simulink model "RB_KAIROS_ArmOnly"  (R2020b)
(part 5 of 17)

t11502 = (t10964.*(t263-t283-t310+t1265))./4.0;
t11506 = (t11023.*(t943-t1091))./4.0;
t11513 = (t3424.*t11023)./4.0;
t11514 = (t6158.*t10141)./4.0;
t11524 = (t6763.*t9828)./4.0;
t11527 = t14.*t6430.*t9828.*8.9697375e-1;
t11530 = -t11523;
t11536 = (t7797.*t9233)./4.0;
t11540 = t14.*t9828.*(t4540+t5.*(t2425-t2468)).*(-8.9697375e-1);
t11562 = t10141.*(-t2149+t2205+t693.*(t48-t349)+t784.*(t48-t349)).*(-1.0./2.0);
t11579 = ((t1492+t2158+t2696-t4727).*(-t3045-t3218+t3458+t3539+t3878+t8.*(t260+t468+t570+t2298).*1.666555))./2.0;
t11624 = t5235.*(t16.*(t30.*(t2425-t2468)+t68.*(t2425-t2468)).*1.666555+t8.*(t7.*(t4650+t34.*(t2425-t2468))+t47.*(t2425-t2468)).*1.666555).*(-1.0./4.0);
t11629 = (t5235.*(t16.*(t30.*(t2425-t2468)+t68.*(t2425-t2468)).*1.666555+t8.*(t7.*(t4650+t34.*(t2425-t2468))+t47.*(t2425-t2468)).*1.666555))./4.0;
t11645 = t10141.*(t624+t2511-t3502-t9.*t439.*4.252e-3).*(-1.0./2.0);
t11655 = (t4252.*t10964)./4.0;
t11657 = (t4251.*t10966)./4.0;
t11658 = t8.*t11633;
t11659 = t9.*t11633;
t11660 = t16.*t11633;
t11661 = t17.*t11633;
t11701 = t15.*t9236.*(t4542-t6448).*(-1.0./4.0);
t11713 = -t11709;
t11714 = (t15.*t9236.*(t6460-t35.*(t2425-t2468)))./4.0;
t11715 = t9263.*(t4542-t6448).*(-1.0./4.0);
t11738 = (t8213.*t9236)./4.0;
t11746 = t15.*t9278.*(t4542-t6448).*(-1.0./4.0);
t11747 = t8166.*(t1786+t2973-t7703-t5.*t12.*3.746479959e-1).*(-1.0./4.0);
t11753 = (t4569.*t10964)./4.0;
t11755 = (t15.*t9278.*(t4542-t6448))./4.0;
t11763 = (t4604.*t10966)./4.0;
t11764 = (t7247.*t9828)./4.0;
t11774 = (t7259.*t9830)./4.0;
t11776 = -t11767;
t11778 = ((t4542-t6448).*(t5457-t7520))./4.0;
t11780 = ((t4542-t6448).*(t5454-t7513))./4.0;
t11784 = t9236.*(t4654+t15.*(t4650+t34.*(t2425-t2468))).*(-1.0./4.0);
t11786 = t9269.*(-t1476-t1540+t2091+t2165+t2579+t8.*(t260+t468+t570+t2298)).*(-1.0./2.0);
t11787 = (t9236.*(t4654+t15.*(t4650+t34.*(t2425-t2468))))./4.0;
t11792 = t7434.*(-t3045-t3218+t3458+t3539+t3878+t8.*(t260+t468+t570+t2298).*1.666555).*(-1.0./2.0);
t11796 = t9828.*(t30.*(t2425-t2468).*3.587895+t68.*(t2425-t2468).*3.587895).*(-1.0./4.0);
t11797 = (t8191.*t9310)./2.0;
t11805 = (t8166.*t9325)./4.0;
t11808 = (t9828.*(t30.*(t2425-t2468).*3.587895+t68.*(t2425-t2468).*3.587895))./4.0;
t11818 = -t11809;
t11824 = t4884.*(t8963+t7.*(t5026+t5.*(t2959-t2967))).*(-1.0./4.0);
t11826 = (t6196.*t10441)./4.0;
t11829 = (t4884.*(t8963+t7.*(t5026+t5.*(t2959-t2967))))./4.0;
t11868 = (t6092.*t10501)./4.0;
t11871 = t8.*t11855;
t11905 = (t5713.*t10769)./4.0;
t11934 = (t7130.*t10141)./2.0;
t11937 = t7728+t9891;
t11947 = t10501.*(t985+t3399-t13.*t42.*1.01140545e-1-t7.*t223.*5.034347249e-2).*(-1.0./4.0);
t12016 = t5443.*(t8963+t7.*(t5026+t5.*(t2959-t2967))).*(-1.0./4.0);
t12021 = (t5443.*(t8963+t7.*(t5026+t5.*(t2959-t2967))))./4.0;
t12028 = (t8711.*t9285)./4.0;
t12030 = (t6302.*(t8643-t8.*(t30.*(t2425-t2468)+t68.*(t2425-t2468)).*7.35522e-1))./4.0;
t12034 = (t6190.*t10769)./4.0;
t12038 = (t4884.*t11266)./4.0;
t12042 = t2910+t2981+t3181+t3294+t3631+t5828+t7998;
t12050 = t2957+t3123+t3130+t3291+t3628+t5827+t8016;
t12072 = t14.*t6430.*t10501.*3.064865e-1;
t12077 = (t8711.*t9499)./4.0;
t12079 = t14.*t10501.*(t4540+t5.*(t2425-t2468)).*(-3.064865e-1);
t12083 = t6190.*(-t1053-t3327+t5081.*1.225946+t7731+t15.*t223.*1.4653732538e-2).*(-1.0./4.0);
t12084 = t14.*t10501.*(t4540+t5.*(t2425-t2468)).*3.064865e-1;
t12097 = (t6928.*t10501)./4.0;
t12100 = (t6175.*t10850)./4.0;
t12106 = (t6196.*t10858)./4.0;
t12150 = (t8437.*t9884)./4.0;
t12181 = t6196.*(t8963+t7.*(t5026+t5.*(t2959-t2967))).*(-1.0./4.0);
t12188 = (t6196.*(t8963+t7.*(t5026+t5.*(t2959-t2967))))./4.0;
t12191 = t10094.*(t4542-t6448).*(-1.0./4.0);
t12194 = (t10094.*(t4542-t6448))./4.0;
t12196 = (t5443.*t11266)./4.0;
t12197 = (t10094.*(t6460-t35.*(t2425-t2468)))./4.0;
t12211 = (t8166.*(-t1785+t2869+t2960+t5489+t5720+t4.*t13.*3.746479959e-1))./4.0;
t12217 = (t7245.*t10501)./2.0;
t12218 = (t7245.*t10501)./4.0;
t12228 = (t7246.*t10501)./4.0;
t12243 = (t6190.*t11023)./4.0;
t12249 = (t3266.*t11907)./4.0;
t12251 = t10501.*(t30.*(t2425-t2468).*1.225946+t68.*(t2425-t2468).*1.225946).*(-1.0./4.0);
t12260 = (t10501.*(t30.*(t2425-t2468).*1.225946+t68.*(t2425-t2468).*1.225946))./4.0;
t12266 = t2684+t2687+t11633;
t12269 = (t3362.*t11907)./4.0;
t12272 = (t11907.*(t923-t1076))./4.0;
t12297 = (t6.*t6430.*t10964)./4.0;
t12299 = (t6442.*t10966)./4.0;
t12302 = (t14.*t6430.*t10966)./4.0;
t12309 = t6.*t10964.*(t4540+t5.*(t2425-t2468)).*(-1.0./4.0);
t12313 = t14.*t10966.*(t4540+t5.*(t2425-t2468)).*(-1.0./4.0);
t12316 = (t6455.*t10964)./4.0;
t12317 = (t8711.*t9884)./4.0;
t12327 = t10966.*(t30.*(t2425-t2468)+t68.*(t2425-t2468)).*(-1.0./4.0);
t12335 = (t10966.*(t30.*(t2425-t2468)+t68.*(t2425-t2468)))./4.0;
t12343 = t10964.*(t4650+t34.*(t2425-t2468)).*(-1.0./4.0);
t12348 = (t10964.*(t4650+t34.*(t2425-t2468)))./4.0;
t12362 = t7.*t12049.*1.059103943995e-1;
t12366 = t15.*t12053.*1.059103943995e-1;
t12374 = (t8433.*t10141)./4.0;
t12377 = (t4884.*t11720)./4.0;
t12378 = t7.*t12163.*8.639075e-2;
t12380 = (t4265.*t11907)./4.0;
t12387 = t7677+t10566;
t12406 = (t8054.*t10441)./4.0;
t12418 = (t8628.*t10141)./4.0;
t12419 = (t8191.*t10398)./4.0;
t12454 = (t4774.*t11907)./4.0;
t12464 = t1313+t3488+t3541+t3612+t3867+t3922+t5822+t8013;
t12483 = (t5443.*t11720)./4.0;
t12486 = t12407.*(-7.35522e-1);
t12489 = t12407.*7.35522e-1;
t12528 = (t8438.*t10501)./4.0;
t12531 = (t9263.*t9828)./2.0;
t12535 = (t5277.*t11907)./4.0;
t12544 = ((t16.*(t30.*(t2425-t2468)+t68.*(t2425-t2468)).*1.666555+t8.*(t7.*(t4650+t34.*(t2425-t2468))+t47.*(t2425-t2468)).*1.666555).*(-t1476-t1540+t2091+t2165+t2579+t8.*(t260+t468+t570+t2298)))./4.0;
t12547 = t10759.*(t4542-t6448).*(-1.0./4.0);
t12548 = (t9325.*t9830)./2.0;
t12549 = (t10759.*(t4542-t6448))./4.0;
t12550 = t9828.*(t5454-t7513).*(-1.0./2.0);
t12552 = t10769.*(t4542-t6448).*(-1.0./4.0);
t12554 = (t9828.*(t5454-t7513))./2.0;
t12555 = (t10769.*(t4542-t6448))./4.0;
t12557 = (t8166.*t10754)./4.0;
t12558 = -t12553;
t12559 = (t10769.*(t6460-t35.*(t2425-t2468)))./4.0;
t12565 = (t8609.*t10501)./4.0;
t12568 = t12407.*(-3.867742437e-3);
t12573 = t15.*t12385.*1.059103943995e-1;
t12579 = t12407.*3.867742437e-3;
t12588 = t3188+t3333+t3627+t7833+t9323;
t12589 = t3125+t3336+t3630+t7835+t9331;
t12590 = t7.*t12396.*1.059103943995e-1;
t12593 = ((t4542-t6448).*(-t1053-t3327+t5081.*1.225946+t7731+t15.*t223.*1.4653732538e-2))./4.0;
t12601 = (t8689.*t10501)./4.0;
t12603 = (t5583.*t11907)./2.0;
t12604 = (t5583.*t11907)./4.0;
t12627 = (t5716.*t11907)./4.0;
t12654 = t8054.*(t8963+t7.*(t5026+t5.*(t2959-t2967))).*(-1.0./4.0);
t12664 = (t8054.*(t8963+t7.*(t5026+t5.*(t2959-t2967))))./4.0;
t12667 = t1267+t1955+t2202+t2562+t7690+t9892;
t12687 = (t5884.*t11907)./4.0;
t12711 = t10964.*(t4542-t6448).*(-1.0./4.0);
t12712 = t10966.*(t4542-t6448).*(-1.0./4.0);
t12715 = (t10966.*(t4542-t6448))./4.0;
t12718 = (t10964.*(t6460-t35.*(t2425-t2468)))./4.0;
t12719 = (t10966.*(t6460-t35.*(t2425-t2468)))./4.0;
t12725 = (t8166.*t10964)./4.0;
t12727 = (t8166.*t10966)./4.0;
t12730 = t8256.*(t8963+t7.*(t5026+t5.*(t2959-t2967))).*(-1.0./4.0);
t12734 = t11023.*(t4542-t6448).*(-1.0./4.0);
t12735 = (t8256.*(t8963+t7.*(t5026+t5.*(t2959-t2967))))./4.0;
t12737 = (t11023.*(t4542-t6448))./4.0;
t12740 = (t11023.*(t6460-t35.*(t2425-t2468)))./4.0;
t12749 = (t6114.*t11907)./4.0;
t12751 = t10964.*(t263+t1265-t7252-t5.*t12.*1.0442e-1).*(-1.0./2.0);
t12752 = (t8272.*t10966)./2.0;
t12756 = (t10964.*(t263+t1265-t7252-t5.*t12.*1.0442e-1))./2.0;
t12796 = t3182+t3565+t3934+t11848;
t12832 = (t14.*t6430.*t11907)./4.0;
t12836 = (t6442.*t11907)./4.0;
t12842 = t14.*t11907.*(t4540+t5.*(t2425-t2468)).*(-1.0./4.0);
t12844 = (t9236.*t10441)./4.0;
t12845 = (t14.*t11907.*(t4540+t5.*(t2425-t2468)))./4.0;
t12859 = t11907.*(t30.*(t2425-t2468)+t68.*(t2425-t2468)).*(-1.0./4.0);
t12865 = (t11907.*(t30.*(t2425-t2468)+t68.*(t2425-t2468)))./4.0;
t12866 = t206+t446+t2571+t2622+t2736+t2770+t11671;
t12887 = (t5634.*t12163)./4.0;
t12890 = (t6175.*t12049)./4.0;
t12898 = t1315+t3619+t3932+t3973+t7832+t9327;
t12900 = (t6196.*t12053)./4.0;
t12914 = -t12911;
t12916 = (t10964.*(-t262+t1056+t1250+t5078+t5282+t4.*t13.*1.0442e-1))./2.0;
t12917 = (t9828.*t10094)./2.0;
t12919 = -t12915;
t12924 = (t8697.*t10966)./2.0;
t12926 = (t8256.*t11266)./4.0;
t12939 = (t5216.*t12385)./4.0;
t12948 = t10501.*(t5457-t7520).*(-1.0./2.0);
t12955 = (t5218.*t12396)./4.0;
t12996 = ((t16.*(t30.*(t2425-t2468)+t68.*(t2425-t2468))+t8.*(t7.*(t4650+t34.*(t2425-t2468))+t47.*(t2425-t2468))).*(-t3045-t3218+t3458+t3539+t3878+t8.*(t260+t468+t570+t2298).*1.666555))./4.0;
t13011 = (t8931.*t10964)./2.0;
t13018 = t10966.*(t5027-t7134).*(-1.0./2.0);
t13023 = (t10966.*(t5027-t7134))./2.0;
t13060 = (t5635.*t12385)./4.0;
t13083 = (t5646.*t12396)./4.0;
t13137 = (t9236.*t10858)./4.0;
t13150 = t232+t429+t2506+t2524+t3657+t3669+t7690+t9892;
t13163 = (t6046.*t12392)./4.0;
t13169 = (t4024.*t12792)./4.0;
t13183 = t9278.*(t8963+t7.*(t5026+t5.*(t2959-t2967))).*(-1.0./4.0);
t13187 = (t9278.*(t8963+t7.*(t5026+t5.*(t2959-t2967))))./4.0;
t13191 = -t13190;
t13199 = (t12163.*(t921+t1317-t5853))./4.0;
t13215 = (t7039.*t12185)./4.0;
t13219 = t16.*t13019.*4.38178973375e-3;
t13236 = t7.*t13140.*8.639075e-2;
t13248 = (t9828.*t10759)./2.0;
t13262 = (t6552.*t12385)./4.0;
t13264 = t11907.*(t4542-t6448).*(-1.0./4.0);
t13268 = (t11907.*(t4542-t6448))./4.0;
t13271 = (t11907.*(t6460-t35.*(t2425-t2468)))./4.0;
t13275 = (t6546.*t12396)./4.0;
t13281 = (t8166.*t11907)./4.0;
t13311 = (t9236.*t11247)./4.0;
t13340 = (t5235.*t12792)./4.0;
t13341 = (t9685.*t10964)./2.0;
t13351 = (t2980.*t13140)./4.0;
t13353 = (t9686.*t10966)./2.0;
t13358 = (t8050.*t12049)./4.0;
t13365 = (t8054.*t12053)./4.0;
t13396 = (t7113.*t12385)./4.0;
t13406 = (t7124.*t12396)./4.0;
t13446 = (t4064.*t13140)./4.0;
t13545 = t11907.*(t5027-t7134).*(-1.0./2.0);
t13578 = t1604+t2211+t3880+t3884+t3988+t4006+t11862;
t13588 = (t4837.*t13140)./4.0;
t13592 = t7797.*(t8329+t17.*(t16.*(t30.*(t2425-t2468)+t68.*(t2425-t2468))+t8.*(t7.*(t4650+t34.*(t2425-t2468))+t47.*(t2425-t2468)))).*(-1.0./4.0);
t13595 = (t7797.*(t8329+t17.*(t16.*(t30.*(t2425-t2468)+t68.*(t2425-t2468))+t8.*(t7.*(t4650+t34.*(t2425-t2468))+t47.*(t2425-t2468)))))./4.0;
t13604 = (t9278.*t11720)./4.0;
t13605 = (t921+t1317-t5853).*(t3129+t3384+t3574+t7846+t9332).*(-1.0./4.0);
t13606 = t12385.*(t2437+t2648+t3129+t3384+t3574).*(-1.0./4.0);
t13617 = (t10501.*t10769)./2.0;
t13629 = t3098+t3211+t3241+t3678+t8102+t10798;
t13630 = (t5095.*t13140)./4.0;
t13631 = (t8047.*t12385)./4.0;
t13633 = (t8044.*t12385)./4.0;
t13636 = (t8053.*t12396)./4.0;
t13637 = (t8065.*t12396)./4.0;
t13650 = t10501.*(-t1053-t3327+t5081.*1.225946+t7731+t15.*t223.*1.4653732538e-2).*(-1.0./2.0);
t13651 = (t10501.*(-t1053-t3327+t5081.*1.225946+t7731+t15.*t223.*1.4653732538e-2))./2.0;
t13664 = (t8285.*t12385)./4.0;
t13689 = (t8310.*t12396)./4.0;
t13706 = (t9285.*t11907)./2.0;
t13732 = (t6069.*t13019)./4.0;
t13738 = t16.*(t3098+t3211-t3221+t3678+t8102+t10798).*2.62925e-3;
t13739 = t7.*t12385.*(t4542-t6448).*(-3.064865e-1);
t13745 = t7.*t12385.*(t4542-t6448).*3.064865e-1;
t13748 = t7.*t12385.*(t6460-t35.*(t2425-t2468)).*3.064865e-1;
t13749 = (t5648.*t13140)./4.0;
t13755 = t15.*t12396.*(t4542-t6448).*(-3.064865e-1);
t13758 = t15.*t12396.*(t6460-t35.*(t2425-t2468)).*3.064865e-1;
t13774 = (t9499.*t11907)./2.0;
t13775 = (t10501.*t11023)./2.0;
t13828 = (t13313.*(t2904-t2927))./4.0;
t13833 = (t9236.*t12053)./4.0;
t13834 = (t5853.*t13140)./4.0;
t13837 = (t5860.*t13140)./4.0;
t13848 = (t5999.*t13140)./4.0;
t13875 = t12396.*(t5150-t6911).*(-1.0./4.0);
t13882 = t12385.*(t7.*(t4650+t34.*(t2425-t2468)).*1.225946+t47.*(t2425-t2468).*1.225946).*(-1.0./4.0);
t13884 = (t12385.*(t7.*(t4650+t34.*(t2425-t2468)).*1.225946+t47.*(t2425-t2468).*1.225946))./4.0;
t13887 = (t8922.*t12396)./4.0;
t13891 = (t5365.*t13313)./4.0;
t13941 = (t9884.*t11907)./2.0;
t13964 = (t4021.*(t3098+t3211-t3221+t3678+t8102+t10798))./4.0;
t14015 = (t9209.*t12385)./4.0;
t14018 = (t6988.*t13140)./4.0;
t14023 = t12792.*(-t1476-t1540+t2091+t2165+t2579+t8.*(t260+t468+t570+t2298)).*(-1.0./4.0);
t14035 = t1566+t1867+t3700+t3703+t4023+t4038+t8101+t10794;
t14107 = t12392.*(-t3045-t3218+t3458+t3539+t3878+t8.*(t260+t468+t570+t2298).*1.666555).*(-1.0./4.0);
t14155 = t15.*t13140.*(t4542-t6448).*(-1.0./4.0);
t14162 = (t15.*t13140.*(t6460-t35.*(t2425-t2468)))./4.0;
t14164 = (t8213.*t13140)./4.0;
t14180 = t13140.*(t4654+t15.*(t4650+t34.*(t2425-t2468))).*(-1.0./4.0);
t14182 = (t13140.*(t4654+t15.*(t4650+t34.*(t2425-t2468))))./4.0;
t14304 = (t8477.*t13313)./4.0;
t14670 = (t10441.*t13140)./2.0;
t14710 = (t10141.*t13313)./4.0;
t14801 = (t10858.*t13140)./2.0;
t14821 = t1763+t1824+t2316+t2415+t2791+t10569+t12397;
t14823 = t1791+t1818+t2335+t2387+t2789+t10567+t12407;
t14845 = t13140.*(t8963+t7.*(t5026+t5.*(t2959-t2967))).*(-1.0./2.0);
t14858 = (t12163.*t12385)./2.0;
t14865 = (t12185.*t12396)./2.0;
t14914 = (t11247.*t13140)./2.0;
t15037 = t12385.*(t3129+t3384+t3574+t7846+t9332).*(-1.0./2.0);
t15040 = (t12385.*(t3129+t3384+t3574+t7846+t9332))./2.0;
t15142 = (t12053.*t13140)./2.0;
t1967 = -t1918;
t2474 = t9.*t2405;
t2480 = t17.*t2405;
t3308 = t543+t1912;
t3392 = t1918.*(-1.2516e-2);
t3448 = t1912.*6.1597e-2;
t3452 = t1918.*6.1597e-2;
t3569 = t1918.*(-4.28e-4);
t3572 = t1918.*(-1.0517e-2);
t3652 = t1918.*(-7.41e-4);
t3845 = t2549.*(-7.35522e-1);
t3893 = t2549.*7.35522e-1;
t4321 = t1912.*4.5305948634e-2;
t4324 = t1918.*4.5305948634e-2;
t4346 = t1912.*3.127439544e-3;
t4349 = t1918.*3.127439544e-3;
t4350 = t1912.*7.735484874e-3;
t4355 = t1918.*7.735484874e-3;
t4666 = t2549.*(-3.127439544e-3);
t4713 = -t4682;
t4769 = -t4744;
t4814 = -t4771;
t4826 = -t4808;
t4956 = -t4947;
t4980 = t1918.*1.672482661783778e-3;
t4981 = t1912.*5.48359106408232e-4;
t5111 = t4528.*7.35522e-1;
t5113 = t4529.*7.35522e-1;
t5127 = -t5106;
t5147 = -t5128;
t5166 = -t5140;
t5184 = -t5160;
t5199 = t4697.*7.35522e-1;
t5220 = t4693.*7.35522e-1;
t5226 = -t5205;
t5236 = t3239.*(t1918+t9.*(t71-t391)).*(-1.0./4.0);
t5238 = t3324.*(t689-t740).*(-1.0./4.0);
t5242 = (t3239.*(t1918+t9.*(t71-t391)))./4.0;
t5243 = t4771.*7.35522e-1;
t5245 = (t3324.*(t689-t740))./4.0;
t5250 = t3280.*(t1918+t9.*(t71-t391)).*(-1.0./4.0);
t5255 = t4767.*7.35522e-1;
t5260 = (t3280.*(t1918+t9.*(t71-t391)))./4.0;
t5296 = t3447.*(t1918+t9.*(t71-t391)).*(-1.0./4.0);
t5305 = (t3447.*(t1918+t9.*(t71-t391)))./4.0;
t5325 = -t5315;
t5343 = -t5332;
t5348 = -t5338;
t5353 = -t5342;
t5359 = t9.*t5337;
t5360 = t17.*t5337;
t5384 = t9.*t5357;
t5386 = t17.*t5357;
t5395 = -t9.*(t1474+t4743);
t5396 = -t17.*(t1474+t4743);
t5415 = t17.*(t1474+t4743);
t5417 = -t5409;
t5558 = t4529.*3.867742437e-3;
t5567 = -t5549;
t5570 = t4528.*1.563719772e-3;
t5607 = -t5584;
t5608 = -t5585;
t5633 = -t5618;
t5643 = t4693.*3.867742437e-3;
t5658 = t4697.*1.563719772e-3;
t5664 = -t5651;
t5676 = -t5662;
t5684 = -t5673;
t5685 = -t5675;
t5687 = t4771.*3.867742437e-3;
t5698 = t4767.*1.563719772e-3;
t5700 = -t5686;
t5727 = -t5717;
t5752 = -t5738;
t5766 = t4410.*(t1918+t9.*(t71-t391)).*(-1.0./4.0);
t5770 = -t5754;
t5773 = (t4410.*(t1918+t9.*(t71-t391)))./4.0;
t5775 = -t5768;
t5789 = (t3324.*t4515)./4.0;
t5801 = t4499.*(t1918+t9.*(t71-t391)).*(-1.0./4.0);
t5805 = -t5792;
t5814 = (t4499.*(t1918+t9.*(t71-t391)))./4.0;
t5820 = t9.*(t1474+t4743).*(-7.35522e-1);
t5882 = -t5871;
t5893 = t4701.*(t1918+t9.*(t71-t391)).*(-1.0./4.0);
t5908 = (t4701.*(t1918+t9.*(t71-t391)))./4.0;
t6011 = -t5994;
t6204 = t8.*t5234.*4.38178973375e-3;
t6218 = -t6206;
t6251 = t2041+t2102+t2636+t2643;
t6341 = (t8.*t6250)./4.0;
t6378 = (t15.*t16.*t6250)./4.0;
t6380 = (t16.*t6271)./4.0;
t6384 = t9.*(t1474+t4743).*(-1.563719772e-3);
t6389 = -t6370;
t6394 = -t6375;
t6402 = t9.*(t1474+t4743).*1.563719772e-3;
t6405 = (t8.*t15.*t6271)./4.0;
t6465 = -t6457;
t6480 = (t227.*t6271)./4.0;
t6482 = (t323.*t6250)./4.0;
t6486 = t5291.*(t1918+t9.*(t71-t391)).*(-1.0./4.0);
t6488 = t8.*t5915.*2.62925e-3;
t6493 = (t5291.*(t1918+t9.*(t71-t391)))./4.0;
t6496 = -t6489;
t6541 = -t6528;
t6568 = -t6559;
t6572 = (t439.*t6250)./4.0;
t6603 = -t6595;
t6608 = t6271.*(t48-t349).*(-1.0./4.0);
t6618 = (t6271.*(t48-t349))./4.0;
t6623 = t17.*t5719.*1.13264871585e-2;
t6640 = -t6630;
t6664 = -t6652;
t6668 = -t6660;
t6688 = -t6680;
t6696 = t5553.*(t1918+t9.*(t71-t391)).*(-1.0./4.0);
t6707 = -t6691;
t6712 = -t6692;
t6717 = (t5553.*(t1918+t9.*(t71-t391)))./4.0;
t6719 = (t15.*t16.*t6634)./4.0;
t6721 = -t6701;
t6725 = -t6708;
t6731 = -t6714;
t6740 = t5609.*(t1918+t9.*(t71-t391)).*(-1.0./4.0);
t6744 = t1999+t2168+t2188+t4511;
t6751 = -t6738;
t6769 = -t6757;
t6775 = -t6768;
t6782 = -t6771;
t6787 = t6.*t6757;
t6792 = -t6779;
t6811 = t1067+t1659+t5719;
t6812 = -t6786;
t6867 = -t6829;
t6875 = (t1840.*t6271)./2.0;
t6878 = t6250.*(t348-t525).*(-1.0./2.0);
t6884 = t2943+t5915;
t6887 = -t6853;
t6891 = -t6865;
t6899 = -t6874;
t6901 = (t6250.*(t348-t525))./2.0;
t6903 = -t6880;
t6904 = -t6882;
t6914 = -t6888;
t6925 = -t6896;
t6933 = -t6905;
t6938 = t2017+t2639+t5337;
t6940 = (t323.*t6634)./4.0;
t6947 = -t6922;
t6954 = -t6929;
t6963 = -t6943;
t6964 = t5763.*(t1918+t9.*(t71-t391)).*(-1.0./4.0);
t6968 = -t6953;
t6980 = (t5763.*(t1918+t9.*(t71-t391)))./4.0;
t6990 = (t17.*t6844)./2.0;
t6996 = (t8.*t6893)./4.0;
t7006 = (t3324.*t5837)./4.0;
t7011 = (t9.*t16.*t6844)./4.0;
t7017 = -t7000;
t7021 = -t7005;
t7027 = (t15.*t16.*t6893)./4.0;
t7032 = -t7012;
t7035 = -t7014;
t7046 = t5834.*(t1918+t9.*(t71-t391)).*(-1.0./4.0);
t7058 = (t5834.*(t1918+t9.*(t71-t391)))./4.0;
t7067 = (t439.*t6634)./2.0;
t7078 = (t9.*t7003)./2.0;
t7101 = -t7091;
t7103 = (t16.*t17.*t7003)./4.0;
t7125 = t17.*(t1912.*(-4.28e-4)+t3337+t587.*(t71-t391)+t689.*(t71-t391)).*(-1.0./4.0);
t7128 = t2676+t2706+t3473+t3497;
t7135 = (t17.*(t1912.*(-4.28e-4)+t3337+t587.*(t71-t391)+t689.*(t71-t391)))./4.0;
t7139 = t9.*t16.*(t1912.*(-4.28e-4)+t3337+t587.*(t71-t391)+t689.*(t71-t391)).*(-1.0./4.0);
t7140 = (t325.*t6844)./4.0;
t7141 = t2693+t2704+t3499+t3587;
t7148 = (t9.*t16.*(t1912.*(-4.28e-4)+t3337+t587.*(t71-t391)+t689.*(t71-t391)))./4.0;
t7158 = t5990.*(t1918+t9.*(t71-t391)).*(-1.0./4.0);
t7160 = (t323.*t6893)./4.0;
t7163 = -t7147;
t7169 = (t5990.*(t1918+t9.*(t71-t391)))./4.0;
t7183 = t6041.*(t1918+t9.*(t71-t391)).*(-1.0./4.0);
t7185 = t9.*(t1912.*(-1.0027e-2)+t2709+t3492+t751.*(t71-t391)).*(-1.0./4.0);
t7189 = (t229.*t7003)./4.0;
t7190 = (t9.*(t1912.*(-1.0027e-2)+t2709+t3492+t751.*(t71-t391)))./4.0;
t7199 = t16.*t17.*(t1912.*(-1.0027e-2)+t2709+t3492+t751.*(t71-t391)).*(-1.0./4.0);
t7207 = (t16.*t17.*(t1912.*(-1.0027e-2)+t2709+t3492+t751.*(t71-t391)))./4.0;
t7232 = (t440.*t6844)./4.0;
t7243 = (t439.*t6893)./4.0;
t7257 = t325.*(t1912.*(-4.28e-4)+t3337+t587.*(t71-t391)+t689.*(t71-t391)).*(-1.0./4.0);
t7269 = (t325.*(t1912.*(-4.28e-4)+t3337+t587.*(t71-t391)+t689.*(t71-t391)))./4.0;
t7285 = (t5069.*t5234)./4.0;
t7299 = -t7286;
t7308 = t229.*(t1912.*(-1.0027e-2)+t2709+t3492+t751.*(t71-t391)).*(-1.0./4.0);
t7322 = -t7300;
t7327 = (t229.*(t1912.*(-1.0027e-2)+t2709+t3492+t751.*(t71-t391)))./4.0;
t7333 = (t4024.*t5915)./4.0;
t7347 = -t7324;
t7353 = t6634.*(t348-t525).*(-1.0./4.0);
t7354 = -t7331;
t7356 = -t7334;
t7370 = t7003.*(t79-t358).*(-1.0./4.0);
t7375 = (t6634.*(t348-t525))./4.0;
t7382 = (t7003.*(t79-t358))./4.0;
t7384 = t6276.*(t1918+t9.*(t71-t391)).*(-1.0./4.0);
t7391 = t845+t1667+t1988+t2498+t4630;
t7397 = t440.*(t1912.*(-4.28e-4)+t3337+t587.*(t71-t391)+t689.*(t71-t391)).*(-1.0./4.0);
t7409 = t16.*t6872.*2.62925e-3;
t7411 = (t440.*(t1912.*(-4.28e-4)+t3337+t587.*(t71-t391)+t689.*(t71-t391)))./4.0;
t7430 = -t7419;
t7438 = t2510+t2628+t2665+t2695+t2735;
t7440 = t1236+t2028+t2063+t2135+t2656+t2666;
t7455 = (t17.*t7396)./4.0;
t7465 = -t7456;
t7467 = ((t79-t358).*(t1912.*(-1.0027e-2)+t2709+t3492+t751.*(t71-t391)))./4.0;
t7471 = (t9.*t16.*t7396)./4.0;
t7480 = -t7473;
t7486 = t1362+t1985+t2170+t2302+t2611+t2692;
t7490 = t2597+t2634+t2703+t2718+t2732;
t7497 = t1813+t1968+t2178+t2279+t2592+t2689;
t7510 = (t15.*t7458)./4.0;
t7525 = -t7514;
t7534 = (t7.*t14.*t7458)./4.0;
t7537 = (t9.*t7469)./4.0;
t7541 = t6893.*(t348-t525).*(-1.0./2.0);
t7549 = t6844.*(t395+t9.*(t48-t349)).*(-1.0./4.0);
t7550 = t6.*t15.*t7458.*(-1.0./4.0);
t7552 = (t8.*t7485)./2.0;
t7556 = (t6893.*(t348-t525))./2.0;
t7565 = (t6844.*(t395+t9.*(t48-t349)))./4.0;
t7566 = (t14.*t43.*t7458)./4.0;
t7570 = (t16.*t17.*t7469)./4.0;
t7575 = -t7557;
t7582 = (t15.*t16.*t7485)./4.0;
t7586 = t8.*t7557;
t7601 = -t7587;
t7611 = (t325.*t7396)./4.0;
t7617 = -t7598;
t7636 = -t7618;
t7640 = (t1907.*t7003)./4.0;
t7654 = t3625+t3660+t5337;
t7689 = (t5234.*t5430)./4.0;
t7691 = (t225.*t7458)./4.0;
t7692 = (t226.*t7458)./4.0;
t7721 = -t7701;
t7722 = -t7702;
t7725 = (t15.*t223.*t7458)./2.0;
t7730 = (t229.*t7469)./4.0;
t7738 = t9.*t6761.*1.13264871585e-2;
t7744 = ((t395+t9.*(t48-t349)).*(t1912.*(-4.28e-4)+t3337+t587.*(t71-t391)+t689.*(t71-t391)))./4.0;
t7757 = -t7747;
t7767 = (t323.*t7485)./4.0;
t7770 = (t2520.*t6872)./4.0;
t7772 = -t7758;
t7773 = -t7759;
t7776 = (t403.*t7458)./2.0;
t7782 = t323.*t7557;
t7785 = t1907.*(t1912.*(-1.0027e-2)+t2709+t3492+t751.*(t71-t391)).*(-1.0./4.0);
t7795 = t6615.*(t1918+t9.*(t71-t391)).*(-1.0./4.0);
t7806 = -t7791;
t7813 = -t7794;
t7814 = (t6615.*(t1918+t9.*(t71-t391)))./4.0;
t7817 = t12.*t7791;
t7818 = -t7803;
t7822 = t266+t464+t555+t1952+t2001+t2288+t2619+t2624;
t7829 = t6629.*(t1918+t9.*(t71-t391)).*(-1.0./4.0);
t7843 = (t6629.*(t1918+t9.*(t71-t391)))./4.0;
t7849 = (t454.*t7458)./2.0;
t7856 = t2490+t2746+t2962+t3127+t3346;
t7870 = t8.*t6957.*4.38178973375e-3;
t7872 = (t470.*t7458)./2.0;
t7878 = (t3324.*t6687)./4.0;
t7890 = (t439.*t7485)./4.0;
t7897 = -t7877;
t7912 = -t7900;
t7913 = t2462+t2899+t2971+t3056+t3506;
t7916 = -t7905;
t7933 = -t7920;
t7934 = -t7922;
t7948 = -t7936;
t7961 = -t7947;
t7969 = t6758.*(t1918+t9.*(t71-t391)).*(-1.0./4.0);
t7981 = (t6758.*(t1918+t9.*(t71-t391)))./4.0;
t7993 = t8.*t7079.*4.38178973375e-3;
t7994 = -t7984;
t8010 = t8.*t7105.*4.38178973375e-3;
t8028 = t16.*t7116.*4.38178973375e-3;
t8063 = t141+t234+t602+t1995+t2020+t2573+t2659+t3348;
t8071 = (t4884.*t6193)./4.0;
t8076 = -t8059;
t8099 = -t8080;
t8122 = t6983.*(t1918+t9.*(t71-t391)).*(-1.0./4.0);
t8123 = t7396.*(t395+t9.*(t48-t349)).*(-1.0./2.0);
t8128 = t7.*t8077;
t8129 = t8.*t8077;
t8131 = t15.*t8077;
t8132 = t16.*t8077;
t8133 = -t8115;
t8135 = t7003.*(t1918+t9.*(t71-t391)).*(-1.0./2.0);
t8138 = -t8121;
t8139 = (t6983.*(t1918+t9.*(t71-t391)))./4.0;
t8151 = -t8136;
t8168 = (t5234.*t5919)./2.0;
t8179 = (t5234.*t5914)./2.0;
t8182 = (t5235.*t5915)./2.0;
t8185 = t7.*t8158;
t8186 = t7.*t8160;
t8190 = -t8170;
t8198 = (t3780.*t6872)./4.0;
t8199 = -t8180;
t8200 = -t8181;
t8202 = -t8183;
t8215 = (t1907.*t7469)./2.0;
t8227 = t1439+t2078+t6957;
t8234 = t7485.*(t348-t525).*(-1.0./2.0);
t8239 = (t5433.*t5719)./4.0;
t8246 = (t7485.*(t348-t525))./2.0;
t8253 = t1463+t1474+t2000+t2268+t2570+t4743;
t8254 = -t8219;
t8269 = -t8238;
t8277 = -t8263;
t8284 = t7557.*(t348-t525);
t8286 = ((t1918+t9.*(t71-t391)).*(t1912.*(-1.0027e-2)+t2709+t3492+t751.*(t71-t391)))./2.0;
t8288 = -t8275;
t8292 = -t8266;
t8300 = -t8290;
t8308 = (t5434.*t5782)./4.0;
t8325 = -t8319;
t8334 = t9.*t7828.*1.539925e-2;
t8361 = (t4300.*t6761)./4.0;
t8385 = -t8376;
t8403 = -t8390;
t8409 = -t8396;
t8446 = t15.*t7937.*8.639075e-2;
t8474 = -t8463;
t8489 = -t8476;
t8498 = -t8483;
t8521 = (t4509.*t6872)./2.0;
t8530 = t2010+t2531+t2638+t2709+t3334+t3492;
t8531 = (t4514.*t6872)./2.0;
t8540 = ((t1918+t9.*(t71-t391)).*(t1528+t1966+t2026-t2172+t587.*(t48-t349)+t689.*(t48-t349)))./4.0;
t8553 = t8220.*(-7.35522e-1);
t8554 = t8222.*(-7.35522e-1);
t8558 = t7.*t8538;
t8561 = t8220.*(-1.666555);
t8562 = t3237+t3363+t3872+t5215;
t8563 = t3218+t3412+t3913+t5211;
t8568 = t8220.*7.35522e-1;
t8569 = t8222.*7.35522e-1;
t8571 = t8220.*1.666555;
t8572 = -t8567;
t8574 = t8229.*1.225946;
t8576 = t8238.*7.35522e-1;
t8578 = t8237.*1.666555;
t8579 = (t17.*t8506)./4.0;
t8580 = (t5443.*t6193)./4.0;
t8582 = t8219.*7.35522e-1;
t8584 = t8238.*1.666555;
t8586 = t8226.*7.35522e-1;
t8587 = t8218.*1.666555;
t8589 = t8219.*1.666555;
t8590 = (t3324.*t7475)./2.0;
t8591 = t8225.*1.666555;
t8592 = t8226.*1.666555;
t8594 = t8229.*1.666555;
t8595 = t8230.*1.666555;
t8597 = t8225.*1.225946;
t8600 = t3116+t3486+t3963+t5232;
t8604 = -t8583;
t8607 = t7469.*(t1918+t9.*(t71-t391)).*(-1.0./4.0);
t8610 = t8266.*7.35522e-1;
t8611 = (t9.*t16.*t8506)./4.0;
t8612 = t8270.*7.35522e-1;
t8613 = t3157+t3590+t3937+t5230;
t8621 = ((t1918+t9.*(t71-t391)).*(t578.*4.28e-4+t2566-t2597+t905.*(t71-t391)+t1021.*(t71-t391)))./2.0;
t8622 = t2237+t2657+t2670+t2700+t3483+t3520;
t8625 = (t8.*t8552)./4.0;
t8639 = (t15.*t16.*t8552)./4.0;
t8641 = t16.*(t1912.*(-1.196e-3)-t1942+t2518+t3589+t696.*(t71-t391)+t891.*(t71-t391)).*(-1.0./4.0);
t8642 = t9.*t7799.*1.13264871585e-2;
t8644 = -t8636;
t8648 = (t16.*(t1912.*(-1.196e-3)-t1942+t2518+t3589+t696.*(t71-t391)+t891.*(t71-t391)))./4.0;
t8656 = t8.*t15.*(t1912.*(-1.196e-3)-t1942+t2518+t3589+t696.*(t71-t391)+t891.*(t71-t391)).*(-1.0./4.0);
t8659 = -t8652;
t8663 = (t8.*t15.*(t1912.*(-1.196e-3)-t1942+t2518+t3589+t696.*(t71-t391)+t891.*(t71-t391)))./4.0;
t8668 = t15.*t44.*(t1912.*(-1.196e-3)-t1942+t2518+t3589+t696.*(t71-t391)+t891.*(t71-t391)).*(-1.0./4.0);
t8669 = -t8664;
t8673 = (t15.*t44.*(t1912.*(-1.196e-3)-t1942+t2518+t3589+t696.*(t71-t391)+t891.*(t71-t391)))./4.0;
t8684 = (t325.*t8506)./4.0;
t8695 = (t323.*t8552)./4.0;
t8698 = t227.*(t1912.*(-1.196e-3)-t1942+t2518+t3589+t696.*(t71-t391)+t891.*(t71-t391)).*(-1.0./4.0);
t8699 = t228.*(t1912.*(-1.196e-3)-t1942+t2518+t3589+t696.*(t71-t391)+t891.*(t71-t391)).*(-1.0./4.0);
t8704 = -t8696;
t8705 = (t228.*(t1912.*(-1.196e-3)-t1942+t2518+t3589+t696.*(t71-t391)+t891.*(t71-t391)))./4.0;
t8708 = -t8702;
t8713 = t2588+t3414+t3525+t3532+t4479;
t8715 = (t3249.*t7815)./4.0;
t8717 = t17.*t7982.*1.13264871585e-2;
t8718 = -t8712;
t8719 = t9.*t7987.*1.13264871585e-2;
t8727 = (t440.*t8506)./4.0;
t8731 = t404.*(t1912.*(-1.196e-3)-t1942+t2518+t3589+t696.*(t71-t391)+t891.*(t71-t391)).*(-1.0./4.0);
t8737 = (t404.*(t1912.*(-1.196e-3)-t1942+t2518+t3589+t696.*(t71-t391)+t891.*(t71-t391)))./4.0;
t8740 = (t5234.*t6681)./2.0;
t8741 = t5112+t6805;
t8742 = t5126+t6794;
t8746 = -t8738;
t8747 = (t5050.*t6872)./2.0;
t8750 = t5131+t6808;
t8751 = t5142+t6795;
t8756 = -t8748;
t8759 = (t439.*t8552)./2.0;
t8770 = -t8760;
t8776 = t6.*t8077.*2.46255173325e-2;
t8777 = ((t1918+t9.*(t71-t391)).*(t618.*4.28e-4-t1841-t2389+t2400-t2414+t17.*(t113-t409).*1.0027e-2))./2.0;
t8783 = t9.*t8460.*1.539925e-2;
t8787 = t17.*t8464.*1.539925e-2;
t8788 = -t8773;
t8801 = ((t48-t349).*(t1912.*(-1.196e-3)-t1942+t2518+t3589+t696.*(t71-t391)+t891.*(t71-t391)))./4.0;
t8813 = -t8800;
t8822 = -t8805;
t8832 = ((t60-t394).*(t1912.*(-1.196e-3)-t1942+t2518+t3589+t696.*(t71-t391)+t891.*(t71-t391)))./4.0;
t8835 = -t8816;
t8838 = -t8821;
t8845 = t8222.*(-3.867742437e-3);
t8848 = t8220.*(-5.01208083475e-2);
t8851 = (t4024.*t7646)./4.0;
t8854 = -t8833;
t8863 = t8222.*3.867742437e-3;
t8867 = t8220.*5.01208083475e-2;
t8870 = (t3738.*t7828)./4.0;
t8876 = t8229.*7.326866269e-3;
t8880 = (t3752.*t7815)./4.0;
t8882 = t8238.*5.01208083475e-2;
t8889 = t8225.*2.5171736245e-2;
t8890 = t8219.*5.01208083475e-2;
t8891 = t539.*(t1912.*(-1.196e-3)-t1942+t2518+t3589+t696.*(t71-t391)+t891.*(t71-t391)).*(-1.0./2.0);
t8893 = t8226.*5.01208083475e-2;
t8894 = (t16.*(t71-t391).*(t1912.*(-1.196e-3)-t1942+t2518+t3589+t696.*(t71-t391)+t891.*(t71-t391)))./2.0;
t8897 = t8237.*1.17633784675e-2;
t8900 = t8218.*1.17633784675e-2;
t8901 = t16.*t8178.*4.38178973375e-3;
t8902 = -t8878;
t8910 = -t8886;
t8911 = t8230.*1.17633784675e-2;
t8918 = t8266.*3.867742437e-3;
t8920 = -t8907;
t8923 = t8270.*1.563719772e-3;
t8930 = (t3743.*t7901)./4.0;
t8933 = (t5069.*t7079)./4.0;
t8958 = -t8949;
t8961 = t604.*(t1912.*(-1.196e-3)-t1942+t2518+t3589+t696.*(t71-t391)+t891.*(t71-t391)).*(-1.0./2.0);
t8972 = (t604.*(t1912.*(-1.196e-3)-t1942+t2518+t3589+t696.*(t71-t391)+t891.*(t71-t391)))./2.0;
t8973 = (t5083.*t7116)./4.0;
t8975 = -t8967;
t8990 = t8055.*(t1918+t9.*(t71-t391)).*(-1.0./2.0);
t8993 = -t8989;
t8994 = (t8055.*(t1918+t9.*(t71-t391)))./2.0;
t8997 = -t8991;
t8999 = t1431+t1625+t1974+t2250+t2545+t3509+t4528;
t9001 = t1217+t1680+t1977+t2204+t2596+t3624+t4529;
t9005 = t8506.*(t395+t9.*(t48-t349)).*(-1.0./2.0);
t9008 = (t8506.*(t395+t9.*(t48-t349)))./2.0;
t9009 = t1840.*(t1912.*(-1.196e-3)-t1942+t2518+t3589+t696.*(t71-t391)+t891.*(t71-t391)).*(-1.0./2.0);
t9010 = (t5448.*t6761)./4.0;
t9012 = t8552.*(t348-t525).*(-1.0./2.0);
t9014 = (t8552.*(t348-t525))./2.0;
t9022 = ((t386+t16.*(t69-t347)).*(t1912.*(-1.196e-3)-t1942+t2518+t3589+t696.*(t71-t391)+t891.*(t71-t391)))./2.0;
t9023 = -t9018;
t9029 = -t9024;
t9034 = t16.*t8709.*2.62925e-3;
t9044 = (t4286.*t7937)./4.0;
t9050 = t3002+t3169+t3373+t3797+t5130;
t9058 = t14.*(t5124-t6795).*(-6.8635e-3);
t9063 = t14.*(t5124-t6795).*6.8635e-3;
t9077 = (t5430.*t7079)./4.0;
t9078 = t14.*t8780.*6.8635e-3;
t9084 = t6.*t8794.*6.8635e-3;
t9107 = (t5441.*t7116)./4.0;
t9111 = t7.*t8802.*8.639075e-2;
t9124 = -t9115;
t9129 = -t9117;
t9131 = -t9120;
t9134 = -t9125;
t9136 = -t9128;
t9154 = -t9149;
t9164 = (t3489.*t8497)./4.0;
t9167 = t713+t2602+t2685+t2719+t4703+t4767;
t9173 = (t5365.*t7336)./4.0;
t9185 = t2905+t3165+t7828;
t9188 = -t9183;
t9191 = -t9189;
t9192 = (t4884.*t7875)./4.0;
t9202 = (t1918+t9.*(t71-t391)).*(t1961.*4.28e-4+t1965.*1.0027e-2-t2314+t2528+t2538-t905.*(t69-t347)).*(-1.0./2.0);
t9205 = ((t1918+t9.*(t71-t391)).*(t1961.*4.28e-4+t1965.*1.0027e-2-t2314+t2528+t2538-t905.*(t69-t347)))./2.0;
t9206 = t8640.*(t701-t775).*(-1.0./4.0);
t9207 = (t5433.*t7348)./4.0;
t9214 = (t5923.*t6872)./4.0;
t9224 = (t5952.*t6872)./4.0;
t9226 = t6462+t6499;
t9229 = (t3365.*t8640)./4.0;
t9230 = (t5234.*t7612)./4.0;
t9234 = (t5234.*t7622)./4.0;
t9239 = t2568.*(t5124-t6795).*(-1.0./4.0);
t9240 = (t3455.*t8640)./4.0;
t9241 = (t5235.*t7646)./4.0;
t9244 = t9.*t9212;
t9245 = t9.*t9213;
t9246 = -t9231;
t9247 = t17.*t9212;
t9248 = t17.*t9213;
t9249 = (t2568.*(t5124-t6795))./4.0;
t9250 = (t6014.*t6872)./4.0;
t9253 = t8.*t9225;
t9255 = t16.*t9225;
t9258 = (t2568.*t8780)./4.0;
t9265 = (t2561.*t8794)./4.0;
t9283 = (t6046.*t6957)./4.0;
t9288 = -t9281;
t9295 = (t5914.*t7079)./4.0;
t9299 = (t5919.*t7079)./4.0;
t9304 = (t6069.*t6995)./4.0;
t9305 = -t9294;
t9328 = (t5912.*t7116)./4.0;
t9329 = (t5915.*t7116)./4.0;
t9342 = -t9338;
t9347 = (t8077.*(t2821-t2864))./4.0;
t9349 = -t9341;
t9353 = t3266.*(t5110-t6808).*(-1.0./4.0);
t9356 = t3270.*(t5124-t6795).*(-1.0./4.0);
t9359 = t3275.*(t5124-t6795).*(-1.0./4.0);
t9365 = t4024.*(t3063+t3528+t3966-t5230).*(-1.0./4.0);
t9370 = (t3270.*(t5124-t6795))./4.0;
t9371 = (t3275.*(t5124-t6795))./4.0;
t9372 = t3292.*(t5124-t6795).*(-1.0./4.0);
t9378 = -t9364;
t9383 = -t9368;
t9385 = t8.*t9106.*2.62925e-3;
t9388 = (t3292.*(t5124-t6795))./4.0;
t9396 = (t3266.*t8779)./4.0;
t9398 = (t3270.*t8780)./4.0;
t9399 = (t3275.*t8780)./4.0;
t9400 = (t6046.*t7105)./4.0;
t9403 = (t3254.*t8794)./4.0;
t9407 = t8.*t9110.*2.62925e-3;
t9409 = -t9392;
t9413 = t3362.*(t5110-t6808).*(-1.0./4.0);
t9416 = t16.*t9112.*2.62925e-3;
t9418 = (t3270.*t8794)./4.0;
t9420 = (t3275.*t8794)./4.0;
t9422 = (t3292.*t8780)./4.0;
t9424 = -t9404;
t9427 = (t923-t1076).*(t5110-t6808).*(-1.0./4.0);
t9428 = -t9408;
t9429 = -t9411;
t9430 = (t3362.*(t5110-t6808))./4.0;
t9431 = (t943-t1091).*(t5110-t6808).*(-1.0./4.0);
t9434 = t17.*t8979.*1.13264871585e-2;
t9437 = t3424.*(t5110-t6808).*(-1.0./4.0);
t9443 = t9.*t8981.*1.13264871585e-2;
t9445 = ((t943-t1091).*(t5110-t6808))./4.0;
t9452 = (t3424.*(t5110-t6808))./4.0;
t9461 = (t6408.*t6761)./4.0;
t9462 = (t3362.*t8779)./4.0;
t9467 = -t9453;
t9468 = -t9454;
t9469 = -t9457;
t9470 = -t9458;
t9471 = -t9459;
t9473 = (t8779.*(t923-t1076))./4.0;
t9476 = (t8779.*(t943-t1091))./4.0;
t9480 = (t3424.*t8779)./4.0;
t9482 = t3643.*(t5124-t6795).*(-1.0./4.0);
t9483 = (t5329.*t7828)./4.0;
t9484 = (t8792.*(t943-t1091))./4.0;
t9493 = (t4152.*t8640)./4.0;
t9498 = -t9492;
t9503 = (t3643.*t8780)./4.0;
t9507 = (t5115.*t8077)./4.0;
t9512 = t8794.*(t263-t283-t310+t1265).*(-1.0./4.0);
t9516 = (t5345.*t7901)./4.0;
t9535 = (t5234.*t8070)./4.0;
t9537 = t2349+t3338+t3467+t3618+t4384+t4390;
t9539 = (t3752.*t8791)./4.0;
t9545 = -t9533;
t9551 = -t9541;
t9559 = -t9547;
t9560 = t9.*t9534;
t9561 = t17.*t9534;
t9568 = (t5443.*t7875)./4.0;
t9572 = t15.*t9216.*8.639075e-2;
t9575 = t15.*(t2810+t2988-t7937).*8.639075e-2;
t9589 = -t9582;
t9592 = -t9584;
t9595 = -t9587;
t9596 = -t9588;
t9607 = -t9598;
t9609 = (t5433.*t7982)./4.0;
t9613 = (t5434.*t7987)./4.0;
t9614 = (t2501.*t9110)./4.0;
t9624 = (t2520.*t9112)./4.0;
t9629 = t4251.*(t5124-t6795).*(-1.0./4.0);
t9631 = t4265.*(t5110-t6808).*(-1.0./4.0);
t9633 = -t9625;
t9636 = (t4251.*(t5124-t6795))./4.0;
t9641 = (t4265.*(t5110-t6808))./4.0;
t9645 = -t9640;
t9647 = (t5719.*t7797)./4.0;
t9648 = (t4251.*t8780)./4.0;
t9649 = (t5699.*t7815)./4.0;
t9651 = (t4265.*t8779)./4.0;
t9653 = (t3421.*t9028)./4.0;
t9655 = (t4252.*t8794)./4.0;
t9659 = -t9650;
t9667 = -t9658;
t9670 = (t4255.*t8802)./4.0;
t9672 = (t5628.*t7937)./4.0;
t9673 = t9.*t9361.*1.539925e-2;
t9675 = t17.*t9362.*1.539925e-2;
t9683 = (t5782.*t7796)./4.0;
t9688 = (t6761.*t6781)./4.0;
t9689 = t9.*(t824+t2543+t2699+t2707-t4767+t17.*(t260+t468+t570+t2298)).*(-1.13264871585e-2);
t9694 = t9.*(t824+t2543+t2699+t2707-t4767+t17.*(t260+t468+t570+t2298)).*1.13264871585e-2;
t9696 = t17.*(-t2550+t2696+t2698+t4771+t9.*(t260+t468+t570+t2298)+t147.*(t71-t391)).*(-1.13264871585e-2);
t9698 = -t9692;
t9708 = t4557.*(t5124-t6795).*(-1.0./4.0);
t9714 = t9.*t9187.*1.13264871585e-2;
t9717 = t3097+t3198+t3387+t3462+t3868+t5209;
t9724 = t4604.*(t5124-t6795).*(-1.0./4.0);
t9726 = (t4964.*t8640)./2.0;
t9727 = t6802+t6906;
t9728 = t6846+t6852;
t9730 = t4611.*(t5124-t6795).*(-1.0./4.0);
t9732 = t6807+t6915;
t9733 = t6856+t6859;
t9736 = -t9723;
t9738 = (t4604.*(t5124-t6795))./4.0;
t9739 = -t9725;
t9740 = (t4557.*t8780)./4.0;
t9741 = (t4611.*(t5124-t6795))./4.0;
t9742 = t17.*t9197.*1.13264871585e-2;
t9745 = t3738.*(t3085-t3419-t3773+t5128+t17.*(t208-t427).*7.35522e-1).*(-1.0./4.0);
t9746 = t6810+t6937;
t9749 = t9549.*7.35522e-1;
t9750 = (t4557.*t8794)./4.0;
t9752 = t9547.*1.666555;
t9753 = t9549.*1.666555;
t9754 = (t4298.*t8979)./4.0;
t9756 = (t4569.*t8794)./4.0;
t9757 = (t4604.*t8780)./4.0;
t9758 = (t4300.*t8981)./4.0;
t9760 = (t4611.*t8780)./4.0;
t9769 = (t4611.*t8794)./4.0;
t9775 = t15.*t9212.*1.059103943995e-1;
t9776 = t15.*t9213.*1.059103943995e-1;
t9780 = t4774.*(t5110-t6808).*(-1.0./4.0);
t9781 = (t6681.*t7079)./4.0;
t9790 = t17.*t9538.*1.539925e-2;
t9795 = -t9782;
t9799 = t7.*t9225.*1.059103943995e-1;
t9810 = -t9793;
t9811 = (t6872.*t6957)./4.0;
t9816 = -t9803;
t9821 = (t6677.*t7116)./4.0;
t9822 = (t4774.*t8779)./4.0;
t9824 = t9.*t9252.*1.13264871585e-2;
t9826 = (t5739.*t8077)./4.0;
t9827 = (t5740.*t8077)./4.0;
t9833 = t5234.*(-t3218+t3458+t3878+t8.*(t260+t468+t570+t2298).*1.666555).*(-1.0./4.0);
t9835 = (t3732.*t9110)./4.0;
t9836 = (t5750.*t8077)./4.0;
t9842 = (t5234.*(-t3218+t3458+t3878+t8.*(t260+t468+t570+t2298).*1.666555))./4.0;
t9847 = (t5329.*t8460)./4.0;
t9849 = (t2966.*(t2810+t2988-t7937))./4.0;
t9858 = (t5345.*t8464)./4.0;
t9859 = (t3780.*t9112)./4.0;
t9870 = t6872.*(t1492+t2158+t2696-t4727).*(-1.0./4.0);
t9871 = t5235.*(t3063+t3528+t3966-t5230).*(-1.0./4.0);
t9878 = -t9869;
t9880 = (t6872.*(t1492+t2158+t2696-t4727))./4.0;
t9881 = (t5235.*(t3063+t3528+t3966-t5230))./4.0;
t9887 = t2660+t3075+t3186+t3238+t3556+t3736+t4524;
t9896 = t2683+t3154+t3179+t3210+t3614+t3718+t4522;
t9899 = -t9889;
t9901 = -t9897;
t9903 = -t9900;
t9905 = (t5843.*t8077)./4.0;
t9908 = (t4024.*t9106)./4.0;
t9918 = (t5290.*t8640)./4.0;
t9931 = -t9927;
t9943 = (t5234.*t8709)./4.0;
t9945 = -t9938;
t9952 = -t9946;
t9954 = -t9947;
t9964 = t5915.*(-t1476-t1540+t2091+t2165+t2579+t8.*(t260+t468+t570+t2298)).*(-1.0./4.0);
t9967 = t1521+t2410+t2587+t3381+t3416+t3611+t3870+t3923;
t9973 = -t9970;
t9979 = t9549.*5.01208083475e-2;
t9982 = t9547.*1.17633784675e-2;
t9987 = (t6069.*t8178)./4.0;
t9997 = (t5696.*t8497)./4.0;
t10006 = (t5365.*t8693)./4.0;
t10008 = -t10001;
t10010 = t5277.*(t5110-t6808).*(-1.0./4.0);
t10012 = (t6223.*t8077)./4.0;
t10014 = (t4035.*(t2810+t2988-t7937))./4.0;
t10016 = (t4489.*t9110)./4.0;
t10019 = (t5277.*(t5110-t6808))./4.0;
t10021 = (t4509.*t9112)./4.0;
t10027 = (t4498.*t9110)./4.0;
t10030 = t7.*(t6853-t6864).*(-8.639075e-2);
t10035 = (t4514.*t9112)./4.0;
t10037 = (t5277.*t8779)./4.0;
t10038 = (t5524.*t8640)./4.0;
t10044 = t7.*(t6853-t6864).*8.639075e-2;
t10054 = -t10042;
t10056 = -t10048;
t10058 = (t5552.*t8640)./2.0;
t10059 = -t10053;
t10062 = (t3738.*t9361)./4.0;
t10065 = (t3743.*t9362)./4.0;
t10090 = -t10076;
t10095 = -t10080;
t10101 = -t10086;
t10106 = (t6193.*t8256)./4.0;
t10111 = t968+t1567+t2757+t3370+t3375+t3886+t3908+t4329;
t10112 = (t4286.*t9216)./4.0;
t10113 = (t6761.*t7540)./4.0;
t10115 = (t3489.*t9505)./4.0;
t10120 = (t6589.*t7815)./4.0;
t10132 = -t10126;
t10164 = t6449+t8225;
t10169 = t5583.*(t5110-t6808).*(-1.0./4.0);
t10176 = (t5583.*(t5110-t6808))./4.0;
t10177 = t6478+t8229;
t10178 = -t10171;
t10182 = t6469+t8237;
t10195 = (t5583.*t8779)./4.0;
t10196 = -t10183;
t10197 = -t10184;
t10205 = (t5007.*t9110)./4.0;
t10208 = -t9.*(t6452-t8229);
t10209 = -t17.*(t6452-t8229);
t10218 = t17.*(t6452-t8229);
t10220 = (t5050.*t9112)./4.0;
t10223 = (t5449.*t8979)./4.0;
t10226 = (t7079.*t7622)./2.0;
t10228 = t5713.*(t5110-t6808).*(-1.0./4.0);
t10230 = t5716.*(t5110-t6808).*(-1.0./4.0);
t10231 = (t6761.*t7901)./2.0;
t10232 = t8.*t9.*(t6452-t8229);
t10233 = (t7079.*t7612)./2.0;
t10234 = (t5448.*t8981)./4.0;
t10236 = (t5713.*(t5110-t6808))./4.0;
t10237 = (t5716.*(t5110-t6808))./4.0;
t10240 = t1604+t2211+t3880+t3884+t3988+t4006+t5227;
t10241 = (t4849.*(t2810+t2988-t7937))./4.0;
t10242 = (t5713.*t8779)./4.0;
t10245 = (t5716.*t8779)./4.0;
t10248 = (t5699.*t8791)./4.0;
t10250 = (t7116.*t7613)./2.0;
t10251 = (t5713.*t8792)./4.0;
t10253 = -t10244;
t10255 = (t7116.*t7646)./2.0;
t10264 = (t4884.*t9212)./4.0;
t10265 = (t4884.*t9213)./4.0;
t10268 = -t10257;
t10276 = -t10267;
t10278 = (t6302.*t8497)./2.0;
t10279 = (t6096.*t8640)./2.0;
t10281 = (t9196.*(t2904-t2927))./4.0;
t10293 = -t10287;
t10294 = -t10288;
t10295 = -t10289;
t10299 = t5329.*(t3085-t3419-t3773+t5128+t17.*(t208-t427).*7.35522e-1).*(-1.0./4.0);
t10300 = -t10298;
t10303 = (t6158.*t8640)./2.0;
t10307 = t4896.*(t249-t391.*(1.1e+1./1.25e+2)-t1912.*4.252e-3+t3505+t5357+t693.*(t71-t391)+t784.*(t71-t391)).*(-1.0./4.0);
t10309 = -t10306;
t10310 = (t4896.*(t249-t391.*(1.1e+1./1.25e+2)-t1912.*4.252e-3+t3505+t5357+t693.*(t71-t391)+t784.*(t71-t391)))./4.0;
t10311 = (t6750.*t8077)./4.0;
t10312 = t5884.*(t5110-t6808).*(-1.0./4.0);
t10317 = (t6767.*t8077)./4.0;
t10318 = (t5884.*(t5110-t6808))./4.0;
t10321 = t4938.*(t249-t391.*(1.1e+1./1.25e+2)-t1912.*4.252e-3+t3505+t5357+t693.*(t71-t391)+t784.*(t71-t391)).*(-1.0./4.0);
t10322 = -t10315;
t10323 = (t6762.*t8077)./4.0;
t10329 = (t2889-t2921).*(t249-t391.*(1.1e+1./1.25e+2)-t1912.*4.252e-3+t3505+t5357+t693.*(t71-t391)+t784.*(t71-t391)).*(-1.0./4.0);
t10330 = (t4938.*(t249-t391.*(1.1e+1./1.25e+2)-t1912.*4.252e-3+t3505+t5357+t693.*(t71-t391)+t784.*(t71-t391)))./4.0;
t10333 = (t7039.*t7937)./2.0;
t10336 = (t5884.*t8779)./4.0;
t10338 = ((t2889-t2921).*(t249-t391.*(1.1e+1./1.25e+2)-t1912.*4.252e-3+t3505+t5357+t693.*(t71-t391)+t784.*(t71-t391)))./4.0;
t10347 = (t5064.*(t2810+t2988-t7937))./4.0;
t10352 = t8640.*(-t2149+t2205+t693.*(t48-t349)+t784.*(t48-t349)).*(-1.0./4.0);
t10359 = (t8640.*(-t2149+t2205+t693.*(t48-t349)+t784.*(t48-t349)))./4.0;
t10362 = -t10357;
t10369 = -t10363;
t10375 = -t10366;
t10376 = -t10367;
t10377 = -t10368;
t10394 = -t10380;
t10426 = -t10417;
t10430 = (t5696.*t9028)./4.0;
t10433 = t6114.*(t5110-t6808).*(-1.0./4.0);
t10435 = t9.*(t6452-t8229).*(-7.35522e-1);
t10442 = (t6114.*(t5110-t6808))./4.0;
t10449 = t8640.*(t624+t2511-t3502-t9.*t439.*4.252e-3).*(-1.0./4.0);
t10451 = (t6114.*t8779)./4.0;
t10454 = (t7079.*t8070)./2.0;
t10455 = t6190.*(t5110-t6808).*(-1.0./4.0);
t10458 = (t8640.*(t624+t2511-t3502-t9.*t439.*4.252e-3))./4.0;
t10466 = (t7348.*t7797)./4.0;
t10468 = t3067+t3368+t9362;
t10469 = t3088+t3379+t9361;
t10470 = (t7116.*t8062)./2.0;
t10471 = (t6190.*t8779)./4.0;
t10475 = (t6190.*t8792)./4.0;
t10482 = (t5365.*t9196)./4.0;
t10493 = (t5434.*t9187)./4.0;
t10503 = (t5433.*t9197)./4.0;
t10507 = -t10502;
t10510 = -t10504;
t10513 = -t10505;
t10514 = -t10508;
t10516 = (t3249.*t9992)./4.0;
t10520 = (t6761.*t8464)./2.0;
t10528 = (t5443.*t9212)./4.0;
t10529 = (t5443.*t9213)./4.0;
t10544 = (t5434.*t9252)./4.0;
t10559 = -t10548;
t10563 = -t10553;
t10565 = (t5329.*t9361)./4.0;
t10573 = (t5345.*t9362)./4.0;
t10605 = (t5613.*(t2810+t2988-t7937))./4.0;
t10614 = (t3752.*t9992)./4.0;
t10629 = (t6397.*t8979)./4.0;
t10639 = t9.*(t6452-t8229).*(-3.867742437e-3);
t10642 = t16.*(t6452-t8229).*(-5.01208083475e-2);
t10646 = (t3421.*t10096)./4.0;
t10651 = -t10635;
t10652 = t8.*(t6452-t8229).*(-1.17633784675e-2);
t10653 = (t5929.*t9110)./2.0;
t10654 = (t5923.*t9112)./2.0;
t10657 = t9.*(t6452-t8229).*3.867742437e-3;
t10658 = -t10640;
t10659 = -t10641;
t10663 = t15.*(t6452-t8229).*(-1.059103943995e-1);
t10665 = (t6408.*t8981)./4.0;
t10672 = (t3489.*t10096)./4.0;
t10673 = t8.*(t6452-t8229).*1.17633784675e-2;
t10676 = (t5951.*t9110)./2.0;
t10682 = t15.*(t6452-t8229).*1.059103943995e-1;
t10683 = (t5952.*t9112)./2.0;
t10684 = (t5947.*t9110)./2.0;
t10697 = (t7796.*t7799)./4.0;
t10698 = -t10694;
t10699 = (t6014.*t9112)./2.0;
t10714 = (t6302.*t9028)./4.0;
t10717 = (t6589.*t8791)./4.0;
t10727 = -t10721;
t10732 = t7079.*(-t3218+t3458+t3878+t8.*(t260+t468+t570+t2298).*1.666555).*(-1.0./4.0);
t10737 = (t5345.*t9538)./4.0;
t10738 = (t5806.*(t2810+t2988-t7937))./2.0;
t10739 = (t7079.*(-t3218+t3458+t3878+t8.*(t260+t468+t570+t2298).*1.666555))./4.0;
t10747 = (t2810+t2988-t7937).*(t495+t572+t1838+t2069+t2107).*(-1.0./2.0);
t10753 = t3432+t3474+t3527+t3542+t4169+t4501+t5132;
t10761 = -t10755;
t10763 = t3466+t3470+t3498+t3537+t4168+t4500+t5156;
t10764 = -t10758;
t10765 = t7116.*(t3063+t3528+t3966-t5230).*(-1.0./4.0);
t10770 = -t10767;
t10774 = (t5928.*(t2810+t2988-t7937))./2.0;
t10781 = (t7130.*t8640)./4.0;
t10787 = t3209+t3253+t3650+t3693+t4033+t4643+t5371;
t10792 = (t7336.*t8477)./4.0;
t10801 = t7646.*(-t1476-t1540+t2091+t2165+t2579+t8.*(t260+t468+t570+t2298)).*(-1.0./4.0);
t10810 = -t10804;
t10812 = (t5696.*t9505)./4.0;
t10816 = (t7079.*t8709)./4.0;
t10831 = (t8802.*(t921+t1317-t5853))./4.0;
t10835 = t6104.*(t249-t391.*(1.1e+1./1.25e+2)-t1912.*4.252e-3+t3505+t5357+t693.*(t71-t391)+t784.*(t71-t391)).*(-1.0./4.0);
t10841 = (t6104.*(t249-t391.*(1.1e+1./1.25e+2)-t1912.*4.252e-3+t3505+t5357+t693.*(t71-t391)+t784.*(t71-t391)))./4.0;
t10844 = (t6780.*t8979)./4.0;
t10845 = (t6781.*t8981)./4.0;
t10848 = (t7336.*t8640)./4.0;
t10856 = (t6193.*t9278)./4.0;
t10860 = (t7875.*t8256)./4.0;
t10863 = t1565+t2039+t3227+t3807+t3809+t4392+t4426+t5198;
t10871 = t2065+t2074+t2166+t2245+t9534;
t10872 = -t10867;
t10876 = -t10875;
t10880 = t6304.*(t249-t391.*(1.1e+1./1.25e+2)-t1912.*4.252e-3+t3505+t5357+t693.*(t71-t391)+t784.*(t71-t391)).*(-1.0./4.0);
t10883 = -t10879;
t10896 = t16.*t3489.*(t6452-t8229).*(-1.838805e-1);
t10926 = -t10918;
t10928 = (t6761.*t9049)./2.0;
t10941 = t7149+t8984;
t10947 = t8.*t10931;
t10948 = t16.*t10931;
t10949 = t17.*t10783.*1.539925e-2;
t10974 = t8218+t8230;
t10975 = (t6729.*t9110)./4.0;
t10987 = t5634.*(t6853-t6864).*(-1.0./4.0);
t11015 = -t11009;
t11020 = t16.*t4021.*(t6452-t8229).*(-4.1663875e-1);
t11025 = t8.*t4024.*(t6452-t8229).*(-4.1663875e-1);
t11033 = (t6302.*t9505)./4.0;
t11035 = -t11029;
t11042 = -t11034;
t11049 = t9110.*(-t1540+t2091+t2579+t8.*(t260+t468+t570+t2298)).*(-1.0./4.0);
t11051 = (t9110.*(-t1540+t2091+t2579+t8.*(t260+t468+t570+t2298)))./4.0;
t11053 = t4884.*(t6452-t8229).*(-1.0./4.0);
t11054 = (t6957.*t9112)./4.0;
t11056 = t4900.*(t6452-t8229).*(-1.0./4.0);
t11057 = (t4884.*(t6452-t8229))./4.0;
t11059 = (t4900.*(t6452-t8229))./4.0;
t11060 = (t6995.*t9110)./4.0;
t11061 = (t8077.*t8437)./4.0;
t11069 = t4939.*(t6452-t8229).*(-1.0./4.0);
t11073 = t9112.*(t1492+t2158+t2696-t4727).*(-1.0./4.0);
t11074 = (t4939.*(t6452-t8229))./4.0;
t11086 = (t7079.*t9098)./2.0;
t11087 = (t7066.*t9110)./2.0;
t11091 = -t11088;
t11093 = -t11090;
t11095 = -t11092;
t11099 = (t7116.*t9106)./2.0;
t11100 = (t7105.*t9112)./2.0;
t11117 = -t11110;
t11119 = (t8191.*t8497)./4.0;
t11153 = (t7538.*t8979)./4.0;
t11158 = -t11151;
t11159 = (t7540.*t8981)./4.0;
t11161 = (t6967.*(t2810+t2988-t7937))./2.0;
t11178 = t5218.*(t6452-t8229).*(-1.0./4.0);
t11183 = (t5218.*(t6452-t8229))./4.0;
t11192 = -t11185;
t11193 = (t7039.*t9216)./2.0;
t11197 = t6966.*(t249-t391.*(1.1e+1./1.25e+2)-t1912.*4.252e-3+t3505+t5357+t693.*(t71-t391)+t784.*(t71-t391)).*(-1.0./4.0);
t11202 = (t6761.*t9362)./4.0;
t11203 = (t6966.*(t249-t391.*(1.1e+1./1.25e+2)-t1912.*4.252e-3+t3505+t5357+t693.*(t71-t391)+t784.*(t71-t391)))./4.0;
t11204 = ((t3063+t3528+t3966-t5230).*(-t1476-t1540+t2091+t2165+t2579+t8.*(t260+t468+t570+t2298)))./2.0;
t11214 = -t11207;
t11215 = -t11208;
t11224 = (t5699.*t9992)./4.0;
t11241 = (t8077.*t8711)./4.0;
t11249 = (t7079.*(t3098+t3199+t3211-t3221+t3678+t4612))./4.0;
t11250 = (t7402.*t9110)./4.0;
t11263 = -t11256;
t11264 = (t7828.*t8979)./4.0;
t11265 = -t11257;
t11273 = (t7116.*t9269)./4.0;
t11274 = (t7434.*t9112)./4.0;
t11276 = t16.*t5365.*(t6452-t8229).*(-1.0./4.0);
t11282 = -t11272;
t11296 = -t11287;
t11305 = -t11299;
t11306 = (t3743.*t10783)./4.0;
t11314 = t5442.*(t6452-t8229).*(-1.0./4.0);
t11316 = t5443.*(t6452-t8229).*(-1.0./4.0);
t11317 = -t11309;
t11318 = (t7901.*t8981)./4.0;
t11324 = (t5442.*(t6452-t8229))./4.0;
t11325 = (t5443.*(t6452-t8229))./4.0;
t11326 = (t6761.*t9538)./4.0;
t11344 = t7547+t9127;
t11345 = t7215.*(t249-t391.*(1.1e+1./1.25e+2)-t1912.*4.252e-3+t3505+t5357+t693.*(t71-t391)+t784.*(t71-t391)).*(-1.0./4.0);
t11347 = (t8433.*t8640)./4.0;
t11350 = (t7215.*(t249-t391.*(1.1e+1./1.25e+2)-t1912.*4.252e-3+t3505+t5357+t693.*(t71-t391)+t784.*(t71-t391)))./4.0;
t11365 = t8272.*(t5124-t6795).*(-1.0./4.0);
t11366 = -t11358;
t11383 = t7.*t10931.*1.059103943995e-1;
t11392 = (t8272.*t8780)./4.0;
t11399 = -t11389;
t11402 = t8794.*(t263+t1265-t7252-t5.*t12.*1.0442e-1).*(-1.0./4.0);
t11403 = t5646.*(t6452-t8229).*(-1.0./4.0);
t11404 = t16.*t5234.*(t6452-t8229).*(-4.1663875e-1);
t11405 = t8.*t5235.*(t6452-t8229).*(-4.1663875e-1);
t11409 = -t11397;
t11413 = t16.*t5234.*(t6452-t8229).*4.1663875e-1;
t11414 = t8.*t5235.*(t6452-t8229).*4.1663875e-1;
t11439 = t16.*(t8219-t8226).*(-4.38178973375e-3);
t11445 = t16.*(t8219-t8226).*4.38178973375e-3;
t11450 = (t8477.*t8693)./4.0;
t11465 = -t11462;
t11479 = t7796.*(t824+t2543+t2699+t2707-t4767+t17.*(t260+t468+t570+t2298)).*(-1.0./4.0);
t11482 = t7797.*(-t2550+t2696+t2698+t4771+t9.*(t260+t468+t570+t2298)+t147.*(t71-t391)).*(-1.0./4.0);
t11487 = (t8191.*t9028)./4.0;
t11498 = (t8640.*t8693)./4.0;
t11500 = -t11494;
t11504 = -t11497;
t11510 = -t11506;
t11515 = -t11513;
t11516 = (t6302.*t10096)./4.0;
t11518 = -t11514;
t11529 = t8.*t6046.*(t6452-t8229).*(-1.0./4.0);
t11534 = t6957.*(-t3045-t3218+t3458+t3539+t3878+t8.*(t260+t468+t570+t2298).*1.666555).*(-1.0./2.0);
t11538 = t16.*t6069.*(t6452-t8229).*(-1.0./4.0);
t11547 = (t6853-t6864).*(t921+t1317-t5853).*(-1.0./4.0);
t11556 = (t7796.*t9252)./4.0;
t11558 = (t8460.*t8979)./4.0;
t11564 = (t8464.*t8981)./4.0;
t11575 = t15.*(t9128+t7.*(t5026+t5.*(t2959-t2967)).*1.225946).*(-8.639075e-2);
t11584 = t15.*(t9128+t7.*(t5026+t5.*(t2959-t2967)).*1.225946).*8.639075e-2;
t11586 = t6175.*(t6452-t8229).*(-1.0./4.0);
t11587 = -t11579;
t11593 = t16.*t5696.*(t6452-t8229).*(-1.838805e-1);
t11595 = (t6175.*(t6452-t8229))./4.0;
t11596 = t6196.*(t6452-t8229).*(-1.0./4.0);
t11601 = (t6196.*(t6452-t8229))./4.0;
t11611 = ((t3479-t3544+t2772.*(t48-t349)+t2775.*(t48-t349)).*(t249-t391.*(1.1e+1./1.25e+2)-t1912.*4.252e-3+t3505+t5357+t693.*(t71-t391)+t784.*(t71-t391)))./4.0;
t11616 = t9106.*(-t1476-t1540+t2091+t2165+t2579+t8.*(t260+t468+t570+t2298)).*(-1.0./4.0);
t11618 = (t9106.*(-t1476-t1540+t2091+t2165+t2579+t8.*(t260+t468+t570+t2298)))./4.0;
t11619 = t7105.*(-t3045-t3218+t3458+t3539+t3878+t8.*(t260+t468+t570+t2298).*1.666555).*(-1.0./4.0);
t11621 = (t7105.*(-t3045-t3218+t3458+t3539+t3878+t8.*(t260+t468+t570+t2298).*1.666555))./4.0;
t11623 = t8697.*(t5124-t6795).*(-1.0./4.0);
t11627 = (t5234.*(t8646-t8.*(t30.*(t2425-t2468)+t68.*(t2425-t2468)).*1.666555))./4.0;
t11628 = (t8697.*(t5124-t6795))./4.0;
t11635 = (t8794.*(-t262+t1056+t1250+t5078+t5282+t4.*t13.*1.0442e-1))./4.0;
t11640 = (t8697.*t8780)./4.0;
t11662 = -t11655;
t11663 = (t8054.*t9212)./4.0;
t11664 = (t8054.*t9213)./4.0;
t11665 = t7980.*(t249-t391.*(1.1e+1./1.25e+2)-t1912.*4.252e-3+t3505+t5357+t693.*(t71-t391)+t784.*(t71-t391)).*(-1.0./4.0);
t11669 = (t8050.*t9225)./4.0;
t11675 = (t7980.*(t249-t391.*(1.1e+1./1.25e+2)-t1912.*4.252e-3+t3505+t5357+t693.*(t71-t391)+t784.*(t71-t391)))./4.0;
t11677 = t6385.*(t6452-t8229).*(-1.0./4.0);
t11678 = -t11659;
t11679 = -t11660;
t11681 = (t6385.*(t6452-t8229))./4.0;
t11687 = t7.*(t4542-t6448).*(t2810+t2988-t7937).*(-1.0./4.0);
t11691 = ((t2752+t3814-t4385-t9.*t439.*3.127439544e-3).*(t249-t391.*(1.1e+1./1.25e+2)-t1912.*4.252e-3+t3505+t5357+t693.*(t71-t391)+t784.*(t71-t391)))./4.0;
t11692 = (t7.*(t4542-t6448).*(t2810+t2988-t7937))./4.0;
t11700 = (t7.*(t6460-t35.*(t2425-t2468)).*(t2810+t2988-t7937))./4.0;
t11704 = (t8177.*(t2810+t2988-t7937))./4.0;
t11706 = t8077.*(t1786+t2973-t7703-t5.*t12.*3.746479959e-1).*(-1.0./4.0);
t11745 = (t7.*(t4650+t34.*(t2425-t2468))+t47.*(t2425-t2468)).*(t2810+t2988-t7937).*(-1.0./4.0);
t11750 = (t8077.*t9325)./4.0;
t11762 = -t11753;
t11773 = -t11764;
t11779 = ((t5110-t6808).*(t5027-t7134))./4.0;
t11781 = ((t5124-t6795).*(t5027-t7134))./4.0;
t11785 = t6546.*(t6452-t8229).*(-1.0./4.0);
t11790 = (t6546.*(t6452-t8229))./4.0;
t11794 = (t8794.*t8931)./4.0;
t11798 = (t6175.*t10408)./4.0;
t11802 = t8779.*(t5027-t7134).*(-1.0./4.0);
t11806 = t8780.*(t5027-t7134).*(-1.0./4.0);
t11810 = -t11797;
t11813 = (t8779.*(t5027-t7134))./4.0;
t11814 = -t11805;
t11815 = (t8780.*(t5027-t7134))./4.0;
t11816 = (t5345.*t10783)./4.0;
t11830 = -t11826;
t11834 = t3249.*(t9125+t7.*(t5026+t5.*(t2959-t2967)).*1.666555).*(-1.0./4.0);
t11837 = (t3249.*(t9125+t7.*(t5026+t5.*(t2959-t2967)).*1.666555))./4.0;
t11842 = t16.*t6302.*(t6452-t8229).*(-1.838805e-1);
t11845 = t16.*t6302.*(t6452-t8229).*1.838805e-1;
t11849 = (t8477.*t9196)./4.0;
t11856 = t11658.*1.666555;
t11857 = t11660.*1.666555;
t11860 = t11658.*7.35522e-1;
t11861 = t11659.*7.35522e-1;
t11863 = t11660.*7.35522e-1;
t11865 = t11661.*7.35522e-1;
t11877 = (t2904-t2927).*(t8219-t8226).*(-1.0./4.0);
t11880 = ((t2904-t2927).*(t8219-t8226))./4.0;
t11881 = (t8191.*t9505)./2.0;
t11895 = t3752.*(t9125+t7.*(t5026+t5.*(t2959-t2967)).*1.666555).*(-1.0./4.0);
t11897 = t8497.*(t249-t391.*(1.1e+1./1.25e+2)-t1912.*4.252e-3+t3505+t5357+t693.*(t71-t391)+t784.*(t71-t391)).*(-1.0./4.0);
t11898 = (t3752.*(t9125+t7.*(t5026+t5.*(t2959-t2967)).*1.666555))./4.0;
t11899 = (t8497.*(t249-t391.*(1.1e+1./1.25e+2)-t1912.*4.252e-3+t3505+t5357+t693.*(t71-t391)+t784.*(t71-t391)))./4.0;
t11912 = (t8640.*t9196)./4.0;
t11914 = t8.*t6872.*(t6452-t8229).*(-1.0./4.0);
t11915 = t8547.*(t249-t391.*(1.1e+1./1.25e+2)-t1912.*4.252e-3+t3505+t5357+t693.*(t71-t391)+t784.*(t71-t391)).*(-1.0./4.0);
t11923 = (t8.*t6872.*(t6452-t8229))./4.0;
t11924 = (t8547.*(t249-t391.*(1.1e+1./1.25e+2)-t1912.*4.252e-3+t3505+t5357+t693.*(t71-t391)+t784.*(t71-t391)))./4.0;
t11925 = t6969.*(t6452-t8229).*(-1.0./4.0);
t11938 = -t11934;
t11943 = t6872.*(t16.*(t30.*(t2425-t2468)+t68.*(t2425-t2468))+t8.*(t7.*(t4650+t34.*(t2425-t2468))+t47.*(t2425-t2468))).*(-1.0./4.0);
t11948 = (t6872.*(t16.*(t30.*(t2425-t2468)+t68.*(t2425-t2468))+t8.*(t7.*(t4650+t34.*(t2425-t2468))+t47.*(t2425-t2468))))./4.0;
t11950 = -t9.*(t7693+t9904);
t11951 = -t17.*(t7693+t9904);
t11952 = (t8979.*t9048)./4.0;
t11953 = (t4255.*t11336)./4.0;
t11959 = t8979.*(t3085-t3419-t3773+t5128+t17.*(t208-t427).*7.35522e-1).*(-1.0./2.0);
t11964 = (t8981.*t9049)./4.0;
t11969 = t3476+t3487+t3540+t3561+t3585+t9309;
t11970 = t9.*(t7693+t9904);
t11979 = (t4286.*t11343)./4.0;
t11981 = t7124.*(t6452-t8229).*(-1.0./4.0);
t11984 = t4286.*(t9128+t7.*(t5026+t5.*(t2959-t2967)).*1.225946).*(-1.0./4.0);
t11985 = (t7124.*(t6452-t8229))./4.0;
t11986 = (t4286.*(t9128+t7.*(t5026+t5.*(t2959-t2967)).*1.225946))./4.0;
t12006 = t5365.*(t8219-t8226).*(-1.0./4.0);
t12008 = t11659.*3.867742437e-3;
t12014 = t11661.*1.563719772e-3;
t12024 = (t7336.*t10141)./2.0;
t12025 = t7217.*(t6452-t8229).*(-1.0./4.0);
t12027 = (t7217.*(t6452-t8229))./4.0;
t12029 = -t12028;
t12031 = -t12030;
t12037 = -t12034;
t12039 = t9285.*(t5110-t6808).*(-1.0./4.0);
t12043 = (t9285.*(t5110-t6808))./4.0;
t12051 = (t8779.*t9285)./4.0;
t12068 = t17.*(t7693+t9904).*(-7.35522e-1);
t12075 = t16.*t7079.*(t6452-t8229).*(-4.1663875e-1);
t12076 = -t12072;
t12080 = -t12077;
t12086 = t8.*t7116.*(t6452-t8229).*(-4.1663875e-1);
t12095 = t9499.*(t5110-t6808).*(-1.0./4.0);
t12098 = (t9499.*(t5110-t6808))./4.0;
t12101 = -t12097;
t12102 = -t12100;
t12103 = (t8779.*t9499)./4.0;
t12108 = -t12106;
t12109 = (t8979.*t9361)./2.0;
t12110 = (t8981.*t9362)./2.0;
t12113 = t9028.*(t249-t391.*(1.1e+1./1.25e+2)-t1912.*4.252e-3+t3505+t5357+t693.*(t71-t391)+t784.*(t71-t391)).*(-1.0./2.0);
t12114 = t7676.*(t6452-t8229).*(-1.0./4.0);
t12117 = (t9028.*(t249-t391.*(1.1e+1./1.25e+2)-t1912.*4.252e-3+t3505+t5357+t693.*(t71-t391)+t784.*(t71-t391)))./2.0;
t12118 = (t7676.*(t6452-t8229))./4.0;
t12157 = -t12150;
t12167 = (t6175.*t10931)./4.0;
t12170 = t7815.*(t6452-t8229).*(-1.0./4.0);
t12174 = (t7815.*(t6452-t8229))./4.0;
t12177 = (t8077.*(-t1785+t2869+t2960+t5489+t5720+t4.*t13.*3.746479959e-1))./4.0;
t12195 = t7.*t12042.*8.639075e-2;
t12199 = (t8981.*t9538)./2.0;
t12203 = -t12196;
t12205 = -t12197;
t12209 = t15.*t12050.*8.639075e-2;
t12212 = t17.*(t7693+t9904).*(-3.867742437e-3);
t12214 = t7937.*(t6452-t8229).*(-1.0./4.0);
t12215 = (t8191.*t10096)./4.0;
t12220 = -t12211;
t12221 = t17.*(t7693+t9904).*3.867742437e-3;
t12223 = -t12217;
t12246 = t9686.*(t5124-t6795).*(-1.0./4.0);
t12250 = -t12243;
t12252 = (t9686.*(t5124-t6795))./4.0;
t12257 = -t12249;
t12262 = (t8794.*t9685)./4.0;
t12267 = (t8780.*t9686)./4.0;
t12270 = t8050.*(t6452-t8229).*(-1.0./4.0);
t12271 = t8053.*(t6452-t8229).*(-1.0./4.0);
t12274 = t8054.*(t6452-t8229).*(-1.0./4.0);
t12275 = -t12269;
t12276 = -t12272;
t12277 = (t8054.*(t6452-t8229))./4.0;
t12278 = t8065.*(t6452-t8229).*(-1.0./4.0);
t12280 = (t6452-t8229).*(t917-t1669+t2469+t2475+t3495+t3591).*(-1.0./4.0);
t12281 = ((t6452-t8229).*(t917-t1669+t2469+t2475+t3495+t3591))./4.0;
t12286 = (t9212.*t9236)./4.0;
t12287 = (t9213.*t9236)./4.0;
t12288 = (t9225.*(t2810+t2988-t7937))./4.0;
t12305 = -t12299;
t12308 = (t5634.*t11336)./4.0;
t12311 = (t9212.*t9278)./4.0;
t12312 = (t9213.*t9278)./4.0;
t12319 = (t5628.*t11343)./4.0;
t12323 = t9828.*(t5124-t6795).*(-1.0./4.0);
t12325 = t9830.*(t5124-t6795).*(-1.0./4.0);
t12329 = t5628.*(t9128+t7.*(t5026+t5.*(t2959-t2967)).*1.225946).*(-1.0./4.0);
t12330 = (t9828.*(t5124-t6795))./4.0;
t12336 = t8256.*(t6452-t8229).*(-1.0./4.0);
t12337 = (t5628.*(t9128+t7.*(t5026+t5.*(t2959-t2967)).*1.225946))./4.0;
t12340 = (t8256.*(t6452-t8229))./4.0;
t12341 = (t8780.*t9828)./4.0;
t12342 = (t8780.*t9830)./4.0;
t12344 = (t8794.*t9828)./4.0;
t12346 = (t8794.*t9830)./4.0;
t12353 = t8310.*(t6452-t8229).*(-1.0./4.0);
t12354 = t5699.*(t9125+t7.*(t5026+t5.*(t2959-t2967)).*1.666555).*(-1.0./4.0);
t12355 = t9884.*(t5110-t6808).*(-1.0./4.0);
t12359 = (t5699.*(t9125+t7.*(t5026+t5.*(t2959-t2967)).*1.666555))./4.0;
t12360 = -t9.*(t9547+t16.*(-t211+t5081+t7275));
t12361 = -t17.*(t9547+t16.*(-t211+t5081+t7275));
t12364 = -t12362;
t12367 = t9310.*(t249-t391.*(1.1e+1./1.25e+2)-t1912.*4.252e-3+t3505+t5357+t693.*(t71-t391)+t784.*(t71-t391)).*(-1.0./4.0);
t12368 = (t8779.*t9884)./4.0;
t12369 = t17.*(t9547+t16.*(-t211+t5081+t7275));
t12371 = -t12366;
t12372 = (t9310.*(t249-t391.*(1.1e+1./1.25e+2)-t1912.*4.252e-3+t3505+t5357+t693.*(t71-t391)+t784.*(t71-t391)))./4.0;
t12376 = -t12374;
t12390 = (t8050.*t10408)./4.0;
t12404 = t9505.*(t249-t391.*(1.1e+1./1.25e+2)-t1912.*4.252e-3+t3505+t5357+t693.*(t71-t391)+t784.*(t71-t391)).*(-1.0./4.0);
t12409 = (t9505.*(t249-t391.*(1.1e+1./1.25e+2)-t1912.*4.252e-3+t3505+t5357+t693.*(t71-t391)+t784.*(t71-t391)))./4.0;
t12410 = t16.*t8477.*(t6452-t8229).*(-1.0./4.0);
t12425 = t16.*t8191.*(t6452-t8229).*(-1.838805e-1);
t12437 = (t6452-t8229).*(t2433+t2449-t3048-t3102+t3223+t3232).*(-1.0./4.0);
t12438 = t8.*(t6452-t8229).*(-t1476-t1540+t2091+t2165+t2579+t8.*(t260+t468+t570+t2298)).*4.1663875e-1;
t12439 = ((t6452-t8229).*(t2433+t2449-t3048-t3102+t3223+t3232))./4.0;
t12460 = (t8693.*t10141)./4.0;
t12465 = t9.*(t9547+t16.*(-t211+t5081+t7275)).*(-7.35522e-1);
t12467 = t16.*t8640.*(t6452-t8229).*(-1.0./4.0);
t12470 = (t16.*t8640.*(t6452-t8229))./4.0;
t12472 = (t4255.*t12042)./4.0;
t12473 = t8640.*(t8315+t8.*(t30.*(t2425-t2468)+t68.*(t2425-t2468))).*(-1.0./4.0);
t12476 = (t8640.*(t8315+t8.*(t30.*(t2425-t2468)+t68.*(t2425-t2468))))./4.0;
t12480 = (t4286.*t12050)./4.0;
t12502 = t8791.*(t6452-t8229).*(-1.0./4.0);
t12530 = -t12528;
t12532 = t6589.*(t9125+t7.*(t5026+t5.*(t2959-t2967)).*1.666555).*(-1.0./4.0);
t12534 = -t12531;
t12536 = (t6589.*(t9125+t7.*(t5026+t5.*(t2959-t2967)).*1.666555))./4.0;
t12539 = -t12535;
t12541 = (t8077.*t10754)./4.0;
t12542 = t9.*(t9547+t16.*(-t211+t5081+t7275)).*(-1.563719772e-3);
t12551 = -t12548;
t12561 = -t12559;
t12564 = t1952+t2001+t2619+t2624+t11626;
t12566 = -t12565;
t12582 = -t12573;
t12591 = -t12590;
t12597 = (t11336.*(t921+t1317-t5853))./4.0;
t12602 = -t12601;
t12606 = -t12603;
t12609 = (t7039.*t11343)./4.0;
t12616 = t9104.*(t6452-t8229).*(-1.0./4.0);
t12618 = (t9104.*(t6452-t8229))./4.0;
t12621 = t16.*t9110.*(t6452-t8229).*(-1.0./4.0);
t12624 = t8.*t9112.*(t6452-t8229).*(-1.0./4.0);
t12629 = t10501.*(t5110-t6808).*(-1.0./4.0);
t12630 = -t12627;
t12631 = (t10501.*(t5110-t6808))./4.0;
t12635 = (t8779.*t10501)./4.0;
t12636 = t10096.*(t249-t391.*(1.1e+1./1.25e+2)-t1912.*4.252e-3+t3505+t5357+t693.*(t71-t391)+t784.*(t71-t391)).*(-1.0./2.0);
t12638 = (t8792.*t10501)./4.0;
t12642 = (t10096.*(t249-t391.*(1.1e+1./1.25e+2)-t1912.*4.252e-3+t3505+t5357+t693.*(t71-t391)+t784.*(t71-t391)))./2.0;
t12646 = (t8050.*t10931)./4.0;
t12692 = (t3249.*t12464)./4.0;
t12695 = -t12687;
t12696 = t1463+t2000+t2268+t2570+t7693+t9904;
t12697 = (t8077.*t10964)./4.0;
t12700 = (t8077.*t10966)./4.0;
t12701 = t9216.*(t6452-t8229).*(-1.0./4.0);
t12704 = (t6452-t8229).*(t2810+t2988-t7937).*(-1.0./4.0);
t12714 = t9236.*(t6452-t8229).*(-1.0./4.0);
t12717 = (t9236.*(t6452-t8229))./4.0;
t12722 = -t12719;
t12729 = -t12725;
t12732 = -t12727;
t12736 = t9278.*(t6452-t8229).*(-1.0./4.0);
t12739 = (t9278.*(t6452-t8229))./4.0;
t12742 = t15.*t12589.*8.639075e-2;
t12743 = -t12740;
t12755 = -t12749;
t12757 = -t12752;
t12759 = (t3752.*t12464)./4.0;
t12760 = t9333.*(t6452-t8229).*(-1.0./4.0);
t12763 = (t9333.*(t6452-t8229))./4.0;
t12826 = t9525.*(t6452-t8229).*(-1.0./4.0);
t12828 = (t10408.*(t2810+t2988-t7937))./4.0;
t12837 = -t12832;
t12843 = t10398.*(t249-t391.*(1.1e+1./1.25e+2)-t1912.*4.252e-3+t3505+t5357+t693.*(t71-t391)+t784.*(t71-t391)).*(-1.0./2.0);
t12850 = -t12844;
t12852 = t16.*(t6452-t8229).*(t249-t391.*(1.1e+1./1.25e+2)-t1912.*4.252e-3+t3505+t5357+t693.*(t71-t391)+t784.*(t71-t391)).*1.838805e-1;
t12860 = t1954+t2161+t2276+t9101+t9549;
t12872 = (t8981.*t10783)./4.0;
t12893 = t8640.*(t8219-t8226).*(-1.0./4.0);
t12894 = -t12890;
t12897 = (t5443.*t12266)./4.0;
t12905 = -t12900;
t12920 = -t12916;
t12931 = -t12926;
t12943 = -t12939;
t12954 = t16.*t12667.*4.38178973375e-3;
t12961 = -t12955;
t12972 = (t8.*(t6452-t8229).*(-t3045-t3218+t3458+t3539+t3878+t8.*(t260+t468+t570+t2298).*1.666555))./4.0;
t13016 = -t13011;
t13024 = (t8643-t8.*(t30.*(t2425-t2468)+t68.*(t2425-t2468)).*7.35522e-1).*(t249-t391.*(1.1e+1./1.25e+2)-t1912.*4.252e-3+t3505+t5357+t693.*(t71-t391)+t784.*(t71-t391)).*(-1.0./4.0);
t13031 = ((t8643-t8.*(t30.*(t2425-t2468)+t68.*(t2425-t2468)).*7.35522e-1).*(t249-t391.*(1.1e+1./1.25e+2)-t1912.*4.252e-3+t3505+t5357+t693.*(t71-t391)+t784.*(t71-t391)))./4.0;
t13035 = (t4286.*t12589)./4.0;
t13038 = t1666+t1767+t1791+t2335+t12387;
t13067 = -t13060;
t13090 = -t13083;
t13098 = t9992.*(t6452-t8229).*(-1.0./4.0);
t13119 = (t10850.*(t2810+t2988-t7937))./4.0;
t13120 = (t12042.*(t921+t1317-t5853))./4.0;
t13138 = (t7039.*t12050)./4.0;
t13141 = t9110.*(t8219-t8226).*(-1.0./4.0);
t13142 = -t13137;
t13144 = (t9110.*(t8219-t8226))./4.0;
t13154 = (t5699.*t12464)./4.0;
t13161 = t16.*t10141.*(t6452-t8229).*(-1.0./4.0);
t13165 = -t13163;
t13170 = -t13169;
t13201 = (t3752.*t12898)./4.0;
t13218 = -t13215;
t13228 = t15.*(t2810+t2988-t12589).*8.639075e-2;
t13237 = -t13236;
t13254 = (t8077.*t11907)./4.0;
t13256 = -t13248;
t13273 = t428+t2143+t2169+t3259+t3274+t9101+t9549;
t13284 = (t5628.*t12589)./4.0;
t13307 = (t11228.*(t2810+t2988-t7937))./4.0;
t13314 = -t13311;
t13326 = t3097+t3387+t3462+t3868+t8148+t10081;
t13337 = (t2966.*(t2810+t2988-t12589))./4.0;
t13338 = (t6872.*t12392)./4.0;
t13343 = t5234.*(t3116+t3486+t3963+t11671.*1.666555).*(-1.0./4.0);
t13347 = -t13340;
t13349 = (t5234.*(t3116+t3486+t3963+t11671.*1.666555))./4.0;
t13355 = -t13351;
t13360 = -t13353;
t13363 = -t13358;
t13368 = -t13365;
t13399 = -t13396;
t13408 = -t13406;
t13416 = t1521+t3381+t3416+t3611+t3870+t3923+t7831+t9319;
t13433 = (t5365.*t12866)./4.0;
t13436 = (t4035.*(t2810+t2988-t12589))./4.0;
t13448 = -t13446;
t13449 = (t6069.*t12667)./4.0;
t13496 = t9165+t11660;
t13508 = t9174+t11658;
t13530 = -t9.*(t9166-t11658);
t13532 = -t17.*(t9166-t11658);
t13560 = (t6761.*t12563)./4.0;
t13579 = (t4849.*(t2810+t2988-t12589))./4.0;
t13585 = (t5699.*t12898)./4.0;
t13590 = (t8256.*t12266)./4.0;
t13596 = t10141.*(t8219-t8226).*(-1.0./4.0);
t13599 = (t10141.*(t8219-t8226))./4.0;
t13610 = (t13150.*(t2904-t2927))./4.0;
t13613 = (t7039.*t12589)./4.0;
t13614 = (t7937.*t12396)./4.0;
t13618 = (t5064.*(t2810+t2988-t12589))./4.0;
t13622 = -t13617;
t13624 = t9.*(t9166-t11658).*(-7.35522e-1);
t13625 = t17.*(t9166-t11658).*(-7.35522e-1);
t13627 = t3148+t3202+t3206+t3646+t8117+t10797;
t13632 = -t13630;
t13640 = -t13636;
t13641 = -t13637;
t13694 = -t13689;
t13698 = (t5365.*t13150)./4.0;
t13709 = -t13706;
t13730 = (t5613.*(t2810+t2988-t12589))./4.0;
t13752 = -t13748;
t13753 = -t13749;
t13780 = (t6589.*t12898)./4.0;
t13785 = -t13774;
t13786 = -t13775;
t13798 = t11343.*(t6452-t8229).*(-1.0./4.0);
t13801 = ((t9125+t7.*(t5026+t5.*(t2959-t2967)).*1.666555).*(t6452-t8229))./4.0;
t13806 = ((t6452-t8229).*(t9128+t7.*(t5026+t5.*(t2959-t2967)).*1.225946))./4.0;
t13813 = (t5806.*(t2810+t2988-t12589))./4.0;
t13816 = t7079.*(t3116+t3486+t3963+t11671.*1.666555).*(-1.0./4.0);
t13817 = (t12049.*(t2810+t2988-t7937))./4.0;
t13818 = (t2810+t2988-t12589).*(t495+t572+t1838+t2069+t2107).*(-1.0./4.0);
t13822 = (t7079.*(t3116+t3486+t3963+t11671.*1.666555))./4.0;
t13824 = (t7116.*t12792)./4.0;
t13839 = -t13833;
t13840 = -t13834;
t13842 = -t13837;
t13845 = (t5928.*(t2810+t2988-t12589))./4.0;
t13849 = -t13848;
t13853 = (t3489.*t13578)./4.0;
t13869 = (t8802.*t12385)./4.0;
t13888 = -t13887;
t13895 = -t13891;
t13915 = t1565+t2039+t3807+t3809+t4392+t4426+t8143+t10091;
t13945 = -t13941;
t13980 = (t9278.*t12266)./4.0;
t13993 = t9110.*(t1292+t2073+t2694+t11671).*(-1.0./4.0);
t13994 = (t9112.*t12392)./4.0;
t13996 = (t9110.*(t1292+t2073+t2694+t11671))./4.0;
t14016 = (t6967.*(t2810+t2988-t12589))./4.0;
t14021 = -t14018;
t14022 = (t9216.*t12396)./4.0;
t14073 = (t8477.*t12866)./4.0;
t14087 = (t5696.*t13578)./4.0;
t14094 = t12050.*(t6452-t8229).*(-1.0./4.0);
t14095 = (t12050.*(t6452-t8229))./4.0;
t14096 = (t8640.*t12866)./4.0;
t14103 = t12385.*(t6853-t6864).*(-1.0./4.0);
t14146 = t12185.*(t6452-t8229).*(-1.0./4.0);
t14148 = (t6302.*t13578)./4.0;
t14149 = t7.*(t4542-t6448).*(t2810+t2988-t12589).*(-1.0./4.0);
t14151 = (t7.*(t4542-t6448).*(t2810+t2988-t12589))./4.0;
t14153 = (t8177.*(t2810+t2988-t12589))./4.0;
t14154 = (t7.*(t6460-t35.*(t2425-t2468)).*(t2810+t2988-t12589))./4.0;
t14169 = (t7.*(t4650+t34.*(t2425-t2468))+t47.*(t2425-t2468)).*(t2810+t2988-t12589).*(-1.0./4.0);
t14173 = ((t7.*(t4650+t34.*(t2425-t2468))+t47.*(t2425-t2468)).*(t2810+t2988-t12589))./4.0;
t14187 = (t3421.*t14035)./4.0;
t14189 = (t3489.*t14035)./4.0;
t14221 = (t8477.*t13150)./4.0;
t14244 = (t8640.*t13150)./4.0;
t14254 = (t2904-t2927).*(t3625+t3660+t9166-t11658).*(-1.0./4.0);
t14255 = ((t2904-t2927).*(t3625+t3660+t9166-t11658))./4.0;
t14260 = t12464.*(t6452-t8229).*(-1.0./4.0);
t14261 = (t12464.*(t6452-t8229))./4.0;
t14274 = (t7079.*(t3098+t3211-t3221+t3678+t8102+t10798))./4.0;
t14275 = (t9110.*t13019)./4.0;
t14343 = t12589.*(t6452-t8229).*(-1.0./4.0);
t14344 = (t12589.*(t6452-t8229))./4.0;
t14356 = (t9212.*t13140)./4.0;
t14357 = (t9213.*t13140)./4.0;
t14358 = (t9225.*(t2810+t2988-t12589))./4.0;
t14364 = (t5696.*t14035)./4.0;
t14389 = t12669.*(t6452-t8229).*(-1.0./4.0);
t14395 = (t8191.*t13578)./4.0;
t14457 = (t10141.*t12866)./4.0;
t14488 = t12898.*(t6452-t8229).*(-1.0./4.0);
t14490 = (t12898.*(t6452-t8229))./4.0;
t14567 = (t11336.*t12385)./2.0;
t14574 = (t11343.*t12396)./2.0;
t14577 = t12396.*(t9128+t7.*(t5026+t5.*(t2959-t2967)).*1.225946).*(-1.0./2.0);
t14612 = (t6452-t8229).*(t2810+t2988-t12589).*(-1.0./4.0);
t14615 = ((t6452-t8229).*(t2810+t2988-t12589))./4.0;
t14616 = t13140.*(t6452-t8229).*(-1.0./4.0);
t14617 = (t13140.*(t6452-t8229))./4.0;
t14637 = t13578.*(t249-t391.*(1.1e+1./1.25e+2)-t1912.*4.252e-3+t3505+t5357+t693.*(t71-t391)+t784.*(t71-t391)).*(-1.0./4.0);
t14640 = (t13578.*(t249-t391.*(1.1e+1./1.25e+2)-t1912.*4.252e-3+t3505+t5357+t693.*(t71-t391)+t784.*(t71-t391)))./4.0;
t14643 = t17.*(t2189+t2495+t2635+t2646+t3580+t9.*(t258+t2289+t5392+t7559)+t17.*(t7693+t9904)).*(-1.13264871585e-2);
t14646 = t17.*(t2189+t2495+t2635+t2646+t3580+t9.*(t258+t2289+t5392+t7559)+t17.*(t7693+t9904)).*1.13264871585e-2;
t14657 = (t10408.*(t2810+t2988-t12589))./2.0;
t14709 = (t8191.*t14035)./4.0;
t14724 = t8477.*(t3625+t3660+t9166-t11658).*(-1.0./4.0);
t14734 = t8640.*(t3625+t3660+t9166-t11658).*(-1.0./4.0);
t14770 = t824+t2543+t2699+t2707+t11661+t11667;
t14781 = (t12042.*t12385)./2.0;
t14782 = (t10850.*(t2810+t2988-t12589))./2.0;
t14800 = (t12050.*t12396)./2.0;
t14805 = -t14801;
t14838 = (t10931.*(t2810+t2988-t12589))./2.0;
t14851 = t5433.*(t2189+t2495+t2635+t2646+t3580+t9.*(t258+t2289+t5392+t7559)+t17.*(t7693+t9904)).*(-1.0./4.0);
t14853 = (t5433.*(t2189+t2495+t2635+t2646+t3580+t9.*(t258+t2289+t5392+t7559)+t17.*(t7693+t9904)))./4.0;
t14868 = -t14865;
t14896 = t17.*(-t2550+t2696+t2698+t11659+t8.*t11672+t147.*(t71-t391)).*(-1.13264871585e-2);
t14900 = (t11228.*(t2810+t2988-t12589))./2.0;
t14916 = -t14914;
t14926 = t9.*t14821.*1.13264871585e-2;
t14927 = t17.*t14823.*1.13264871585e-2;
t14933 = t14035.*(t249-t391.*(1.1e+1./1.25e+2)-t1912.*4.252e-3+t3505+t5357+t693.*(t71-t391)+t784.*(t71-t391)).*(-1.0./4.0);
t14963 = t17.*(t3471+t3796+t3914+t3942+t4358+t9.*(t258+t2289+t5392+t7559).*7.35522e-1+t17.*(t7693+t9904).*7.35522e-1).*(-1.539925e-2);
t14965 = t17.*(t3471+t3796+t3914+t3942+t4358+t9.*(t258+t2289+t5392+t7559).*7.35522e-1+t17.*(t7693+t9904).*7.35522e-1).*1.539925e-2;
t15042 = t3743.*(t3471+t3796+t3914+t3942+t4358+t9.*(t258+t2289+t5392+t7559).*7.35522e-1+t17.*(t7693+t9904).*7.35522e-1).*(-1.0./4.0);
t15045 = (t3743.*(t3471+t3796+t3914+t3942+t4358+t9.*(t258+t2289+t5392+t7559).*7.35522e-1+t17.*(t7693+t9904).*7.35522e-1))./4.0;
t15046 = (t12396.*t12589)./2.0;
t15081 = t10141.*(t3625+t3660+t9166-t11658).*(-1.0./4.0);
t15120 = (t5434.*t14821)./4.0;
t15121 = (t5433.*t14823)./4.0;
t15124 = t7797.*(t2189+t2495+t2635+t2646+t3580+t9.*(t258+t2289+t5392+t7559)+t17.*(t7693+t9904)).*(-1.0./4.0);
t15126 = (t7797.*(t2189+t2495+t2635+t2646+t3580+t9.*(t258+t2289+t5392+t7559)+t17.*(t7693+t9904)))./4.0;
t15136 = (t12049.*(t2810+t2988-t12589))./2.0;
t15155 = t3209+t3253+t3650+t3693+t4033+t10795+t12485;
t15156 = t3214+t3251+t3654+t3667+t4030+t10793+t12489;
t15178 = t5345.*(t3471+t3796+t3914+t3942+t4358+t9.*(t258+t2289+t5392+t7559).*7.35522e-1+t17.*(t7693+t9904).*7.35522e-1).*(-1.0./4.0);
t15180 = (t5345.*(t3471+t3796+t3914+t3942+t4358+t9.*(t258+t2289+t5392+t7559).*7.35522e-1+t17.*(t7693+t9904).*7.35522e-1))./4.0;
t15320 = t6761.*(t3471+t3796+t3914+t3942+t4358+t9.*(t258+t2289+t5392+t7559).*7.35522e-1+t17.*(t7693+t9904).*7.35522e-1).*(-1.0./4.0);
t15324 = (t6761.*(t3471+t3796+t3914+t3942+t4358+t9.*(t258+t2289+t5392+t7559).*7.35522e-1+t17.*(t7693+t9904).*7.35522e-1))./4.0;
t15341 = t7797.*(-t2550+t2696+t2698+t11659+t8.*t11672+t147.*(t71-t391)).*(-1.0./4.0);
t15343 = (t7797.*(-t2550+t2696+t2698+t11659+t8.*t11672+t147.*(t71-t391)))./4.0;
t15375 = (t7796.*t14821)./4.0;
t15376 = (t7797.*t14823)./4.0;
t16112 = t3191+t3236+t3694+t3776+t3783+t3829+t3831+t3907+t3980+t4124+t4167+t4189+t5294+t5363+t5741+t5751+t5849+t5924+t6339+t6359+t7357+t7360+t7604+t7680+t8137+t8319+t8320+t9133;
t16115 = t3741+t3760+t3821+t4764+t4784+t4822+t4925+t4969+t5898+t5931+t6017+t6280+t6513+t6527+t6606+t6930+t6941+t8619+t8633+t8670+t9046+t9062+t9315;
t16125 = t3320+t3361+t3385+t3484+t4641+t4645+t4752+t4763+t4778+t4792+t5930+t5974+t6009+t6057+t6103+t6112+t6162+t6479+t6710+t6711+t6873+t6879+t7287+t7288+t9270+t9277+t9312+t9314+t9712+t9939;
t3377 = t542+t1967;
t3516 = -t3448;
t3521 = -t3452;
t3817 = t2474.*7.35522e-1;
t3819 = t2480.*7.35522e-1;
t4339 = -t4321;
t4341 = -t4324;
t4371 = -t4355;
t4631 = t2474.*3.867742437e-3;
t4668 = t2480.*1.563719772e-3;
t5186 = (t3219.*t3308)./4.0;
t5240 = t3308.*(t689-t740).*(-1.0./4.0);
t5249 = (t3308.*(t689-t740))./4.0;
t5253 = (t3308.*(t1130-t16.*t17.*1.2516e-2))./4.0;
t5257 = -t5243;
t5385 = -t5359;
t5408 = -t5384;
t5588 = -t5570;
t5659 = -t5643;
t5674 = -t5658;
t5701 = -t5687;
t5749 = (t3308.*t4432)./4.0;
t5791 = (t3308.*t4515)./4.0;
t5798 = (t3308.*t4551)./4.0;
t5799 = -t5789;
t5802 = t5359.*7.35522e-1;
t5804 = t5360.*7.35522e-1;
t5823 = t5415.*(-7.35522e-1);
t5830 = t5384.*7.35522e-1;
t5832 = t5386.*7.35522e-1;
t5842 = t5415.*7.35522e-1;
t6217 = -t6204;
t6326 = (t7.*t6251)./4.0;
t6360 = -t6341;
t6363 = (t14.*t15.*t6251)./4.0;
t6367 = t5415.*(-3.867742437e-3);
t6377 = t5386.*3.867742437e-3;
t6387 = t5415.*3.867742437e-3;
t6390 = t5384.*1.563719772e-3;
t6395 = -t6378;
t6396 = -t6380;
t6411 = (t3308.*t5233)./4.0;
t6416 = -t6405;
t6485 = (t321.*t6251)./4.0;
t6495 = -t6488;
t6599 = t6251.*(t71-t391).*(-1.0./2.0);
t6610 = (t3308.*t5481)./4.0;
t6632 = -t6623;
t6670 = (t3308.*t5561)./4.0;
t6732 = -t6719;
t6919 = (t3308.*t5761)./4.0;
t7007 = -t6996;
t7008 = (t3308.*t5837)./4.0;
t7026 = -t7006;
t7031 = -t7011;
t7045 = -t7027;
t7064 = t2530+t2670+t3392+t3483;
t7069 = (t3308.*t5888)./4.0;
t7081 = -t7067;
t7111 = -t7103;
t7114 = (t3308.*t5955)./4.0;
t7129 = t2679+t2691+t3515+t3569;
t7150 = -t7140;
t7195 = (t8.*t7141)./4.0;
t7198 = -t7189;
t7213 = (t15.*t16.*t7141)./4.0;
t7258 = (t3308.*t6188)./4.0;
t7297 = -t7285;
t7394 = (t323.*t7141)./4.0;
t7413 = t8.*t6884.*2.62925e-3;
t7420 = -t7409;
t7464 = -t7455;
t7472 = (t439.*t7141)./4.0;
t7474 = -t7467;
t7476 = -t7471;
t7495 = (t8.*t7440)./4.0;
t7517 = (t15.*t16.*t7440)./4.0;
t7523 = -t7510;
t7533 = t6.*t7510;
t7551 = -t7534;
t7568 = (t16.*t7497)./4.0;
t7572 = (t8.*t7486)./4.0;
t7580 = -t7566;
t7585 = -t7570;
t7595 = (t8.*t15.*t7497)./4.0;
t7596 = -t7582;
t7599 = (t15.*t16.*t7486)./4.0;
t7609 = t7.*t16.*t7497.*(-1.0./4.0);
t7615 = t7.*t8.*t7486.*(-1.0./4.0);
t7629 = -t7611;
t7631 = (t15.*t39.*t7486)./4.0;
t7647 = (t15.*t44.*t7497)./4.0;
t7706 = (t3308.*t6573)./4.0;
t7710 = -t7689;
t7711 = -t7691;
t7712 = -t7692;
t7742 = t8.*t6744.*4.38178973375e-3;
t7746 = -t7725;
t7755 = (t227.*t7497)./4.0;
t7756 = (t228.*t7497)./4.0;
t7762 = (t2501.*t6884)./4.0;
t7768 = (t323.*t7486)./4.0;
t7769 = (t324.*t7486)./4.0;
t7780 = -t7767;
t7781 = t17.*t6811.*1.13264871585e-2;
t7788 = -t7776;
t7809 = (t3308.*t6637)./4.0;
t7810 = (t370.*t7486)./4.0;
t7816 = t16.*t321.*t7497.*(-1.0./4.0);
t7826 = t7141.*(t348-t525).*(-1.0./2.0);
t7827 = t8.*t321.*t7486.*(-1.0./4.0);
t7830 = (t439.*t7440)./2.0;
t7836 = (t404.*t7497)./4.0;
t7842 = (t7141.*(t348-t525))./2.0;
t7860 = -t7849;
t7880 = (t3308.*t6687)./4.0;
t7884 = -t7870;
t7889 = -t7872;
t7898 = -t7878;
t7906 = -t7890;
t7911 = (t439.*t7486)./4.0;
t7925 = t7497.*(t48-t349).*(-1.0./4.0);
t7931 = (t483.*t7486)./4.0;
t7941 = (t7497.*(t48-t349))./4.0;
t7953 = t7497.*(t60-t394).*(-1.0./4.0);
t7971 = (t539.*t7497)./2.0;
t7972 = (t3308.*t6803)./4.0;
t7975 = t16.*t7497.*(t71-t391).*(-1.0./2.0);
t7979 = t8.*t7486.*(t71-t391).*(-1.0./2.0);
t7989 = (t16.*t7497.*(t71-t391))./2.0;
t7991 = (t8.*t7486.*(t71-t391))./2.0;
t7997 = t7486.*(t113-t409).*(-1.0./2.0);
t8004 = (t3308.*t6844)./2.0;
t8014 = (t7486.*(t113-t409))./2.0;
t8029 = -t8010;
t8041 = -t8028;
t8074 = (t604.*t7497)./2.0;
t8090 = -t8071;
t8098 = t7486.*(t380-t392).*(-1.0./2.0);
t8114 = (t7486.*(t380-t392))./2.0;
t8145 = t7440.*(t348-t525).*(-1.0./4.0);
t8154 = (t3732.*t6884)./4.0;
t8157 = (t7440.*(t348-t525))./4.0;
t8162 = t3308.*(t1912.*(-4.28e-4)+t3337+t587.*(t71-t391)+t689.*(t71-t391)).*(-1.0./2.0);
t8174 = (t3308.*(t1912.*(-4.28e-4)+t3337+t587.*(t71-t391)+t689.*(t71-t391)))./2.0;
t8201 = -t8182;
t8212 = (t1840.*t7497)./2.0;
t8216 = -t8198;
t8245 = t1476+t2256+t6938;
t8250 = (t1904.*t7486)./2.0;
t8251 = t7486.*(t348-t525).*(-1.0./2.0);
t8252 = -t8239;
t8276 = t7497.*(t386+t16.*(t69-t347)).*(-1.0./2.0);
t8289 = (t7497.*(t386+t16.*(t69-t347)))./2.0;
t8296 = -t8286;
t8317 = -t8308;
t8343 = -t8334;
t8354 = t17.*t7856.*1.539925e-2;
t8371 = -t8361;
t8395 = (t4298.*t6811)./4.0;
t8451 = -t8446;
t8481 = (t3308.*t7396)./4.0;
t8505 = t8131.*1.225946;
t8511 = (t4489.*t6884)./2.0;
t8512 = t8129.*7.35522e-1;
t8515 = t8128.*1.666555;
t8516 = t8129.*1.666555;
t8517 = t8131.*1.666555;
t8518 = t8132.*1.666555;
t8519 = t8128.*1.225946;
t8523 = t3308.*(t578.*1.2516e-2+t2492-t2628+t2673+t1129.*(t71-t391)).*(-1.0./2.0);
t8525 = (t4498.*t6884)./2.0;
t8527 = -t8521;
t8535 = (t3308.*(t578.*1.2516e-2+t2492-t2628+t2673+t1129.*(t71-t391)))./2.0;
t8546 = -t8531;
t8588 = t1942+t2554+t2674+t2702+t3490+t3652;
t8593 = (t3308.*t7475)./4.0;
t8599 = -t8576;
t8601 = -t8579;
t8602 = -t8580;
t8603 = -t8582;
t8605 = -t8584;
t8608 = -t8589;
t8614 = (t9.*t8530)./4.0;
t8616 = -t8610;
t8617 = -t8611;
t8626 = (t16.*t17.*t8530)./4.0;
t8627 = -t8621;
t8630 = t8.*t9.*t8530.*(-1.0./4.0);
t8631 = -t8625;
t8637 = (t16.*t41.*t8530)./4.0;
t8647 = -t8639;
t8650 = -t8642;
t8654 = t3944+t3965+t4349+t4350;
t8655 = t7.*t8641;
t8662 = t7.*t8648;
t8666 = (t17.*t8622)./4.0;
t8677 = (t9.*t16.*t8622)./4.0;
t8679 = (t229.*t8530)./4.0;
t8680 = (t230.*t8530)./4.0;
t8681 = t8.*t17.*t8622.*(-1.0./4.0);
t8687 = (t16.*t45.*t8622)./4.0;
t8688 = -t8684;
t8701 = t9.*t323.*t8530.*(-1.0./4.0);
t8703 = -t8695;
t8707 = (t405.*t8530)./4.0;
t8716 = t3308.*(t1788+t2251+t2331-t2398+t587.*(t113-t409)+t689.*(t113-t409)).*(-1.0./2.0);
t8720 = t321.*t8641;
t8721 = -t8715;
t8722 = (t3308.*(t1788+t2251+t2331-t2398+t587.*(t113-t409)+t689.*(t113-t409)))./2.0;
t8723 = -t8717;
t8724 = -t8719;
t8725 = t2031+t2474+t2569+t3581+t5386;
t8726 = t321.*t8648;
t8729 = (t325.*t8622)./4.0;
t8730 = (t326.*t8622)./4.0;
t8732 = -t8727;
t8733 = (t5007.*t6884)./2.0;
t8749 = -t8740;
t8752 = (t371.*t8622)./4.0;
t8755 = -t8747;
t8762 = t8530.*(t79-t358).*(-1.0./4.0);
t8763 = t17.*t323.*t8622.*(-1.0./4.0);
t8767 = t9.*t439.*t8530.*(-1.0./4.0);
t8771 = (t8530.*(t79-t358))./4.0;
t8774 = t8131.*7.326866269e-3;
t8781 = t8128.*2.5171736245e-2;
t8785 = t8530.*(t77-t390).*(-1.0./4.0);
t8786 = t8129.*5.01208083475e-2;
t8790 = -t8776;
t8793 = t8132.*1.17633784675e-2;
t8798 = (t8530.*(t77-t390))./4.0;
t8807 = (t540.*t8530)./4.0;
t8814 = -t8801;
t8815 = (t3308.*t7932)./2.0;
t8847 = (t440.*t8622)./4.0;
t8871 = -t8851;
t8881 = (t7128.*(t2904-t2927))./4.0;
t8887 = (t484.*t8622)./4.0;
t8892 = -t8870;
t8895 = (t3743.*t7856)./4.0;
t8899 = -t8876;
t8903 = -t8880;
t8905 = -t8882;
t8909 = t17.*t439.*t8622.*(-1.0./4.0);
t8913 = -t8889;
t8914 = -t8890;
t8915 = -t8894;
t8919 = -t8901;
t8924 = (t605.*t8530)./4.0;
t8926 = t8.*t8562.*2.62925e-3;
t8936 = t8.*t8227.*4.38178973375e-3;
t8939 = -t8930;
t8943 = (t3738.*t7913)./4.0;
t8951 = t8622.*(t106-t414).*(-1.0./4.0);
t8953 = t8.*t8253.*4.38178973375e-3;
t8959 = (t8622.*(t106-t414))./4.0;
t9000 = (t754.*t8622)./4.0;
t9002 = t8530.*(t357-t519).*(-1.0./4.0);
t9003 = (t1907.*t8530)./4.0;
t9006 = (t8530.*(t357-t519))./4.0;
t9011 = t9.*t8530.*(t348-t525).*(-1.0./2.0);
t9013 = -t9010;
t9017 = (t5449.*t6811)./4.0;
t9025 = (t1837.*t8622)./4.0;
t9026 = -t9022;
t9036 = t17.*t8622.*(t348-t525).*(-1.0./2.0);
t9037 = t8.*t8713.*2.62925e-3;
t9038 = t8622.*(t395+t9.*(t48-t349)).*(-1.0./4.0);
t9039 = -t9034;
t9042 = (t2458.*t8530)./2.0;
t9051 = t6.*t8742.*6.8635e-3;
t9052 = -t9044;
t9054 = t8530.*(t383+t9.*(t380-t392)).*(-1.0./2.0);
t9056 = t3005+t3163+t3419+t3773+t5147;
t9060 = (t8530.*(t383+t9.*(t380-t392)))./2.0;
t9066 = (t2612.*t8530)./2.0;
t9067 = (t5365.*t7128)./4.0;
t9070 = (t2418.*t8622)./2.0;
t9081 = -t9077;
t9085 = -t9078;
t9088 = -t9084;
t9089 = (t2482.*t8622)./2.0;
t9097 = (t2522.*t8622)./2.0;
t9114 = -t9107;
t9148 = (t7654.*(t2904-t2927))./4.0;
t9160 = (t3308.*t8506)./2.0;
t9162 = (t3284.*t8530)./2.0;
t9171 = t702+t2550+t2675+t2717+t4700+t4814;
t9175 = t8530.*(t1918+t9.*(t71-t391)).*(-1.0./2.0);
t9179 = -t9173;
t9180 = (t4900.*t7822)./4.0;
t9182 = (t8530.*(t1918+t9.*(t71-t391)))./2.0;
t9193 = (t4939.*t7822)./4.0;
t9194 = t2887+t3158+t7856;
t9198 = -t9192;
t9203 = (t3324.*t8622)./2.0;
t9204 = (t3308.*t8622)./2.0;
t9211 = (t5929.*t6884)./4.0;
t9220 = (t5951.*t6884)./4.0;
t9221 = -t9214;
t9222 = (t5947.*t6884)./4.0;
t9223 = (t2561.*t8742)./4.0;
t9238 = -t9224;
t9242 = -t9229;
t9243 = -t9230;
t9251 = -t9240;
t9254 = t8.*t9226;
t9256 = t16.*t9226;
t9264 = t287+t450+t1804+t2672+t2686+t3465+t3572+t4702;
t9267 = -t9258;
t9274 = -t9265;
t9290 = -t9283;
t9306 = -t9295;
t9324 = (t4024.*t8562)./4.0;
t9339 = (t3254.*t8742)./4.0;
t9340 = -t9329;
t9344 = (t3270.*t8742)./4.0;
t9345 = (t8063.*(t2904-t2927))./4.0;
t9346 = (t3275.*t8742)./4.0;
t9351 = (t4021.*t8600)./4.0;
t9395 = -t9385;
t9412 = (t8741.*(t943-t1091))./4.0;
t9419 = -t9398;
t9421 = -t9399;
t9423 = -t9400;
t9433 = -t9416;
t9438 = -t9418;
t9441 = -t9420;
t9442 = -t9422;
t9447 = -t9434;
t9460 = -t9443;
t9472 = -t9461;
t9474 = t8742.*(t263-t283-t310+t1265).*(-1.0./4.0);
t9475 = -t9462;
t9479 = (t6397.*t6811)./4.0;
t9485 = -t9476;
t9486 = t9.*t8999.*1.13264871585e-2;
t9488 = -t9480;
t9489 = t17.*t9001.*1.13264871585e-2;
t9490 = -t9483;
t9497 = (t5345.*t7856)./4.0;
t9501 = -t9493;
t9513 = -t9507;
t9517 = (t5329.*t7913)./4.0;
t9519 = t9.*t9185.*1.539925e-2;
t9532 = (t5069.*t8227)./4.0;
t9543 = (t5442.*t7822)./4.0;
t9546 = -t9535;
t9548 = -t9539;
t9553 = t9244.*7.35522e-1;
t9554 = t9245.*7.35522e-1;
t9556 = t9247.*7.35522e-1;
t9557 = t9248.*7.35522e-1;
t9562 = t9255.*1.666555;
t9564 = t9255.*7.35522e-1;
t9566 = t9253.*1.666555;
t9581 = -t9575;
t9612 = (t5365.*t8063)./4.0;
t9620 = (t4252.*t8742)./4.0;
t9622 = -t9613;
t9634 = (t2054.*t9185)./4.0;
t9654 = -t9647;
t9656 = -t9648;
t9662 = -t9651;
t9664 = -t9653;
t9674 = -t9670;
t9679 = -t9672;
t9680 = -t9673;
t9681 = -t9675;
t9691 = -t9688;
t9695 = (t6729.*t6884)./4.0;
t9697 = (t5430.*t8227)./4.0;
t9699 = (t4557.*t8742)./4.0;
t9705 = (t4569.*t8742)./4.0;
t9709 = (t6744.*t6872)./4.0;
t9711 = (t6780.*t6811)./4.0;
t9718 = (t4611.*t8742)./4.0;
t9737 = (t3743.*t9050)./4.0;
t9743 = t3032+t3204+t3415+t3593+t3873+t5226;
t9744 = t3176+t3494+t8562;
t9747 = t6864+t6887;
t9748 = t3045+t3595+t8563;
t9751 = -t9742;
t9759 = -t9750;
t9761 = -t9752;
t9762 = -t9754;
t9765 = -t9757;
t9766 = -t9758;
t9767 = t9560.*7.35522e-1;
t9768 = t9561.*7.35522e-1;
t9770 = -t9760;
t9771 = t9244.*3.867742437e-3;
t9772 = t9245.*3.867742437e-3;
t9777 = -t9769;
t9778 = t9247.*1.563719772e-3;
t9779 = t9248.*1.563719772e-3;
t9783 = t9255.*5.01208083475e-2;
t9787 = -t9775;
t9788 = -t9776;
t9789 = t9.*t9537.*1.539925e-2;
t9794 = -t9781;
t9800 = t7.*t9226.*1.059103943995e-1;
t9804 = -t9790;
t9806 = t6884.*(-t1540+t2091+t2579+t8.*(t260+t468+t570+t2298)).*(-1.0./4.0);
t9808 = t9253.*1.17633784675e-2;
t9813 = -t9799;
t9818 = (t6884.*(-t1540+t2091+t2579+t8.*(t260+t468+t570+t2298)))./4.0;
t9823 = -t9811;
t9832 = -t9821;
t9834 = (t5235.*t8562)./4.0;
t9837 = -t9824;
t9839 = -t9827;
t9841 = (t6884.*t6995)./4.0;
t9844 = -t9835;
t9845 = -t9836;
t9853 = -t9847;
t9856 = (t5234.*t8600)./4.0;
t9857 = -t9849;
t9867 = -t9858;
t9868 = -t9859;
t9885 = t17.*(t3452-t4730+t5359+t9.*(t71-t391).*6.1597e-2+t17.*(t426-t581)).*(-1.13264871585e-2);
t9895 = t17.*(t3452-t4730+t5359+t9.*(t71-t391).*6.1597e-2+t17.*(t426-t581)).*1.13264871585e-2;
t9913 = -t9908;
t9920 = -t9918;
t9923 = (t3767.*t9185)./4.0;
t9942 = (t5235.*t8713)./4.0;
t9949 = -t9943;
t9955 = (t5914.*t8227)./4.0;
t9956 = (t6385.*t7822)./4.0;
t9958 = (t5919.*t8227)./4.0;
t9985 = -t9979;
t9989 = -t9982;
t9990 = t16.*t9717.*2.62925e-3;
t9991 = t9560.*3.867742437e-3;
t9999 = t9561.*1.563719772e-3;
t10004 = -t9997;
t10018 = (t6046.*t8253)./4.0;
t10022 = t15.*t9732.*8.639075e-2;
t10023 = t15.*t9733.*8.639075e-2;
t10024 = -t10014;
t10029 = t7.*t9746.*8.639075e-2;
t10039 = -t10027;
t10047 = -t10035;
t10050 = -t10037;
t10051 = -t10038;
t10069 = -t10062;
t10073 = -t10065;
t10116 = -t10112;
t10117 = -t10113;
t10119 = -t10115;
t10122 = t17.*t9887.*1.539925e-2;
t10125 = t9.*t9896.*1.539925e-2;
t10128 = (t6811.*t7538)./4.0;
t10136 = (t4517.*t9185)./4.0;
t10147 = t6461+t8128;
t10153 = t6505+t8131;
t10163 = (t4772.*t9185)./4.0;
t10170 = t2148+t2513+t2649+t2661+t3582+t4697+t5395;
t10180 = t2189+t2495+t2635+t2646+t3580+t4693+t5415;
t10188 = t8.*t10164;
t10189 = t9.*t10164;
t10191 = t16.*t10164;
t10192 = t17.*t10164;
t10199 = t6466+t8269;
t10202 = -t10195;
t10203 = t9.*t10182;
t10204 = t17.*t10182;
t10211 = -t10205;
t10212 = (t6761.*t7856)./2.0;
t10213 = (t6811.*t7828)./2.0;
t10216 = t8.*t10208;
t10217 = t8.*t10209;
t10222 = (t5713.*t8741)./4.0;
t10225 = -t10220;
t10229 = -t10223;
t10235 = -t10226;
t10238 = -t10234;
t10239 = (t5434.*t8999)./4.0;
t10246 = -t10241;
t10247 = (t5433.*t9001)./4.0;
t10252 = -t10242;
t10254 = -t10245;
t10259 = -t10248;
t10260 = -t10250;
t10261 = (t6811.*t7913)./2.0;
t10262 = -t10251;
t10266 = (t6969.*t7822)./4.0;
t10274 = -t10264;
t10275 = -t10265;
t10282 = -t10278;
t10283 = -t10279;
t10286 = -t10281;
t10290 = (t3249.*t9727)./4.0;
t10291 = (t3249.*t9728)./4.0;
t10301 = (t5345.*t9050)./4.0;
t10305 = -t10303;
t10316 = -t10311;
t10326 = -t10317;
t10342 = (t6681.*t8227)./4.0;
t10343 = -t10333;
t10345 = -t10336;
t10355 = -t10347;
t10365 = (t5217.*t9185)./4.0;
t10371 = (t3752.*t9727)./4.0;
t10372 = (t3752.*t9728)./4.0;
t10420 = (t6884.*t8178)./4.0;
t10421 = (t7217.*t7822)./4.0;
t10436 = t10218.*(-7.35522e-1);
t10440 = -t10430;
t10443 = t10218.*7.35522e-1;
t10448 = (t6190.*t8741)./4.0;
t10450 = (t4021.*t9717)./4.0;
t10452 = t10232.*(-7.35522e-1);
t10456 = (t6872.*t8253)./4.0;
t10459 = -t10451;
t10460 = t10232.*7.35522e-1;
t10462 = -t10454;
t10474 = (t3743.*t9887)./4.0;
t10476 = -t10471;
t10480 = t3053+t3225+t3339+t3551+t3851+t4391+t5111;
t10481 = (t3738.*t9896)./4.0;
t10485 = t3160+t3168+t3345+t3478+t3898+t4420+t5113;
t10487 = -t10482;
t10490 = t2714+t3899+t3939+t3996+t5208+t5255;
t10495 = -t10493;
t10497 = (t3265.*t9967)./4.0;
t10509 = -t10503;
t10517 = (t3360.*t9967)./4.0;
t10523 = -t10516;
t10530 = -t10520;
t10533 = -t10528;
t10534 = -t10529;
t10540 = (t6811.*t8460)./2.0;
t10576 = (t3771.*t9967)./4.0;
t10577 = t6809+t8597;
t10581 = -t10573;
t10586 = t6804+t8591;
t10588 = t6826+t8574;
t10591 = t5433.*(t3452-t4730+t5359+t9.*(t71-t391).*6.1597e-2+t17.*(t426-t581)).*(-1.0./4.0);
t10595 = t6824+t8594;
t10596 = t17.*(t1987-t2621+t3452-t4730+t5359+t9.*(t71-t391).*6.1597e-2+t17.*(t426-t581)).*(-1.13264871585e-2);
t10597 = t6841+t8578;
t10599 = (t5433.*(t3452-t4730+t5359+t9.*(t71-t391).*6.1597e-2+t17.*(t426-t581)))./4.0;
t10606 = t17.*(t1987-t2621+t3452-t4730+t5359+t9.*(t71-t391).*6.1597e-2+t17.*(t426-t581)).*1.13264871585e-2;
t10615 = (t5719.*t9185)./2.0;
t10616 = (t7676.*t7822)./4.0;
t10632 = t7.*t10164.*1.059103943995e-1;
t10655 = t10218.*(-1.563719772e-3);
t10656 = (t3421.*t10111)./4.0;
t10660 = t8.*t10182.*4.38178973375e-3;
t10662 = (t5760.*t9185)./2.0;
t10667 = -t10646;
t10674 = -t10653;
t10675 = t8.*t10218.*(-3.867742437e-3);
t10677 = -t10654;
t10678 = t10218.*1.563719772e-3;
t10680 = (t3489.*t10111)./4.0;
t10685 = t10232.*(-1.563719772e-3);
t10687 = -t10676;
t10690 = t10232.*1.563719772e-3;
t10706 = -t10697;
t10713 = (t7128.*t8477)./4.0;
t10719 = (t7815.*t7822)./2.0;
t10720 = (t7815.*t7822)./4.0;
t10724 = -t10714;
t10725 = -t10717;
t10728 = t17.*t10468.*1.539925e-2;
t10730 = t9.*t10469.*1.539925e-2;
t10731 = (t5329.*t9537)./4.0;
t10744 = -t10737;
t10749 = (t7116.*t8562)./4.0;
t10751 = (t7079.*t8600)./4.0;
t10756 = t9.*(t2740+t3849+t3968+t3972-t5255+t17.*(t260+t468+t570+t2298).*7.35522e-1).*(-1.539925e-2);
t10757 = t17.*(-t3823+t3970+t5243+t9.*(t260+t468+t570+t2298).*7.35522e-1+t972.*(t71-t391)+t2777.*(t71-t391)).*(-1.539925e-2);
t10762 = t9.*(t2740+t3849+t3968+t3972-t5255+t17.*(t260+t468+t570+t2298).*7.35522e-1).*1.539925e-2;
t10771 = (t6038.*t9185)./2.0;
t10777 = (t4453.*t9967)./4.0;
t10779 = -t10774;
t10784 = (t7128.*t8640)./4.0;
t10785 = -t10781;
t10788 = (t7622.*t8227)./4.0;
t10789 = (t7612.*t8227)./4.0;
t10800 = -t10792;
t10803 = (t2054.*t10469)./4.0;
t10805 = (t7822.*(t917-t1669+t2469+t2475+t3495+t3591))./4.0;
t10806 = (t2044.*t10468)./4.0;
t10808 = (t3489.*t10240)./4.0;
t10813 = -t10812;
t10814 = (t5234.*t9717)./4.0;
t10818 = -t10816;
t10827 = (t7116.*t8713)./4.0;
t10836 = -t10831;
t10839 = t15.*(t6806-t8574).*(-8.639075e-2);
t10843 = t15.*(t6806-t8574).*8.639075e-2;
t10851 = -t10845;
t10857 = t4298.*(t1987-t2621+t3452-t4730+t5359+t9.*(t71-t391).*6.1597e-2+t17.*(t426-t581)).*(-1.0./4.0);
t10861 = (t4298.*(t1987-t2621+t3452-t4730+t5359+t9.*(t71-t391).*6.1597e-2+t17.*(t426-t581)))./4.0;
t10865 = -t10860;
t10885 = (t7654.*t8477)./4.0;
t10894 = t9.*t10753.*1.539925e-2;
t10907 = t17.*t10763.*1.539925e-2;
t10920 = t8132+t8185;
t10923 = (t8070.*t8227)./4.0;
t10927 = (t6526.*t9185)./2.0;
t10929 = (t6761.*t9050)./4.0;
t10936 = t8129+t8220;
t10944 = (t6811.*t9048)./2.0;
t10952 = t6811.*(t3085-t3419-t3773+t5128+t17.*(t208-t427).*7.35522e-1).*(-1.0./4.0);
t10953 = -t10949;
t10955 = t6504+t9253;
t10958 = (t6811.*(t3085-t3419-t3773+t5128+t17.*(t208-t427).*7.35522e-1))./4.0;
t10961 = t9.*t10787.*1.539925e-2;
t10969 = (t5628.*t9732)./4.0;
t10970 = (t5628.*t9733)./4.0;
t10972 = t15.*t7822.*(t4542-t6448).*(-4.1663875e-1);
t10973 = t6517+t9255;
t10983 = t15.*t7822.*(t4542-t6448).*4.1663875e-1;
t10984 = -t10975;
t10986 = (t5634.*t9746)./4.0;
t10988 = t9.*(t9253-t44.*(t4540+t5.*(t2425-t2468)));
t10990 = t17.*(t9253-t44.*(t4540+t5.*(t2425-t2468)));
t10991 = (t6744.*t9112)./4.0;
t10994 = t15.*t7822.*(t6460-t35.*(t2425-t2468)).*4.1663875e-1;
t10995 = (t7654.*t8640)./4.0;
t10996 = t8226+t8254;
t11006 = t9.*t10974;
t11008 = t17.*t10974;
t11010 = (t3767.*t10469)./4.0;
t11013 = (t3763.*t10468)./4.0;
t11022 = (t5275.*t9967)./4.0;
t11031 = (t7822.*(t2433+t2449-t3048-t3102+t3223+t3232))./4.0;
t11040 = t2980.*(t6806-t8574).*(-1.0./4.0);
t11045 = (t2980.*(t6806-t8574))./4.0;
t11058 = t3249.*(t6801-t8594).*(-1.0./4.0);
t11063 = (t3249.*(t6801-t8594))./4.0;
t11064 = t3265.*(t6801-t8594).*(-1.0./4.0);
t11065 = -t11061;
t11068 = (t3265.*(t6801-t8594))./4.0;
t11072 = (t8063.*t8477)./4.0;
t11081 = t3360.*(t6801-t8594).*(-1.0./4.0);
t11085 = (t3360.*(t6801-t8594))./4.0;
t11106 = -t11099;
t11107 = -t11100;
t11124 = -t11119;
t11125 = t3771.*(t6801-t8594).*(-1.0./4.0);
t11126 = (t5518.*t9967)./4.0;
t11128 = t3752.*(t6801-t8594).*(-1.0./4.0);
t11133 = (t5523.*t9967)./4.0;
t11135 = (t3771.*(t6801-t8594))./4.0;
t11138 = (t3752.*(t6801-t8594))./4.0;
t11141 = (t5543.*t9967)./4.0;
t11144 = t10948.*7.35522e-1;
t11147 = t10947.*1.666555;
t11149 = t10948.*1.666555;
t11163 = (t5216.*t10164)./4.0;
t11166 = -t11153;
t11171 = -t11159;
t11175 = (t4474.*t10468)./4.0;
t11176 = t8227.*(-t3218+t3458+t3878+t8.*(t260+t468+t570+t2298).*1.666555).*(-1.0./2.0);
t11180 = (t8227.*(-t3218+t3458+t3878+t8.*(t260+t468+t570+t2298).*1.666555))./2.0;
t11182 = t8562.*(-t1476-t1540+t2091+t2165+t2579+t8.*(t260+t468+t570+t2298)).*(-1.0./2.0);
t11189 = (t7822.*t8791)./2.0;
t11190 = (t4517.*t10469)./4.0;
t11195 = -t11193;
t11196 = (t8227.*t8600)./2.0;
t11199 = t7822.*(t5144-t6902).*(-1.0./4.0);
t11209 = (t7822.*(t5144-t6902))./4.0;
t11210 = -t11202;
t11211 = t4064.*(t6806-t8574).*(-1.0./4.0);
t11212 = -t11204;
t11219 = (t6811.*t9361)./4.0;
t11233 = -t11224;
t11235 = (t7822.*t8927)./4.0;
t11236 = (t4772.*t10469)./4.0;
t11240 = (t4798.*t10468)./4.0;
t11245 = (t3738.*t10753)./4.0;
t11253 = t4255.*(t6806-t8574).*(-1.0./4.0);
t11258 = t4286.*(t6806-t8574).*(-1.0./4.0);
t11260 = (t4255.*(t6806-t8574))./4.0;
t11261 = (t3743.*t10763)./4.0;
t11267 = (t4286.*(t6806-t8574))./4.0;
t11275 = -t11264;
t11283 = (t7796.*t8999)./4.0;
t11285 = t5449.*(t1987-t2621+t3452-t4730+t5359+t9.*(t71-t391).*6.1597e-2+t17.*(t426-t581)).*(-1.0./4.0);
t11294 = (t5449.*(t1987-t2621+t3452-t4730+t5359+t9.*(t71-t391).*6.1597e-2+t17.*(t426-t581)))./4.0;
t11297 = (t7856.*t8981)./4.0;
t11298 = (t7797.*t9001)./4.0;
t11303 = (t5443.*t10164)./4.0;
t11311 = (t5696.*t10111)./4.0;
t11313 = (t7913.*t8979)./4.0;
t11319 = (t8227.*t8709)./2.0;
t11321 = (t3738.*t10787)./4.0;
t11322 = t4453.*(t6801-t8594).*(-1.0./4.0);
t11327 = t8713.*(-t1476-t1540+t2091+t2165+t2579+t8.*(t260+t468+t570+t2298)).*(-1.0./2.0);
t11328 = -t11318;
t11330 = (t4453.*(t6801-t8594))./4.0;
t11332 = (t7348.*t9185)./4.0;
t11334 = -t11326;
t11339 = (t6811.*t9537)./4.0;
t11348 = t7542+t9134;
t11349 = t7546+t9136;
t11353 = -t11347;
t11359 = t8742.*(t263+t1265-t7252-t5.*t12.*1.0442e-1).*(-1.0./4.0);
t11373 = t10948.*5.01208083475e-2;
t11378 = t10947.*1.17633784675e-2;
t11379 = (t5635.*t10164)./4.0;
t11390 = t8587+t8595;
t11391 = -t11383;
t11410 = (t9967.*(-t1272-t1479+t1647+t1848+t2236))./4.0;
t11411 = (t3421.*t10863)./4.0;
t11412 = t8.*(t9253-t44.*(t4540+t5.*(t2425-t2468))).*4.38178973375e-3;
t11423 = (t3489.*t10863)./4.0;
t11427 = t8.*t10974.*4.38178973375e-3;
t11434 = (t6589.*t9727)./4.0;
t11435 = (t6589.*t9728)./4.0;
t11436 = (t6193.*t9967)./2.0;
t11437 = (t6193.*t9967)./4.0;
t11438 = ((t701-t775).*(t1589-t2213+t3195-t4346+t4355+t4748.*7.35522e-1+t2772.*(t71-t391)+t2775.*(t71-t391)))./4.0;
t11442 = t4837.*(t6806-t8574).*(-1.0./4.0);
t11446 = (t4837.*(t6806-t8574))./4.0;
t11448 = (t5213.*t10468)./4.0;
t11449 = (t5217.*t10469)./4.0;
t11452 = t3365.*(t1589-t2213+t3195-t4346+t4355+t4748.*7.35522e-1+t2772.*(t71-t391)+t2775.*(t71-t391)).*(-1.0./4.0);
t11454 = t3455.*(t1589-t2213+t3195-t4346+t4355+t4748.*7.35522e-1+t2772.*(t71-t391)+t2775.*(t71-t391)).*(-1.0./4.0);
t11455 = (t3365.*(t1589-t2213+t3195-t4346+t4355+t4748.*7.35522e-1+t2772.*(t71-t391)+t2775.*(t71-t391)))./4.0;
t11456 = (t3455.*(t1589-t2213+t3195-t4346+t4355+t4748.*7.35522e-1+t2772.*(t71-t391)+t2775.*(t71-t391)))./4.0;
t11457 = (t7822.*t9104)./2.0;
t11460 = (t5696.*t10240)./4.0;
t11483 = t3543+t3820+t3911+t3949+t4360+t5199+t5820;
t11486 = t6744.*(-t3045-t3218+t3458+t3539+t3878+t8.*(t260+t468+t570+t2298).*1.666555).*(-1.0./2.0);
t11491 = -t11487;
t11492 = (t9185.*(t2056+t2203+t2351+t3433+t3503+t16.*t389.*(1.1e+1./1.25e+2)))./4.0;
t11501 = t5329.*(t2740+t3849+t3968+t3972-t5255+t17.*(t260+t468+t570+t2298).*7.35522e-1).*(-1.0./4.0);
t11503 = t5095.*(t6806-t8574).*(-1.0./4.0);
t11505 = -t11498;
t11507 = (t5095.*(t6806-t8574))./4.0;
t11509 = t5345.*(-t3823+t3970+t5243+t9.*(t260+t468+t570+t2298).*7.35522e-1+t972.*(t71-t391)+t2777.*(t71-t391)).*(-1.0./4.0);
t11520 = -t11516;
t11521 = (t6046.*t10182)./4.0;
t11544 = (t6535.*t9967)./2.0;
t11546 = (t9746.*(t921+t1317-t5853))./4.0;
t11555 = (t7940.*t9185)./4.0;
t11560 = t4152.*(t1589-t2213+t3195-t4346+t4355+t4748.*7.35522e-1+t2772.*(t71-t391)+t2775.*(t71-t391)).*(-1.0./4.0);
t11566 = (t6175.*t10164)./4.0;
t11570 = (t7039.*t9732)./4.0;
t11571 = (t7039.*t9733)./4.0;
t11573 = (t4152.*(t1589-t2213+t3195-t4346+t4355+t4748.*7.35522e-1+t2772.*(t71-t391)+t2775.*(t71-t391)))./4.0;
t11574 = t7.*t11344.*8.639075e-2;
t11577 = -t11564;
t11580 = (t6196.*t10164)./4.0;
t11582 = (t6761.*t9887)./4.0;
t11590 = (t7982.*t9185)./4.0;
t11592 = t5275.*(t6801-t8594).*(-1.0./4.0);
t11604 = t16.*(t8589-t8592).*(-2.62925e-3);
t11606 = (t8227.*t9098)./4.0;
t11607 = (t6811.*t9896)./4.0;
t11609 = t7797.*(t3452-t4730+t5359+t9.*(t71-t391).*6.1597e-2+t17.*(t426-t581)).*(-1.0./4.0);
t11610 = t16.*(t8589-t8592).*2.62925e-3;
t11614 = (t7797.*(t3452-t4730+t5359+t9.*(t71-t391).*6.1597e-2+t17.*(t426-t581)))./4.0;
t11615 = (t8742.*(-t262+t1056+t1250+t5078+t5282+t4.*t13.*1.0442e-1))./4.0;
t11617 = -t11611;
t11625 = (t5679.*t10468)./4.0;
t11631 = (t7822.*t9333)./4.0;
t11634 = -t11627;
t11637 = (t6654.*t9967)./4.0;
t11638 = (t5719.*t10469)./4.0;
t11639 = t6397.*(t1987-t2621+t3452-t4730+t5359+t9.*(t71-t391).*6.1597e-2+t17.*(t426-t581)).*(-1.0./4.0);
t11642 = -t11635;
t11647 = (t6397.*(t1987-t2621+t3452-t4730+t5359+t9.*(t71-t391).*6.1597e-2+t17.*(t426-t581)))./4.0;
t11648 = -t11640;
t11670 = (t8050.*t9226)./4.0;
t11673 = -t11663;
t11674 = -t11664;
t11680 = (t5760.*t10469)./4.0;
t11684 = (t5782.*t10468)./4.0;
t11689 = (t6302.*t10240)./4.0;
t11699 = -t11691;
t11707 = -t11700;
t11710 = -t11704;
t11716 = t5518.*(t6801-t8594).*(-1.0./4.0);
t11719 = t5523.*(t6801-t8594).*(-1.0./4.0);
t11723 = (t5518.*(t6801-t8594))./4.0;
t11727 = (t5523.*(t6801-t8594))./4.0;
t11729 = t5543.*(t6801-t8594).*(-1.0./4.0);
t11735 = (t4884.*t10871)./4.0;
t11739 = (t5543.*(t6801-t8594))./4.0;
t11751 = (t8742.*t8931)./4.0;
t11752 = (t7822.*t9525)./2.0;
t11757 = t5634.*(t6806-t8574).*(-1.0./4.0);
t11761 = (t6970.*t9967)./2.0;
t11765 = t5628.*(t6806-t8574).*(-1.0./4.0);
t11771 = (t6552.*t10164)./4.0;
t11772 = t5648.*(t6806-t8574).*(-1.0./4.0);
t11775 = (t5628.*(t6806-t8574))./4.0;
t11782 = (t8227.*(t3098+t3199+t3211-t3221+t3678+t4612))./2.0;
t11788 = (t6016.*t10468)./4.0;
t11795 = (t6038.*t10469)./4.0;
t11800 = t5699.*(t6801-t8594).*(-1.0./4.0);
t11804 = -t11794;
t11811 = -t11798;
t11812 = (t5699.*(t6801-t8594))./4.0;
t11820 = (t5329.*t10787)./4.0;
t11821 = (t7080.*t9967)./2.0;
t11822 = t4964.*(t1589-t2213+t3195-t4346+t4355+t4748.*7.35522e-1+t2772.*(t71-t391)+t2775.*(t71-t391)).*(-1.0./4.0);
t11858 = t5853.*(t6806-t8574).*(-1.0./4.0);
t11866 = t5860.*(t6806-t8574).*(-1.0./4.0);
t11867 = -t11857;
t11872 = -t11861;
t11874 = -t11863;
t11882 = t6780.*(t1987-t2621+t3452-t4730+t5359+t9.*(t71-t391).*6.1597e-2+t17.*(t426-t581)).*(-1.0./4.0);
t11886 = -t11881;
t11887 = (t6780.*(t1987-t2621+t3452-t4730+t5359+t9.*(t71-t391).*6.1597e-2+t17.*(t426-t581)))./4.0;
t11890 = t3421.*(t8582-t8586).*(-1.0./4.0);
t11892 = t3489.*(t8582-t8586).*(-1.0./4.0);
t11894 = (t3421.*(t8582-t8586))./4.0;
t11896 = t5999.*(t6806-t8574).*(-1.0./4.0);
t11906 = (t6872.*t10182)./4.0;
t11909 = t5290.*(t1589-t2213+t3195-t4346+t4355+t4748.*7.35522e-1+t2772.*(t71-t391)+t2775.*(t71-t391)).*(-1.0./4.0);
t11911 = t16.*t6884.*(t6452-t8229).*(-1.0./4.0);
t11916 = (t5290.*(t1589-t2213+t3195-t4346+t4355+t4748.*7.35522e-1+t2772.*(t71-t391)+t2775.*(t71-t391)))./4.0;
t11918 = (t16.*t6884.*(t6452-t8229))./4.0;
t11919 = (t7822.*t9727)./4.0;
t11920 = (t7822.*t9728)./4.0;
t11921 = -t11912;
t11929 = (t6801-t8594).*(-t1272-t1479+t1647+t1848+t2236).*(-1.0./4.0);
t11931 = ((t6801-t8594).*(-t1272-t1479+t1647+t1848+t2236))./4.0;
t11933 = (t7128.*t10141)./4.0;
t11941 = t6193.*(t6801-t8594).*(-1.0./4.0);
t11945 = (t6193.*(t6801-t8594))./4.0;
t11955 = (t6526.*t10469)./4.0;
t11956 = t6884.*(t8315+t8.*(t30.*(t2425-t2468)+t68.*(t2425-t2468))).*(-1.0./4.0);
t11957 = -t11952;
t11958 = (t6540.*t10468)./4.0;
t11960 = (t7113.*t10164)./4.0;
t11961 = -t11953;
t11965 = (t8981.*t9050)./2.0;
t11966 = (t6884.*(t8315+t8.*(t30.*(t2425-t2468)+t68.*(t2425-t2468))))./4.0;
t11972 = (t4255.*t11344)./4.0;
t11973 = -t11964;
t11982 = -t11979;
t12004 = t5524.*(t1589-t2213+t3195-t4346+t4355+t4748.*7.35522e-1+t2772.*(t71-t391)+t2775.*(t71-t391)).*(-1.0./4.0);
t12011 = (t5524.*(t1589-t2213+t3195-t4346+t4355+t4748.*7.35522e-1+t2772.*(t71-t391)+t2775.*(t71-t391)))./4.0;
t12015 = -t12008;
t12017 = t5552.*(t1589-t2213+t3195-t4346+t4355+t4748.*7.35522e-1+t2772.*(t71-t391)+t2775.*(t71-t391)).*(-1.0./4.0);
t12019 = (t5696.*t10863)./4.0;
t12020 = -t12014;
t12022 = (t5552.*(t1589-t2213+t3195-t4346+t4355+t4748.*7.35522e-1+t2772.*(t71-t391)+t2775.*(t71-t391)))./4.0;
t12026 = -t12024;
t12033 = (t8227.*t9717)./2.0;
t12046 = t8253.*(-t3045-t3218+t3458+t3539+t3878+t8.*(t260+t468+t570+t2298).*1.666555).*(-1.0./2.0);
t12048 = (t8253.*(-t3045-t3218+t3458+t3539+t3878+t8.*(t260+t468+t570+t2298).*1.666555))./2.0;
t12052 = t6535.*(t6801-t8594).*(-1.0./4.0);
t12054 = -t12051;
t12059 = (t7822.*t9992)./2.0;
t12060 = (t7875.*t9967)./2.0;
t12062 = t6761.*(-t3823+t3970+t5243+t9.*(t260+t468+t570+t2298).*7.35522e-1+t972.*(t71-t391)+t2777.*(t71-t391)).*(-1.0./4.0);
t12063 = (t6761.*(-t3823+t3970+t5243+t9.*(t260+t468+t570+t2298).*7.35522e-1+t972.*(t71-t391)+t2777.*(t71-t391)))./4.0;
t12066 = t6589.*(t6801-t8594).*(-1.0./4.0);
t12067 = t11970.*(-7.35522e-1);
t12069 = t6811.*(t2740+t3849+t3968+t3972-t5255+t17.*(t260+t468+t570+t2298).*7.35522e-1).*(-1.0./4.0);
t12071 = (t6589.*(t6801-t8594))./4.0;
t12073 = t11970.*7.35522e-1;
t12074 = (t6811.*(t2740+t3849+t3968+t3972-t5255+t17.*(t260+t468+t570+t2298).*7.35522e-1))./4.0;
t12087 = t7538.*(t1987-t2621+t3452-t4730+t5359+t9.*(t71-t391).*6.1597e-2+t17.*(t426-t581)).*(-1.0./4.0);
t12088 = (t7538.*(t1987-t2621+t3452-t4730+t5359+t9.*(t71-t391).*6.1597e-2+t17.*(t426-t581)))./4.0;
t12090 = (t7654.*t10141)./4.0;
t12091 = t6654.*(t6801-t8594).*(-1.0./4.0);
t12094 = (t6654.*(t6801-t8594))./4.0;
t12104 = -t12103;
t12111 = -t12110;
t12112 = t6096.*(t1589-t2213+t3195-t4346+t4355+t4748.*7.35522e-1+t2772.*(t71-t391)+t2775.*(t71-t391)).*(-1.0./4.0);
t12116 = (t6096.*(t1589-t2213+t3195-t4346+t4355+t4748.*7.35522e-1+t2772.*(t71-t391)+t2775.*(t71-t391)))./4.0;
t12119 = t15.*t9967.*(t4542-t6448).*(-1.0./4.0);
t12122 = (t15.*t9967.*(t4542-t6448))./4.0;
t12124 = (t15.*t9967.*(t6460-t35.*(t2425-t2468)))./4.0;
t12125 = t6158.*(t1589-t2213+t3195-t4346+t4355+t4748.*7.35522e-1+t2772.*(t71-t391)+t2775.*(t71-t391)).*(-1.0./4.0);
t12130 = (t6158.*(t1589-t2213+t3195-t4346+t4355+t4748.*7.35522e-1+t2772.*(t71-t391)+t2775.*(t71-t391)))./4.0;
t12133 = (t8213.*t9967)./4.0;
t12137 = t7828.*(t1987-t2621+t3452-t4730+t5359+t9.*(t71-t391).*6.1597e-2+t17.*(t426-t581)).*(-1.0./4.0);
t12138 = (t6046.*(t9253-t44.*(t4540+t5.*(t2425-t2468))))./4.0;
t12140 = (t6302.*t10863)./4.0;
t12143 = (t7828.*(t1987-t2621+t3452-t4730+t5359+t9.*(t71-t391).*6.1597e-2+t17.*(t426-t581)))./4.0;
t12159 = t6970.*(t6801-t8594).*(-1.0./4.0);
t12162 = t6988.*(t6806-t8574).*(-1.0./4.0);
t12168 = (t6806-t8574).*(t921+t1317-t5853).*(-1.0./4.0);
t12171 = t9967.*(t4654+t15.*(t4650+t34.*(t2425-t2468))).*(-1.0./4.0);
t12173 = -t12167;
t12175 = t7913.*(t1987-t2621+t3452-t4730+t5359+t9.*(t71-t391).*6.1597e-2+t17.*(t426-t581)).*(-1.0./4.0);
t12178 = ((-t2149+t2205+t693.*(t48-t349)+t784.*(t48-t349)).*(t1589-t2213+t3195-t4346+t4355+t4748.*7.35522e-1+t2772.*(t71-t391)+t2775.*(t71-t391)))./4.0;
t12182 = (t7913.*(t1987-t2621+t3452-t4730+t5359+t9.*(t71-t391).*6.1597e-2+t17.*(t426-t581)))./4.0;
t12183 = t7039.*(t6806-t8574).*(-1.0./4.0);
t12187 = t5234.*(t8589-t8592).*(-1.0./4.0);
t12189 = (t7039.*(t6806-t8574))./4.0;
t12193 = (t8979.*t9537)./2.0;
t12198 = (t7348.*t10469)./2.0;
t12200 = t10164.*(t2437+t2648+t3129+t3384+t3574).*(-1.0./4.0);
t12201 = t9185.*(-t2550+t2696+t2698+t4771+t9.*(t260+t468+t570+t2298)+t147.*(t71-t391)).*(-1.0./4.0);
t12202 = -t12195;
t12204 = t7080.*(t6801-t8594).*(-1.0./4.0);
t12207 = (t9185.*(-t2550+t2696+t2698+t4771+t9.*(t260+t468+t570+t2298)+t147.*(t71-t391)))./4.0;
t12208 = t10468.*(t1468-t1988-t2498+t4565+t17.*(t208-t427)).*(-1.0./2.0);
t12210 = (t7080.*(t6801-t8594))./4.0;
t12216 = -t12209;
t12219 = t11970.*(-1.563719772e-3);
t12222 = -t12215;
t12224 = t11970.*1.563719772e-3;
t12225 = (t8191.*t10111)./2.0;
t12226 = (t8063.*t10141)./2.0;
t12227 = (t6761.*t10763)./4.0;
t12230 = (t8742.*t9685)./4.0;
t12233 = (t9185.*t9197)./4.0;
t12237 = (t6811.*t10753)./4.0;
t12248 = ((t624+t2511-t3502-t9.*t439.*4.252e-3).*(t1589-t2213+t3195-t4346+t4355+t4748.*7.35522e-1+t2772.*(t71-t391)+t2775.*(t71-t391)))./4.0;
t12256 = (t8044.*t10164)./4.0;
t12258 = (t8047.*t10164)./4.0;
t12261 = (t8050.*t10164)./4.0;
t12263 = (t8054.*t10164)./4.0;
t12273 = -t12267;
t12289 = (t9226.*(t2810+t2988-t7937))./4.0;
t12294 = t9185.*(t3452-t4730+t5359+t9.*(t71-t391).*6.1597e-2+t17.*(t426-t581)).*(-1.0./4.0);
t12295 = (t3249.*t11969)./4.0;
t12301 = (t9185.*(t3452-t4730+t5359+t9.*(t71-t391).*6.1597e-2+t17.*(t426-t581)))./4.0;
t12314 = (t8742.*t9828)./4.0;
t12315 = (t8742.*t9830)./4.0;
t12318 = (t8256.*t10164)./4.0;
t12320 = -t12311;
t12321 = -t12312;
t12326 = (t5634.*t11344)./4.0;
t12334 = (t8285.*t10164)./4.0;
t12345 = -t12341;
t12349 = t9103+t9559;
t12350 = -t12344;
t12351 = -t12346;
t12356 = (t8191.*t10240)./4.0;
t12373 = (t10469.*(t2056+t2203+t2351+t3433+t3503+t16.*t389.*(1.1e+1./1.25e+2)))./2.0;
t12375 = (t7799.*t10468)./2.0;
t12384 = t8460.*(t1987-t2621+t3452-t4730+t5359+t9.*(t71-t391).*6.1597e-2+t17.*(t426-t581)).*(-1.0./4.0);
t12389 = (t8460.*(t1987-t2621+t3452-t4730+t5359+t9.*(t71-t391).*6.1597e-2+t17.*(t426-t581)))./4.0;
t12391 = (t7940.*t10469)./2.0;
t12394 = (t7949.*t10468)./2.0;
t12399 = (t8981.*t9887)./2.0;
t12400 = (t7982.*t10469)./2.0;
t12401 = (t8979.*t9896)./2.0;
t12405 = (t7987.*t10468)./2.0;
t12433 = t16.*t8227.*(t6452-t8229).*(-4.1663875e-1);
t12436 = (t6872.*t10974)./4.0;
t12443 = t6884.*(t8219-t8226).*(-1.0./4.0);
t12447 = t7822.*(t6801-t8594).*(-1.0./4.0);
t12451 = (t7822.*(t6801-t8594))./4.0;
t12455 = t7128.*(t1589-t2213+t3195-t4346+t4355+t4748.*7.35522e-1+t2772.*(t71-t391)+t2775.*(t71-t391)).*(-1.0./2.0);
t12456 = t7128.*(t1589-t2213+t3195-t4346+t4355+t4748.*7.35522e-1+t2772.*(t71-t391)+t2775.*(t71-t391)).*(-1.0./4.0);
t12457 = t7130.*(t1589-t2213+t3195-t4346+t4355+t4748.*7.35522e-1+t2772.*(t71-t391)+t2775.*(t71-t391)).*(-1.0./4.0);
t12458 = (t7128.*(t1589-t2213+t3195-t4346+t4355+t4748.*7.35522e-1+t2772.*(t71-t391)+t2775.*(t71-t391)))./2.0;
t12459 = (t7128.*(t1589-t2213+t3195-t4346+t4355+t4748.*7.35522e-1+t2772.*(t71-t391)+t2775.*(t71-t391)))./4.0;
t12461 = t7875.*(t6801-t8594).*(-1.0./4.0);
t12462 = (t7130.*(t1589-t2213+t3195-t4346+t4355+t4748.*7.35522e-1+t2772.*(t71-t391)+t2775.*(t71-t391)))./4.0;
t12466 = t12369.*(-7.35522e-1);
t12469 = t12369.*7.35522e-1;
t12474 = -t12472;
t12479 = t6302.*(t8582-t8586).*(-1.0./4.0);
t12482 = -t12480;
t12490 = t7336.*(t1589-t2213+t3195-t4346+t4355+t4748.*7.35522e-1+t2772.*(t71-t391)+t2775.*(t71-t391)).*(-1.0./4.0);
t12493 = (t7336.*(t1589-t2213+t3195-t4346+t4355+t4748.*7.35522e-1+t2772.*(t71-t391)+t2775.*(t71-t391)))./4.0;
t12540 = t12369.*(-3.867742437e-3);
t12543 = t12369.*3.867742437e-3;
t12545 = (t8227.*(t8646-t8.*(t30.*(t2425-t2468)+t68.*(t2425-t2468)).*1.666555))./4.0;
t12556 = t7654.*(t1589-t2213+t3195-t4346+t4355+t4748.*7.35522e-1+t2772.*(t71-t391)+t2775.*(t71-t391)).*(-1.0./2.0);
t12560 = (t7654.*(t1589-t2213+t3195-t4346+t4355+t4748.*7.35522e-1+t2772.*(t71-t391)+t2775.*(t71-t391)))./2.0;
t12574 = t9048.*(t1987-t2621+t3452-t4730+t5359+t9.*(t71-t391).*6.1597e-2+t17.*(t426-t581)).*(-1.0./4.0);
t12576 = (t9212.*t9967)./4.0;
t12577 = (t9213.*t9967)./4.0;
t12583 = (t9048.*(t1987-t2621+t3452-t4730+t5359+t9.*(t71-t391).*6.1597e-2+t17.*(t426-t581)))./4.0;
t12585 = ((t3085-t3419-t3773+t5128+t17.*(t208-t427).*7.35522e-1).*(t1987-t2621+t3452-t4730+t5359+t9.*(t71-t391).*6.1597e-2+t17.*(t426-t581)))./4.0;
t12614 = -t12609;
t12625 = (t8741.*t10501)./4.0;
t12634 = t8063.*(t1589-t2213+t3195-t4346+t4355+t4748.*7.35522e-1+t2772.*(t71-t391)+t2775.*(t71-t391)).*(-1.0./4.0);
t12637 = t10111.*(t249-t391.*(1.1e+1./1.25e+2)-t1912.*4.252e-3+t3505+t5357+t693.*(t71-t391)+t784.*(t71-t391)).*(-1.0./4.0);
t12639 = t7079.*(t8589-t8592).*(-1.0./4.0);
t12644 = (t7079.*(t8589-t8592))./4.0;
t12648 = -t12646;
t12655 = (t8256.*t10871)./4.0;
t12662 = (t5699.*t11969)./4.0;
t12671 = (t8999.*t10468)./2.0;
t12679 = (t9209.*t10164)./4.0;
t12681 = (t9001.*t10469)./2.0;
t12683 = t8979.*(t2740+t3849+t3968+t3972-t5255+t17.*(t260+t468+t570+t2298).*7.35522e-1).*(-1.0./4.0);
t12686 = (t10164.*(t2810+t2988-t7937))./4.0;
t12688 = t8981.*(-t3823+t3970+t5243+t9.*(t260+t468+t570+t2298).*7.35522e-1+t972.*(t71-t391)+t2777.*(t71-t391)).*(-1.0./4.0);
t12703 = (t9236.*t10164)./4.0;
t12706 = -t12697;
t12709 = -t12700;
t12728 = (t9278.*t10164)./4.0;
t12747 = -t12742;
t12758 = t9361.*(t1987-t2621+t3452-t4730+t5359+t9.*(t71-t391).*6.1597e-2+t17.*(t426-t581)).*(-1.0./4.0);
t12761 = -t12759;
t12764 = t10240.*(t249-t391.*(1.1e+1./1.25e+2)-t1912.*4.252e-3+t3505+t5357+t693.*(t71-t391)+t784.*(t71-t391)).*(-1.0./2.0);
t12768 = (t10240.*(t249-t391.*(1.1e+1./1.25e+2)-t1912.*4.252e-3+t3505+t5357+t693.*(t71-t391)+t784.*(t71-t391)))./2.0;
t12772 = t8433.*(t1589-t2213+t3195-t4346+t4355+t4748.*7.35522e-1+t2772.*(t71-t391)+t2775.*(t71-t391)).*(-1.0./2.0);
t12775 = (t8433.*(t1589-t2213+t3195-t4346+t4355+t4748.*7.35522e-1+t2772.*(t71-t391)+t2775.*(t71-t391)))./2.0;
t12813 = t9537.*(t1987-t2621+t3452-t4730+t5359+t9.*(t71-t391).*6.1597e-2+t17.*(t426-t581)).*(-1.0./4.0);
t12818 = (t9537.*(t1987-t2621+t3452-t4730+t5359+t9.*(t71-t391).*6.1597e-2+t17.*(t426-t581)))./4.0;
t12823 = t10468.*(t824+t2543+t2699+t2707-t4767+t17.*(t260+t468+t570+t2298)).*(-1.0./4.0);
t12824 = t10469.*(-t2550+t2696+t2698+t4771+t9.*(t260+t468+t570+t2298)+t147.*(t71-t391)).*(-1.0./4.0);
t12833 = (t8979.*t10753)./4.0;
t12834 = (t9187.*t10468)./4.0;
t12841 = t8628.*(t1589-t2213+t3195-t4346+t4355+t4748.*7.35522e-1+t2772.*(t71-t391)+t2775.*(t71-t391)).*(-1.0./2.0);
t12848 = (t9197.*t10469)./4.0;
t12849 = (t8981.*t10763)./4.0;
t12871 = (t9233.*t10469)./4.0;
t12878 = (t8979.*t10787)./4.0;
t12884 = (t9252.*t10468)./4.0;
t12886 = t8693.*(t1589-t2213+t3195-t4346+t4355+t4748.*7.35522e-1+t2772.*(t71-t391)+t2775.*(t71-t391)).*(-1.0./2.0);
t12889 = (t8693.*(t1589-t2213+t3195-t4346+t4355+t4748.*7.35522e-1+t2772.*(t71-t391)+t2775.*(t71-t391)))./2.0;
t12899 = t10469.*(t3452-t4730+t5359+t9.*(t71-t391).*6.1597e-2+t17.*(t426-t581)).*(-1.0./4.0);
t12901 = -t12897;
t12902 = (t10469.*(t3452-t4730+t5359+t9.*(t71-t391).*6.1597e-2+t17.*(t426-t581)))./4.0;
t12934 = (t6589.*t11969)./4.0;
t12960 = t10182.*(-t3045-t3218+t3458+t3539+t3878+t8.*(t260+t468+t570+t2298).*1.666555).*(-1.0./4.0);
t12965 = (t10182.*(-t3045-t3218+t3458+t3539+t3878+t8.*(t260+t468+t570+t2298).*1.666555))./4.0;
t12976 = t8.*t12696.*4.38178973375e-3;
t12982 = t8191.*(t8582-t8586).*(-1.0./4.0);
t12986 = (t8191.*(t8582-t8586))./4.0;
t12992 = t8227.*(t8589-t8592).*(-1.0./4.0);
t13000 = t9896.*(t1987-t2621+t3452-t4730+t5359+t9.*(t71-t391).*6.1597e-2+t17.*(t426-t581)).*(-1.0./4.0);
t13005 = t8982+t10948;
t13007 = (t9896.*(t1987-t2621+t3452-t4730+t5359+t9.*(t71-t391).*6.1597e-2+t17.*(t426-t581)))./4.0;
t13013 = t8998+t10947;
t13039 = -t13035;
t13074 = (t9967.*t10164)./4.0;
t13080 = t9967.*(t6452-t8229).*(-1.0./4.0);
t13085 = (t9967.*(t6452-t8229))./4.0;
t13108 = (t4900.*t12564)./4.0;
t13118 = (t4939.*t12564)./4.0;
t13121 = t16.*t12860.*4.38178973375e-3;
t13124 = -t13119;
t13125 = -t13120;
t13131 = (t9112.*(t9253-t44.*(t4540+t5.*(t2425-t2468))))./4.0;
t13136 = (t9112.*t10974)./4.0;
t13143 = -t13138;
t13149 = t9196.*(t1589-t2213+t3195-t4346+t4355+t4748.*7.35522e-1+t2772.*(t71-t391)+t2775.*(t71-t391)).*(-1.0./2.0);
t13151 = t10863.*(t249-t391.*(1.1e+1./1.25e+2)-t1912.*4.252e-3+t3505+t5357+t693.*(t71-t391)+t784.*(t71-t391)).*(-1.0./2.0);
t13155 = -t13154;
t13157 = (t9278.*t10871)./4.0;
t13202 = (t5442.*t12564)./4.0;
t13203 = -t13201;
t13221 = (t7822.*t11969)./4.0;
t13231 = t8.*t13038.*4.38178973375e-3;
t13234 = -t13228;
t13288 = -t13284;
t13305 = ((t2740+t3849+t3968+t3972-t5255+t17.*(t260+t468+t570+t2298).*7.35522e-1).*(t1987-t2621+t3452-t4730+t5359+t9.*(t71-t391).*6.1597e-2+t17.*(t426-t581)))./2.0;
t13333 = t3032+t3415+t3593+t3873+t8149+t10095;
t13335 = t6884.*(t1292+t2073+t2694+t11671).*(-1.0./4.0);
t13339 = (t6884.*(t1292+t2073+t2694+t11671))./4.0;
t13344 = -t13337;
t13346 = -t13338;
t13370 = (t9253-t44.*(t4540+t5.*(t2425-t2468))).*(-t3045-t3218+t3458+t3539+t3878+t8.*(t260+t468+t570+t2298).*1.666555).*(-1.0./4.0);
t13376 = t3386+t3523+t3548+t9318+t9753;
t13381 = t10974.*(-t3045-t3218+t3458+t3539+t3878+t8.*(t260+t468+t570+t2298).*1.666555).*(-1.0./4.0);
t13385 = (t10974.*(-t3045-t3218+t3458+t3539+t3878+t8.*(t260+t468+t570+t2298).*1.666555))./4.0;
t13401 = ((t8582-t8586).*(t249-t391.*(1.1e+1./1.25e+2)-t1912.*4.252e-3+t3505+t5357+t693.*(t71-t391)+t784.*(t71-t391)))./4.0;
t13410 = (t6385.*t12564)./4.0;
t13414 = t10753.*(t1987-t2621+t3452-t4730+t5359+t9.*(t71-t391).*6.1597e-2+t17.*(t426-t581)).*(-1.0./2.0);
t13415 = (t10753.*(t1987-t2621+t3452-t4730+t5359+t9.*(t71-t391).*6.1597e-2+t17.*(t426-t581)))./2.0;
t13420 = (t9967.*t10871)./4.0;
t13437 = -t13436;
t13440 = t10787.*(t1987-t2621+t3452-t4730+t5359+t9.*(t71-t391).*6.1597e-2+t17.*(t426-t581)).*(-1.0./2.0);
t13444 = (t10787.*(t1987-t2621+t3452-t4730+t5359+t9.*(t71-t391).*6.1597e-2+t17.*(t426-t581)))./2.0;
t13451 = t16.*t13326.*2.62925e-3;
t13454 = -t13449;
t13463 = (t6046.*t12696)./4.0;
t13482 = t10441.*(t6806-t8574).*(-1.0./4.0);
t13518 = t9.*t13496;
t13519 = t17.*t13496;
t13563 = -t13560;
t13566 = t6811.*(t9.*(t16.*(t30.*(t2425-t2468)+t68.*(t2425-t2468))+t8.*(t7.*(t4650+t34.*(t2425-t2468))+t47.*(t2425-t2468))).*7.35522e-1+t17.*(t4654+t15.*(t4650+t34.*(t2425-t2468))).*7.35522e-1).*(-1.0./4.0);
t13571 = (t6811.*(t9.*(t16.*(t30.*(t2425-t2468)+t68.*(t2425-t2468))+t8.*(t7.*(t4650+t34.*(t2425-t2468))+t47.*(t2425-t2468))).*7.35522e-1+t17.*(t4654+t15.*(t4650+t34.*(t2425-t2468))).*7.35522e-1))./4.0;
t13584 = (t16.*(t6452-t8229).*(t1589-t2213+t3195-t4346+t4355+t4748.*7.35522e-1+t2772.*(t71-t391)+t2775.*(t71-t391)))./4.0;
t13591 = -t13585;
t13593 = (t6969.*t12564)./4.0;
t13594 = -t13590;
t13603 = ((t8315+t8.*(t30.*(t2425-t2468)+t68.*(t2425-t2468))).*(t1589-t2213+t3195-t4346+t4355+t4748.*7.35522e-1+t2772.*(t71-t391)+t2775.*(t71-t391)))./4.0;
t13619 = -t13613;
t13620 = -t13614;
t13623 = -t13618;
t13634 = (t7217.*t12564)./4.0;
t13635 = (t7822.*t12464)./4.0;
t13639 = (t9967.*t11266)./4.0;
t13654 = (t6884.*t12667)./4.0;
t13670 = (t4021.*t13326)./4.0;
t13674 = (t6872.*t12696)./4.0;
t13688 = (t3265.*t13416)./4.0;
t13700 = (t3360.*t13416)./4.0;
t13702 = -t13698;
t13722 = (t3771.*t13416)./4.0;
t13724 = t10858.*(t6806-t8574).*(-1.0./4.0);
t13729 = (t10858.*(t6806-t8574))./4.0;
t13734 = t8.*t13627.*2.62925e-3;
t13735 = t10871.*(t6801-t8594).*(-1.0./4.0);
t13740 = (t10871.*(t6801-t8594))./4.0;
t13742 = (t6046.*t13038)./4.0;
t13743 = (t7676.*t12564)./4.0;
t13747 = (t13273.*(t2904-t2927))./4.0;
t13766 = (t10164.*t11336)./4.0;
t13784 = (t10164.*t11344)./4.0;
t13791 = -t13780;
t13794 = (t7815.*t12564)./2.0;
t13795 = (t7815.*t12564)./4.0;
t13800 = ((t6801-t8594).*(t8963+t7.*(t5026+t5.*(t2959-t2967))))./4.0;
t13805 = ((t6806-t8574).*(t8963+t7.*(t5026+t5.*(t2959-t2967))))./4.0;
t13809 = -t13801;
t13812 = -t13806;
t13829 = -t13824;
t13835 = (t6884.*t12860)./4.0;
t13846 = (t4453.*t13416)./4.0;
t13851 = (t12564.*(t917-t1669+t2469+t2475+t3495+t3591))./4.0;
t13855 = (t5365.*t13273)./4.0;
t13871 = -t13869;
t13874 = (t5234.*t13326)./4.0;
t13876 = t2091+t2579+t13508;
t13879 = t2031+t2569+t9172+t11679;
t13885 = (t7822.*t12669)./4.0;
t13886 = (t9967.*t11720)./4.0;
t13949 = t11247.*(t6806-t8574).*(-1.0./4.0);
t13953 = t15.*t12564.*(t4542-t6448).*(-4.1663875e-1);
t13956 = t11266.*(t6801-t8594).*(-1.0./4.0);
t13959 = (t4024.*t13627)./4.0;
t13960 = t15.*t12564.*(t4542-t6448).*4.1663875e-1;
t13963 = (t11266.*(t6801-t8594))./4.0;
t13967 = t15.*t12564.*(t6460-t35.*(t2425-t2468)).*4.1663875e-1;
t13974 = t2038+t3531+t3538+t4196+t4218+t9316+t9749;
t13975 = (t5275.*t13416)./4.0;
t13978 = (t12564.*(t2433+t2449-t3048-t3102+t3223+t3232))./4.0;
t13982 = -t13980;
t13983 = ((t8219-t8226).*(t1589-t2213+t3195-t4346+t4355+t4748.*7.35522e-1+t2772.*(t71-t391)+t2775.*(t71-t391)))./4.0;
t13997 = -t13994;
t14005 = t9185.*(t8329+t17.*(t16.*(t30.*(t2425-t2468)+t68.*(t2425-t2468))+t8.*(t7.*(t4650+t34.*(t2425-t2468))+t47.*(t2425-t2468)))).*(-1.0./4.0);
t14006 = (t5523.*t13416)./4.0;
t14008 = (t9185.*(t8329+t17.*(t16.*(t30.*(t2425-t2468)+t68.*(t2425-t2468))+t8.*(t7.*(t4650+t34.*(t2425-t2468))+t47.*(t2425-t2468)))))./4.0;
t14009 = (t5518.*t13416)./4.0;
t14011 = (t5543.*t13416)./4.0;
t14017 = t3600+t3672+t13508;
t14019 = (t7822.*t12898)./4.0;
t14020 = (t8791.*t12564)./4.0;
t14024 = -t14022;
t14025 = t8227.*(t3116+t3486+t3963+t11671.*1.666555).*(-1.0./4.0);
t14027 = t12564.*(t5144-t6902).*(-1.0./4.0);
t14028 = (t12564.*(t5144-t6902))./4.0;
t14029 = (t8927.*t12564)./4.0;
t14038 = t11969.*(t6452-t8229).*(-1.0./4.0);
t14039 = (t11969.*(t6452-t8229))./4.0;
t14042 = (t13416.*(-t1272-t1479+t1647+t1848+t2236))./4.0;
t14048 = (t6193.*t13416)./2.0;
t14049 = (t6193.*t13416)./4.0;
t14069 = (t3421.*t13915)./4.0;
t14074 = t11720.*(t6801-t8594).*(-1.0./4.0);
t14077 = (t3489.*t13915)./4.0;
t14078 = (t9104.*t12564)./4.0;
t14080 = -t14073;
t14085 = (t10164.*t12042)./4.0;
t14089 = -t14087;
t14097 = -t14096;
t14102 = (t9746.*t12385)./4.0;
t14105 = (t6535.*t13416)./4.0;
t14106 = (t9967.*t12266)./4.0;
t14109 = (t9732.*t12396)./4.0;
t14110 = (t9733.*t12396)./4.0;
t14113 = t3458+t3878+t9471+t11856;
t14122 = (t9333.*t12564)./4.0;
t14125 = (t6654.*t13416)./4.0;
t14129 = (t10164.*t12163)./4.0;
t14150 = -t14148;
t14157 = -t14153;
t14160 = -t14154;
t14171 = (t9525.*t12564)./4.0;
t14174 = (t6970.*t13416)./4.0;
t14188 = (t7080.*t13416)./4.0;
t14191 = -t14189;
t14212 = t12053.*(t6806-t8574).*(-1.0./4.0);
t14214 = (t12053.*(t6806-t8574))./4.0;
t14223 = -t14221;
t14225 = (t9110.*t12860)./4.0;
t14227 = t4395+t4428+t9469+t11860;
t14230 = (t9727.*t12564)./4.0;
t14231 = (t9728.*t12564)./4.0;
t14247 = -t14244;
t14262 = (t5696.*t13915)./4.0;
t14268 = t12266.*(t6801-t8594).*(-1.0./4.0);
t14269 = (t12266.*(t6801-t8594))./4.0;
t14273 = (t8227.*t13326)./4.0;
t14276 = (t7875.*t13416)./4.0;
t14277 = (t9992.*t12564)./4.0;
t14279 = t287+t450+t2672+t2686+t3465+t3572+t9172+t11679;
t14282 = t12696.*(-t3045-t3218+t3458+t3539+t3878+t8.*(t260+t468+t570+t2298).*1.666555).*(-1.0./4.0);
t14284 = (t7116.*t13627)./4.0;
t14285 = (t9112.*t13038)./4.0;
t14286 = (t12696.*(-t3045-t3218+t3458+t3539+t3878+t8.*(t260+t468+t570+t2298).*1.666555))./4.0;
t14302 = (t8640.*t13273)./4.0;
t14306 = t15.*t13416.*(t4542-t6448).*(-1.0./4.0);
t14307 = (t15.*t13416.*(t4542-t6448))./4.0;
t14308 = (t15.*t13416.*(t6460-t35.*(t2425-t2468)))./4.0;
t14311 = (t8213.*t13416)./4.0;
t14312 = ((t9.*(t16.*(t30.*(t2425-t2468)+t68.*(t2425-t2468))+t8.*(t7.*(t4650+t34.*(t2425-t2468))+t47.*(t2425-t2468))).*7.35522e-1+t17.*(t4654+t15.*(t4650+t34.*(t2425-t2468))).*7.35522e-1).*(t1987-t2621+t3452-t4730+t5359+t9.*(t71-t391).*6.1597e-2+t17.*(t426-t581)))./4.0;
t14324 = t12385.*(t6806-t8574).*(-1.0./4.0);
t14327 = t13416.*(t4654+t15.*(t4650+t34.*(t2425-t2468))).*(-1.0./4.0);
t14328 = (t12385.*(t6806-t8574))./4.0;
t14329 = (t13416.*(t4654+t15.*(t4650+t34.*(t2425-t2468))))./4.0;
t14334 = t12396.*(t6806-t8574).*(-1.0./4.0);
t14337 = (t6302.*t13915)./4.0;
t14338 = (t12396.*(t6806-t8574))./4.0;
t14341 = t10164.*(t3129+t3384+t3574+t7846+t9332).*(-1.0./4.0);
t14342 = (t10164.*(t3129+t3384+t3574+t7846+t9332))./4.0;
t14350 = t3421.*(t4401+t4424+t9457-t11860).*(-1.0./4.0);
t14351 = (t3421.*(t4401+t4424+t9457-t11860))./4.0;
t14359 = (t9226.*(t2810+t2988-t12589))./4.0;
t14397 = -t14395;
t14420 = (t8227.*(t3098+t3211-t3221+t3678+t8102+t10798))./4.0;
t14422 = t13627.*(-t1476-t1540+t2091+t2165+t2579+t8.*(t260+t468+t570+t2298)).*(-1.0./4.0);
t14425 = t13038.*(-t3045-t3218+t3458+t3539+t3878+t8.*(t260+t468+t570+t2298).*1.666555).*(-1.0./4.0);
t14443 = t12564.*(t6801-t8594).*(-1.0./4.0);
t14459 = -t14457;
t14522 = t2268+t2514+t2542+t2570+t3634+t9877+t11951;
t14526 = t2246+t2494+t2548+t2617+t3636+t9879+t11970;
t14541 = t2049+t2112+t2138+t2147+t3245+t9561+t12360;
t14542 = t2043+t2168+t2188+t2223+t3242+t9560+t12369;
t14543 = t4896.*(t249-t391.*(1.1e+1./1.25e+2)-t1912.*4.252e-3+t3505+t13496+t693.*(t71-t391)+t784.*(t71-t391)).*(-1.0./4.0);
t14544 = (t4896.*(t249-t391.*(1.1e+1./1.25e+2)-t1912.*4.252e-3+t3505+t13496+t693.*(t71-t391)+t784.*(t71-t391)))./4.0;
t14547 = (t9212.*t13416)./4.0;
t14548 = (t9213.*t13416)./4.0;
t14549 = t4938.*(t249-t391.*(1.1e+1./1.25e+2)-t1912.*4.252e-3+t3505+t13496+t693.*(t71-t391)+t784.*(t71-t391)).*(-1.0./4.0);
t14554 = (t2889-t2921).*(t249-t391.*(1.1e+1./1.25e+2)-t1912.*4.252e-3+t3505+t13496+t693.*(t71-t391)+t784.*(t71-t391)).*(-1.0./4.0);
t14555 = (t4938.*(t249-t391.*(1.1e+1./1.25e+2)-t1912.*4.252e-3+t3505+t13496+t693.*(t71-t391)+t784.*(t71-t391)))./4.0;
t14557 = ((t2889-t2921).*(t249-t391.*(1.1e+1./1.25e+2)-t1912.*4.252e-3+t3505+t13496+t693.*(t71-t391)+t784.*(t71-t391)))./4.0;
t14568 = -t14567;
t14571 = (t11344.*t12385)./2.0;
t14580 = t5696.*(t4401+t4424+t9457-t11860).*(-1.0./4.0);
t14602 = (t10164.*(t2810+t2988-t12589))./4.0;
t14611 = (t10164.*t13140)./4.0;
t14642 = t6302.*(t4401+t4424+t9457-t11860).*(-1.0./4.0);
t14644 = t9.*(t2148+t2513+t2649+t2661+t3582+t11950+t17.*(t258+t2289+t5392+t7559)).*(-1.13264871585e-2);
t14647 = t9.*(t2148+t2513+t2649+t2661+t3582+t11950+t17.*(t258+t2289+t5392+t7559)).*1.13264871585e-2;
t14660 = -t14657;
t14677 = t12564.*(t9125+t7.*(t5026+t5.*(t2959-t2967)).*1.666555).*(-1.0./2.0);
t14681 = (t12564.*(t9125+t7.*(t5026+t5.*(t2959-t2967)).*1.666555))./2.0;
t14682 = (t10141.*t13273)./4.0;
t14692 = t12866.*(t1589-t2213+t3195-t4346+t4355+t4748.*7.35522e-1+t2772.*(t71-t391)+t2775.*(t71-t391)).*(-1.0./4.0);
t14694 = (t12866.*(t1589-t2213+t3195-t4346+t4355+t4748.*7.35522e-1+t2772.*(t71-t391)+t2775.*(t71-t391)))./4.0;
t14695 = t6104.*(t249-t391.*(1.1e+1./1.25e+2)-t1912.*4.252e-3+t3505+t13496+t693.*(t71-t391)+t784.*(t71-t391)).*(-1.0./4.0);
t14696 = (t6104.*(t249-t391.*(1.1e+1./1.25e+2)-t1912.*4.252e-3+t3505+t13496+t693.*(t71-t391)+t784.*(t71-t391)))./4.0;
t14722 = t6304.*(t249-t391.*(1.1e+1./1.25e+2)-t1912.*4.252e-3+t3505+t13496+t693.*(t71-t391)+t784.*(t71-t391)).*(-1.0./4.0);
t14751 = (t10164.*t13416)./4.0;
t14755 = t13416.*(t6452-t8229).*(-1.0./4.0);
t14772 = t702+t2550+t2675+t2717+t11668+t11678;
t14785 = -t14781;
t14786 = -t14782;
t14804 = -t14800;
t14808 = t6966.*(t249-t391.*(1.1e+1./1.25e+2)-t1912.*4.252e-3+t3505+t13496+t693.*(t71-t391)+t784.*(t71-t391)).*(-1.0./4.0);
t14813 = (t6966.*(t249-t391.*(1.1e+1./1.25e+2)-t1912.*4.252e-3+t3505+t13496+t693.*(t71-t391)+t784.*(t71-t391)))./4.0;
t14835 = t13150.*(t1589-t2213+t3195-t4346+t4355+t4748.*7.35522e-1+t2772.*(t71-t391)+t2775.*(t71-t391)).*(-1.0./4.0);
t14839 = t13915.*(t249-t391.*(1.1e+1./1.25e+2)-t1912.*4.252e-3+t3505+t5357+t693.*(t71-t391)+t784.*(t71-t391)).*(-1.0./4.0);
t14852 = t7215.*(t249-t391.*(1.1e+1./1.25e+2)-t1912.*4.252e-3+t3505+t13496+t693.*(t71-t391)+t784.*(t71-t391)).*(-1.0./4.0);
t14854 = (t7215.*(t249-t391.*(1.1e+1./1.25e+2)-t1912.*4.252e-3+t3505+t13496+t693.*(t71-t391)+t784.*(t71-t391)))./4.0;
t14855 = t5434.*(t2148+t2513+t2649+t2661+t3582+t11950+t17.*(t258+t2289+t5392+t7559)).*(-1.0./4.0);
t14856 = (t5434.*(t2148+t2513+t2649+t2661+t3582+t11950+t17.*(t258+t2289+t5392+t7559)))./4.0;
t14862 = ((t701-t775).*(t1589-t2213-t4346+t4355+t9454+t11863+t2772.*(t71-t391)+t2775.*(t71-t391)))./4.0;
t14869 = t3365.*(t1589-t2213-t4346+t4355+t9454+t11863+t2772.*(t71-t391)+t2775.*(t71-t391)).*(-1.0./4.0);
t14870 = (t11969.*t12564)./2.0;
t14871 = t3455.*(t1589-t2213-t4346+t4355+t9454+t11863+t2772.*(t71-t391)+t2775.*(t71-t391)).*(-1.0./4.0);
t14872 = (t3365.*(t1589-t2213-t4346+t4355+t9454+t11863+t2772.*(t71-t391)+t2775.*(t71-t391)))./4.0;
t14873 = (t3455.*(t1589-t2213-t4346+t4355+t9454+t11863+t2772.*(t71-t391)+t2775.*(t71-t391)))./4.0;
t14882 = t8191.*(t4401+t4424+t9457-t11860).*(-1.0./4.0);
t14891 = t13273.*(t1589-t2213+t3195-t4346+t4355+t4748.*7.35522e-1+t2772.*(t71-t391)+t2775.*(t71-t391)).*(-1.0./4.0);
t14894 = t3552+t3822+t3883+t3916+t4378+t10078+t12068;
t14895 = t9.*t14770.*1.13264871585e-2;
t14904 = t4152.*(t1589-t2213-t4346+t4355+t9454+t11863+t2772.*(t71-t391)+t2775.*(t71-t391)).*(-1.0./4.0);
t14907 = (t4152.*(t1589-t2213-t4346+t4355+t9454+t11863+t2772.*(t71-t391)+t2775.*(t71-t391)))./4.0;
t14924 = ((t3479-t3544+t2772.*(t48-t349)+t2775.*(t48-t349)).*(t249-t391.*(1.1e+1./1.25e+2)-t1912.*4.252e-3+t3505+t13496+t693.*(t71-t391)+t784.*(t71-t391)))./4.0;
t14928 = -t14926;
t14929 = t13313.*(t1589-t2213+t3195-t4346+t4355+t4748.*7.35522e-1+t2772.*(t71-t391)+t2775.*(t71-t391)).*(-1.0./4.0);
t14930 = -t14927;
t14940 = t7980.*(t249-t391.*(1.1e+1./1.25e+2)-t1912.*4.252e-3+t3505+t13496+t693.*(t71-t391)+t784.*(t71-t391)).*(-1.0./4.0);
t14942 = (t7980.*(t249-t391.*(1.1e+1./1.25e+2)-t1912.*4.252e-3+t3505+t13496+t693.*(t71-t391)+t784.*(t71-t391)))./4.0;
t14947 = ((t2752+t3814-t4385-t9.*t439.*3.127439544e-3).*(t249-t391.*(1.1e+1./1.25e+2)-t1912.*4.252e-3+t3505+t13496+t693.*(t71-t391)+t784.*(t71-t391)))./4.0;
t14970 = (t10871.*t13416)./2.0;
t14971 = t4964.*(t1589-t2213-t4346+t4355+t9454+t11863+t2772.*(t71-t391)+t2775.*(t71-t391)).*(-1.0./4.0);
t14976 = t13416.*(t8963+t7.*(t5026+t5.*(t2959-t2967))).*(-1.0./2.0);
t14977 = (t13416.*(t8963+t7.*(t5026+t5.*(t2959-t2967))))./2.0;
t14986 = t8497.*(t249-t391.*(1.1e+1./1.25e+2)-t1912.*4.252e-3+t3505+t13496+t693.*(t71-t391)+t784.*(t71-t391)).*(-1.0./4.0);
t14990 = (t8497.*(t249-t391.*(1.1e+1./1.25e+2)-t1912.*4.252e-3+t3505+t13496+t693.*(t71-t391)+t784.*(t71-t391)))./4.0;
t14997 = t5290.*(t1589-t2213-t4346+t4355+t9454+t11863+t2772.*(t71-t391)+t2775.*(t71-t391)).*(-1.0./4.0);
t15001 = t8547.*(t249-t391.*(1.1e+1./1.25e+2)-t1912.*4.252e-3+t3505+t13496+t693.*(t71-t391)+t784.*(t71-t391)).*(-1.0./4.0);
t15002 = (t5290.*(t1589-t2213-t4346+t4355+t9454+t11863+t2772.*(t71-t391)+t2775.*(t71-t391)))./4.0;
t15003 = (t8547.*(t249-t391.*(1.1e+1./1.25e+2)-t1912.*4.252e-3+t3505+t13496+t693.*(t71-t391)+t784.*(t71-t391)))./4.0;
t15021 = t5524.*(t1589-t2213-t4346+t4355+t9454+t11863+t2772.*(t71-t391)+t2775.*(t71-t391)).*(-1.0./4.0);
t15024 = (t5524.*(t1589-t2213-t4346+t4355+t9454+t11863+t2772.*(t71-t391)+t2775.*(t71-t391)))./4.0;
t15026 = t5552.*(t1589-t2213-t4346+t4355+t9454+t11863+t2772.*(t71-t391)+t2775.*(t71-t391)).*(-1.0./4.0);
t15028 = (t5552.*(t1589-t2213-t4346+t4355+t9454+t11863+t2772.*(t71-t391)+t2775.*(t71-t391)))./4.0;
t15063 = (t12464.*t12564)./2.0;
t15066 = (t11266.*t13416)./2.0;
t15088 = t2740+t3849+t3968+t3972+t11865+t11870;
t15098 = t6096.*(t1589-t2213-t4346+t4355+t9454+t11863+t2772.*(t71-t391)+t2775.*(t71-t391)).*(-1.0./4.0);
t15101 = ((t4401+t4424+t9457-t11860).*(t249-t391.*(1.1e+1./1.25e+2)-t1912.*4.252e-3+t3505+t5357+t693.*(t71-t391)+t784.*(t71-t391)))./4.0;
t15106 = (t6096.*(t1589-t2213-t4346+t4355+t9454+t11863+t2772.*(t71-t391)+t2775.*(t71-t391)))./4.0;
t15108 = t9028.*(t249-t391.*(1.1e+1./1.25e+2)-t1912.*4.252e-3+t3505+t13496+t693.*(t71-t391)+t784.*(t71-t391)).*(-1.0./4.0);
t15112 = (t9028.*(t249-t391.*(1.1e+1./1.25e+2)-t1912.*4.252e-3+t3505+t13496+t693.*(t71-t391)+t784.*(t71-t391)))./4.0;
t15115 = t6158.*(t1589-t2213-t4346+t4355+t9454+t11863+t2772.*(t71-t391)+t2775.*(t71-t391)).*(-1.0./4.0);
t15117 = (t6158.*(t1589-t2213-t4346+t4355+t9454+t11863+t2772.*(t71-t391)+t2775.*(t71-t391)))./4.0;
t15122 = ((-t2149+t2205+t693.*(t48-t349)+t784.*(t48-t349)).*(t1589-t2213-t4346+t4355+t9454+t11863+t2772.*(t71-t391)+t2775.*(t71-t391)))./4.0;
t15128 = t7796.*(t2148+t2513+t2649+t2661+t3582+t11950+t17.*(t258+t2289+t5392+t7559)).*(-1.0./4.0);
t15130 = (t7796.*(t2148+t2513+t2649+t2661+t3582+t11950+t17.*(t258+t2289+t5392+t7559)))./4.0;
t15131 = ((t624+t2511-t3502-t9.*t439.*4.252e-3).*(t1589-t2213-t4346+t4355+t9454+t11863+t2772.*(t71-t391)+t2775.*(t71-t391)))./4.0;
t15138 = -t15136;
t15141 = t17.*(-t3823+t3970+t11861+t8.*t11864+t972.*(t71-t391)+t2777.*(t71-t391)).*(-1.539925e-2);
t15168 = t9310.*(t249-t391.*(1.1e+1./1.25e+2)-t1912.*4.252e-3+t3505+t13496+t693.*(t71-t391)+t784.*(t71-t391)).*(-1.0./4.0);
t15186 = (t12564.*t12669)./2.0;
t15187 = (t11720.*t13416)./2.0;
t15194 = t9505.*(t249-t391.*(1.1e+1./1.25e+2)-t1912.*4.252e-3+t3505+t13496+t693.*(t71-t391)+t784.*(t71-t391)).*(-1.0./4.0);
t15196 = (t9505.*(t249-t391.*(1.1e+1./1.25e+2)-t1912.*4.252e-3+t3505+t13496+t693.*(t71-t391)+t784.*(t71-t391)))./4.0;
t15215 = t7128.*(t1589-t2213-t4346+t4355+t9454+t11863+t2772.*(t71-t391)+t2775.*(t71-t391)).*(-1.0./2.0);
t15216 = t7128.*(t1589-t2213-t4346+t4355+t9454+t11863+t2772.*(t71-t391)+t2775.*(t71-t391)).*(-1.0./4.0);
t15217 = t7130.*(t1589-t2213-t4346+t4355+t9454+t11863+t2772.*(t71-t391)+t2775.*(t71-t391)).*(-1.0./4.0);
t15218 = (t7128.*(t1589-t2213-t4346+t4355+t9454+t11863+t2772.*(t71-t391)+t2775.*(t71-t391)))./2.0;
t15219 = (t7128.*(t1589-t2213-t4346+t4355+t9454+t11863+t2772.*(t71-t391)+t2775.*(t71-t391)))./4.0;
t15220 = t17.*t15156.*1.539925e-2;
t15221 = t9.*t15155.*1.539925e-2;
t15228 = t7336.*(t1589-t2213-t4346+t4355+t9454+t11863+t2772.*(t71-t391)+t2775.*(t71-t391)).*(-1.0./4.0);
t15229 = (t7336.*(t1589-t2213-t4346+t4355+t9454+t11863+t2772.*(t71-t391)+t2775.*(t71-t391)))./4.0;
t15238 = (t12564.*t12898)./2.0;
t15251 = t7654.*(t1589-t2213-t4346+t4355+t9454+t11863+t2772.*(t71-t391)+t2775.*(t71-t391)).*(-1.0./4.0);
t15256 = (t7654.*(t1589-t2213-t4346+t4355+t9454+t11863+t2772.*(t71-t391)+t2775.*(t71-t391)))./4.0;
t15257 = ((t3625+t3660+t9166-t11658).*(t1589-t2213+t3195-t4346+t4355+t4748.*7.35522e-1+t2772.*(t71-t391)+t2775.*(t71-t391)))./4.0;
t15269 = (t3738.*t15155)./4.0;
t15270 = (t3743.*t15156)./4.0;
t15286 = t8063.*(t1589-t2213-t4346+t4355+t9454+t11863+t2772.*(t71-t391)+t2775.*(t71-t391)).*(-1.0./4.0);
t15287 = t10096.*(t249-t391.*(1.1e+1./1.25e+2)-t1912.*4.252e-3+t3505+t13496+t693.*(t71-t391)+t784.*(t71-t391)).*(-1.0./4.0);
t15292 = t10111.*(t249-t391.*(1.1e+1./1.25e+2)-t1912.*4.252e-3+t3505+t13496+t693.*(t71-t391)+t784.*(t71-t391)).*(-1.0./4.0);
t15321 = t9185.*(t2189+t2495+t2635+t2646+t3580+t9.*(t258+t2289+t5392+t7559)+t17.*(t7693+t9904)).*(-1.0./4.0);
t15325 = (t9185.*(t2189+t2495+t2635+t2646+t3580+t9.*(t258+t2289+t5392+t7559)+t17.*(t7693+t9904)))./4.0;
t15335 = (t7796.*t14770)./4.0;
t15349 = t5345.*(-t3823+t3970+t11861+t8.*t11864+t972.*(t71-t391)+t2777.*(t71-t391)).*(-1.0./4.0);
t15353 = (t5345.*(-t3823+t3970+t11861+t8.*t11864+t972.*(t71-t391)+t2777.*(t71-t391)))./4.0;
t15367 = t10240.*(t249-t391.*(1.1e+1./1.25e+2)-t1912.*4.252e-3+t3505+t13496+t693.*(t71-t391)+t784.*(t71-t391)).*(-1.0./4.0);
t15369 = t8433.*(t1589-t2213-t4346+t4355+t9454+t11863+t2772.*(t71-t391)+t2775.*(t71-t391)).*(-1.0./4.0);
t15370 = (t10240.*(t249-t391.*(1.1e+1./1.25e+2)-t1912.*4.252e-3+t3505+t13496+t693.*(t71-t391)+t784.*(t71-t391)))./4.0;
t15373 = (t12266.*t13416)./2.0;
t15381 = t8628.*(t1589-t2213-t4346+t4355+t9454+t11863+t2772.*(t71-t391)+t2775.*(t71-t391)).*(-1.0./4.0);
t15389 = t10398.*(t249-t391.*(1.1e+1./1.25e+2)-t1912.*4.252e-3+t3505+t13496+t693.*(t71-t391)+t784.*(t71-t391)).*(-1.0./4.0);
t15391 = t16.*(t6452-t8229).*(t249-t391.*(1.1e+1./1.25e+2)-t1912.*4.252e-3+t3505+t13496+t693.*(t71-t391)+t784.*(t71-t391)).*1.838805e-1;
t15396 = t8693.*(t1589-t2213-t4346+t4355+t9454+t11863+t2772.*(t71-t391)+t2775.*(t71-t391)).*(-1.0./4.0);
t15398 = (t8693.*(t1589-t2213-t4346+t4355+t9454+t11863+t2772.*(t71-t391)+t2775.*(t71-t391)))./4.0;
t15400 = (t5329.*t15155)./4.0;
t15401 = (t5345.*t15156)./4.0;
t15436 = (t8643-t8.*(t30.*(t2425-t2468)+t68.*(t2425-t2468)).*7.35522e-1).*(t249-t391.*(1.1e+1./1.25e+2)-t1912.*4.252e-3+t3505+t13496+t693.*(t71-t391)+t784.*(t71-t391)).*(-1.0./4.0);
t15439 = ((t8643-t8.*(t30.*(t2425-t2468)+t68.*(t2425-t2468)).*7.35522e-1).*(t249-t391.*(1.1e+1./1.25e+2)-t1912.*4.252e-3+t3505+t13496+t693.*(t71-t391)+t784.*(t71-t391)))./4.0;
t15444 = t9196.*(t1589-t2213-t4346+t4355+t9454+t11863+t2772.*(t71-t391)+t2775.*(t71-t391)).*(-1.0./4.0);
t15445 = t6761.*(-t3823+t3970+t11861+t8.*t11864+t972.*(t71-t391)+t2777.*(t71-t391)).*(-1.0./4.0);
t15446 = (t6761.*(-t3823+t3970+t11861+t8.*t11864+t972.*(t71-t391)+t2777.*(t71-t391)))./4.0;
t15447 = t10863.*(t249-t391.*(1.1e+1./1.25e+2)-t1912.*4.252e-3+t3505+t13496+t693.*(t71-t391)+t784.*(t71-t391)).*(-1.0./4.0);
t15449 = t2549+t2650+t3448+t11652+t13532;
t15460 = t9185.*(-t2550+t2696+t2698+t11659+t8.*t11672+t147.*(t71-t391)).*(-1.0./4.0);
t15461 = (t9185.*(-t2550+t2696+t2698+t11659+t8.*t11672+t147.*(t71-t391)))./4.0;
t15501 = t17.*(t3452+t11654+t9.*(t71-t391).*6.1597e-2+t17.*(t426-t581)+t9.*(t9166-t11658)).*(-1.13264871585e-2);
t15502 = t17.*(t3452+t11654+t9.*(t71-t391).*6.1597e-2+t17.*(t426-t581)+t9.*(t9166-t11658)).*1.13264871585e-2;
t15515 = ((t8582-t8586).*(t249-t391.*(1.1e+1./1.25e+2)-t1912.*4.252e-3+t3505+t13496+t693.*(t71-t391)+t784.*(t71-t391)))./4.0;
t15531 = (t16.*(t6452-t8229).*(t1589-t2213-t4346+t4355+t9454+t11863+t2772.*(t71-t391)+t2775.*(t71-t391)))./4.0;
t15533 = ((t8315+t8.*(t30.*(t2425-t2468)+t68.*(t2425-t2468))).*(t1589-t2213-t4346+t4355+t9454+t11863+t2772.*(t71-t391)+t2775.*(t71-t391)))./4.0;
t15535 = t3893+t3901+t4321+t11852+t13625;
t15550 = t8981.*(-t3823+t3970+t11861+t8.*t11864+t972.*(t71-t391)+t2777.*(t71-t391)).*(-1.0./4.0);
t15552 = (t8981.*(-t3823+t3970+t11861+t8.*t11864+t972.*(t71-t391)+t2777.*(t71-t391)))./4.0;
t15555 = t5433.*(t3452+t11654+t9.*(t71-t391).*6.1597e-2+t17.*(t426-t581)+t9.*(t9166-t11658)).*(-1.0./4.0);
t15557 = t17.*(t1987-t2621+t3452+t11654+t9.*(t71-t391).*6.1597e-2+t17.*(t426-t581)+t9.*(t9166-t11658)).*(-1.13264871585e-2);
t15558 = (t5433.*(t3452+t11654+t9.*(t71-t391).*6.1597e-2+t17.*(t426-t581)+t9.*(t9166-t11658)))./4.0;
t15560 = t17.*(t1987-t2621+t3452+t11654+t9.*(t71-t391).*6.1597e-2+t17.*(t426-t581)+t9.*(t9166-t11658)).*1.13264871585e-2;
t15562 = t17.*(t4324+t11855+t9.*(t71-t391).*4.5305948634e-2+t17.*(t426-t581).*7.35522e-1+t9.*(t9166-t11658).*7.35522e-1).*(-1.539925e-2);
t15564 = t17.*(t4324+t11855+t9.*(t71-t391).*4.5305948634e-2+t17.*(t426-t581).*7.35522e-1+t9.*(t9166-t11658).*7.35522e-1).*1.539925e-2;
t15580 = (t10468.*t14770)./4.0;
t15585 = t10469.*(-t2550+t2696+t2698+t11659+t8.*t11672+t147.*(t71-t391)).*(-1.0./4.0);
t15586 = (t10469.*(-t2550+t2696+t2698+t11659+t8.*t11672+t147.*(t71-t391)))./4.0;
t15589 = (t8979.*t15155)./4.0;
t15590 = (t10468.*t14821)./4.0;
t15591 = (t10469.*t14823)./4.0;
t15592 = (t8981.*t15156)./4.0;
t15601 = t4298.*(t1987-t2621+t3452+t11654+t9.*(t71-t391).*6.1597e-2+t17.*(t426-t581)+t9.*(t9166-t11658)).*(-1.0./4.0);
t15602 = (t4298.*(t1987-t2621+t3452+t11654+t9.*(t71-t391).*6.1597e-2+t17.*(t426-t581)+t9.*(t9166-t11658)))./4.0;
t15609 = t3743.*(t4324+t11855+t9.*(t71-t391).*4.5305948634e-2+t17.*(t426-t581).*7.35522e-1+t9.*(t9166-t11658).*7.35522e-1).*(-1.0./4.0);
t15610 = (t3743.*(t4324+t11855+t9.*(t71-t391).*4.5305948634e-2+t17.*(t426-t581).*7.35522e-1+t9.*(t9166-t11658).*7.35522e-1))./4.0;
t15614 = ((t8219-t8226).*(t1589-t2213-t4346+t4355+t9454+t11863+t2772.*(t71-t391)+t2775.*(t71-t391)))./4.0;
t15620 = t5449.*(t1987-t2621+t3452+t11654+t9.*(t71-t391).*6.1597e-2+t17.*(t426-t581)+t9.*(t9166-t11658)).*(-1.0./4.0);
t15621 = (t5449.*(t1987-t2621+t3452+t11654+t9.*(t71-t391).*6.1597e-2+t17.*(t426-t581)+t9.*(t9166-t11658)))./4.0;
t15646 = t5345.*(t4324+t11855+t9.*(t71-t391).*4.5305948634e-2+t17.*(t426-t581).*7.35522e-1+t9.*(t9166-t11658).*7.35522e-1).*(-1.0./4.0);
t15648 = (t5345.*(t4324+t11855+t9.*(t71-t391).*4.5305948634e-2+t17.*(t426-t581).*7.35522e-1+t9.*(t9166-t11658).*7.35522e-1))./4.0;
t15657 = t7797.*(t3452+t11654+t9.*(t71-t391).*6.1597e-2+t17.*(t426-t581)+t9.*(t9166-t11658)).*(-1.0./4.0);
t15658 = (t7797.*(t3452+t11654+t9.*(t71-t391).*6.1597e-2+t17.*(t426-t581)+t9.*(t9166-t11658)))./4.0;
t15660 = t6397.*(t1987-t2621+t3452+t11654+t9.*(t71-t391).*6.1597e-2+t17.*(t426-t581)+t9.*(t9166-t11658)).*(-1.0./4.0);
t15663 = t17.*(t3418-t3879+t4324+t11855+t9.*(t71-t391).*4.5305948634e-2+t17.*(t426-t581).*7.35522e-1+t9.*(t9166-t11658).*7.35522e-1).*(-1.539925e-2);
t15665 = t17.*(t3418-t3879+t4324+t11855+t9.*(t71-t391).*4.5305948634e-2+t17.*(t426-t581).*7.35522e-1+t9.*(t9166-t11658).*7.35522e-1).*1.539925e-2;
t15670 = t2044.*(t3418-t3879+t4324+t11855+t9.*(t71-t391).*4.5305948634e-2+t17.*(t426-t581).*7.35522e-1+t9.*(t9166-t11658).*7.35522e-1).*(-1.0./4.0);
t15672 = (t2044.*(t3418-t3879+t4324+t11855+t9.*(t71-t391).*4.5305948634e-2+t17.*(t426-t581).*7.35522e-1+t9.*(t9166-t11658).*7.35522e-1))./4.0;
t15678 = t15155.*(t1987-t2621+t3452-t4730+t5359+t9.*(t71-t391).*6.1597e-2+t17.*(t426-t581)).*(-1.0./4.0);
t15680 = (t15155.*(t1987-t2621+t3452-t4730+t5359+t9.*(t71-t391).*6.1597e-2+t17.*(t426-t581)))./4.0;
t15683 = t6780.*(t1987-t2621+t3452+t11654+t9.*(t71-t391).*6.1597e-2+t17.*(t426-t581)+t9.*(t9166-t11658)).*(-1.0./4.0);
t15684 = (t6780.*(t1987-t2621+t3452+t11654+t9.*(t71-t391).*6.1597e-2+t17.*(t426-t581)+t9.*(t9166-t11658)))./4.0;
t15689 = t3763.*(t3418-t3879+t4324+t11855+t9.*(t71-t391).*4.5305948634e-2+t17.*(t426-t581).*7.35522e-1+t9.*(t9166-t11658).*7.35522e-1).*(-1.0./4.0);
t15691 = (t3763.*(t3418-t3879+t4324+t11855+t9.*(t71-t391).*4.5305948634e-2+t17.*(t426-t581).*7.35522e-1+t9.*(t9166-t11658).*7.35522e-1))./4.0;
t15692 = t6761.*(t4324+t11855+t9.*(t71-t391).*4.5305948634e-2+t17.*(t426-t581).*7.35522e-1+t9.*(t9166-t11658).*7.35522e-1).*(-1.0./4.0);
t15693 = (t6761.*(t4324+t11855+t9.*(t71-t391).*4.5305948634e-2+t17.*(t426-t581).*7.35522e-1+t9.*(t9166-t11658).*7.35522e-1))./4.0;
t15701 = t7538.*(t1987-t2621+t3452+t11654+t9.*(t71-t391).*6.1597e-2+t17.*(t426-t581)+t9.*(t9166-t11658)).*(-1.0./4.0);
t15703 = (t7538.*(t1987-t2621+t3452+t11654+t9.*(t71-t391).*6.1597e-2+t17.*(t426-t581)+t9.*(t9166-t11658)))./4.0;
t15704 = t4474.*(t3418-t3879+t4324+t11855+t9.*(t71-t391).*4.5305948634e-2+t17.*(t426-t581).*7.35522e-1+t9.*(t9166-t11658).*7.35522e-1).*(-1.0./4.0);
t15713 = t4798.*(t3418-t3879+t4324+t11855+t9.*(t71-t391).*4.5305948634e-2+t17.*(t426-t581).*7.35522e-1+t9.*(t9166-t11658).*7.35522e-1).*(-1.0./4.0);
t15714 = (t4798.*(t3418-t3879+t4324+t11855+t9.*(t71-t391).*4.5305948634e-2+t17.*(t426-t581).*7.35522e-1+t9.*(t9166-t11658).*7.35522e-1))./4.0;
t15715 = t7828.*(t1987-t2621+t3452+t11654+t9.*(t71-t391).*6.1597e-2+t17.*(t426-t581)+t9.*(t9166-t11658)).*(-1.0./4.0);
t15717 = (t7828.*(t1987-t2621+t3452+t11654+t9.*(t71-t391).*6.1597e-2+t17.*(t426-t581)+t9.*(t9166-t11658)))./4.0;
t15720 = t7913.*(t1987-t2621+t3452+t11654+t9.*(t71-t391).*6.1597e-2+t17.*(t426-t581)+t9.*(t9166-t11658)).*(-1.0./4.0);
t15721 = (t7913.*(t1987-t2621+t3452+t11654+t9.*(t71-t391).*6.1597e-2+t17.*(t426-t581)+t9.*(t9166-t11658)))./4.0;
t15727 = t5213.*(t3418-t3879+t4324+t11855+t9.*(t71-t391).*4.5305948634e-2+t17.*(t426-t581).*7.35522e-1+t9.*(t9166-t11658).*7.35522e-1).*(-1.0./4.0);
t15729 = (t5213.*(t3418-t3879+t4324+t11855+t9.*(t71-t391).*4.5305948634e-2+t17.*(t426-t581).*7.35522e-1+t9.*(t9166-t11658).*7.35522e-1))./4.0;
t15730 = t9185.*(t3452+t11654+t9.*(t71-t391).*6.1597e-2+t17.*(t426-t581)+t9.*(t9166-t11658)).*(-1.0./4.0);
t15732 = (t9185.*(t3452+t11654+t9.*(t71-t391).*6.1597e-2+t17.*(t426-t581)+t9.*(t9166-t11658)))./4.0;
t15742 = t8460.*(t1987-t2621+t3452+t11654+t9.*(t71-t391).*6.1597e-2+t17.*(t426-t581)+t9.*(t9166-t11658)).*(-1.0./4.0);
t15744 = (t8460.*(t1987-t2621+t3452+t11654+t9.*(t71-t391).*6.1597e-2+t17.*(t426-t581)+t9.*(t9166-t11658)))./4.0;
t15749 = t5679.*(t3418-t3879+t4324+t11855+t9.*(t71-t391).*4.5305948634e-2+t17.*(t426-t581).*7.35522e-1+t9.*(t9166-t11658).*7.35522e-1).*(-1.0./4.0);
t15751 = (t5679.*(t3418-t3879+t4324+t11855+t9.*(t71-t391).*4.5305948634e-2+t17.*(t426-t581).*7.35522e-1+t9.*(t9166-t11658).*7.35522e-1))./4.0;
t15760 = t5782.*(t3418-t3879+t4324+t11855+t9.*(t71-t391).*4.5305948634e-2+t17.*(t426-t581).*7.35522e-1+t9.*(t9166-t11658).*7.35522e-1).*(-1.0./4.0);
t15761 = (t5782.*(t3418-t3879+t4324+t11855+t9.*(t71-t391).*4.5305948634e-2+t17.*(t426-t581).*7.35522e-1+t9.*(t9166-t11658).*7.35522e-1))./4.0;
t15762 = t6016.*(t3418-t3879+t4324+t11855+t9.*(t71-t391).*4.5305948634e-2+t17.*(t426-t581).*7.35522e-1+t9.*(t9166-t11658).*7.35522e-1).*(-1.0./4.0);
t15764 = (t6016.*(t3418-t3879+t4324+t11855+t9.*(t71-t391).*4.5305948634e-2+t17.*(t426-t581).*7.35522e-1+t9.*(t9166-t11658).*7.35522e-1))./4.0;
t15772 = t6540.*(t3418-t3879+t4324+t11855+t9.*(t71-t391).*4.5305948634e-2+t17.*(t426-t581).*7.35522e-1+t9.*(t9166-t11658).*7.35522e-1).*(-1.0./4.0);
t15773 = t9048.*(t1987-t2621+t3452+t11654+t9.*(t71-t391).*6.1597e-2+t17.*(t426-t581)+t9.*(t9166-t11658)).*(-1.0./4.0);
t15774 = (t6540.*(t3418-t3879+t4324+t11855+t9.*(t71-t391).*4.5305948634e-2+t17.*(t426-t581).*7.35522e-1+t9.*(t9166-t11658).*7.35522e-1))./4.0;
t15775 = (t9048.*(t1987-t2621+t3452+t11654+t9.*(t71-t391).*6.1597e-2+t17.*(t426-t581)+t9.*(t9166-t11658)))./4.0;
t15776 = ((t3085-t3419-t3773+t5128+t17.*(t208-t427).*7.35522e-1).*(t1987-t2621+t3452+t11654+t9.*(t71-t391).*6.1597e-2+t17.*(t426-t581)+t9.*(t9166-t11658)))./4.0;
t15779 = t8981.*(t4324+t11855+t9.*(t71-t391).*4.5305948634e-2+t17.*(t426-t581).*7.35522e-1+t9.*(t9166-t11658).*7.35522e-1).*(-1.0./4.0);
t15780 = (t8981.*(t4324+t11855+t9.*(t71-t391).*4.5305948634e-2+t17.*(t426-t581).*7.35522e-1+t9.*(t9166-t11658).*7.35522e-1))./4.0;
t15784 = t9361.*(t1987-t2621+t3452+t11654+t9.*(t71-t391).*6.1597e-2+t17.*(t426-t581)+t9.*(t9166-t11658)).*(-1.0./4.0);
t15785 = t13578.*(t249-t391.*(1.1e+1./1.25e+2)-t1912.*4.252e-3+t3505+t13496+t693.*(t71-t391)+t784.*(t71-t391)).*(-1.0./2.0);
t15789 = t9537.*(t1987-t2621+t3452+t11654+t9.*(t71-t391).*6.1597e-2+t17.*(t426-t581)+t9.*(t9166-t11658)).*(-1.0./4.0);
t15791 = (t9537.*(t1987-t2621+t3452+t11654+t9.*(t71-t391).*6.1597e-2+t17.*(t426-t581)+t9.*(t9166-t11658)))./4.0;
t15792 = ((t1468-t1988-t2498+t4565+t17.*(t208-t427)).*(t3418-t3879+t4324+t11855+t9.*(t71-t391).*4.5305948634e-2+t17.*(t426-t581).*7.35522e-1+t9.*(t9166-t11658).*7.35522e-1))./4.0;
t15793 = t12866.*(t1589-t2213-t4346+t4355+t9454+t11863+t2772.*(t71-t391)+t2775.*(t71-t391)).*(-1.0./2.0);
t15796 = t10469.*(t3452+t11654+t9.*(t71-t391).*6.1597e-2+t17.*(t426-t581)+t9.*(t9166-t11658)).*(-1.0./4.0);
t15797 = (t10469.*(t3452+t11654+t9.*(t71-t391).*6.1597e-2+t17.*(t426-t581)+t9.*(t9166-t11658)))./4.0;
t15800 = t7799.*(t3418-t3879+t4324+t11855+t9.*(t71-t391).*4.5305948634e-2+t17.*(t426-t581).*7.35522e-1+t9.*(t9166-t11658).*7.35522e-1).*(-1.0./4.0);
t15801 = (t7799.*(t3418-t3879+t4324+t11855+t9.*(t71-t391).*4.5305948634e-2+t17.*(t426-t581).*7.35522e-1+t9.*(t9166-t11658).*7.35522e-1))./4.0;
t15803 = t7949.*(t3418-t3879+t4324+t11855+t9.*(t71-t391).*4.5305948634e-2+t17.*(t426-t581).*7.35522e-1+t9.*(t9166-t11658).*7.35522e-1).*(-1.0./4.0);
t15806 = t9896.*(t1987-t2621+t3452+t11654+t9.*(t71-t391).*6.1597e-2+t17.*(t426-t581)+t9.*(t9166-t11658)).*(-1.0./4.0);
t15807 = t7987.*(t3418-t3879+t4324+t11855+t9.*(t71-t391).*4.5305948634e-2+t17.*(t426-t581).*7.35522e-1+t9.*(t9166-t11658).*7.35522e-1).*(-1.0./4.0);
t15815 = t13150.*(t1589-t2213-t4346+t4355+t9454+t11863+t2772.*(t71-t391)+t2775.*(t71-t391)).*(-1.0./2.0);
t15816 = t13915.*(t249-t391.*(1.1e+1./1.25e+2)-t1912.*4.252e-3+t3505+t13496+t693.*(t71-t391)+t784.*(t71-t391)).*(-1.0./2.0);
t15832 = t8999.*(t3418-t3879+t4324+t11855+t9.*(t71-t391).*4.5305948634e-2+t17.*(t426-t581).*7.35522e-1+t9.*(t9166-t11658).*7.35522e-1).*(-1.0./4.0);
t15834 = t13273.*(t1589-t2213-t4346+t4355+t9454+t11863+t2772.*(t71-t391)+t2775.*(t71-t391)).*(-1.0./2.0);
t15835 = (t13273.*(t1589-t2213-t4346+t4355+t9454+t11863+t2772.*(t71-t391)+t2775.*(t71-t391)))./2.0;
t15838 = ((t2740+t3849+t3968+t3972-t5255+t17.*(t260+t468+t570+t2298).*7.35522e-1).*(t1987-t2621+t3452+t11654+t9.*(t71-t391).*6.1597e-2+t17.*(t426-t581)+t9.*(t9166-t11658)))./4.0;
t15842 = t13313.*(t1589-t2213-t4346+t4355+t9454+t11863+t2772.*(t71-t391)+t2775.*(t71-t391)).*(-1.0./2.0);
t15843 = t14035.*(t249-t391.*(1.1e+1./1.25e+2)-t1912.*4.252e-3+t3505+t13496+t693.*(t71-t391)+t784.*(t71-t391)).*(-1.0./2.0);
t15844 = ((t824+t2543+t2699+t2707-t4767+t17.*(t260+t468+t570+t2298)).*(t3418-t3879+t4324+t11855+t9.*(t71-t391).*4.5305948634e-2+t17.*(t426-t581).*7.35522e-1+t9.*(t9166-t11658).*7.35522e-1))./4.0;
t15847 = t9187.*(t3418-t3879+t4324+t11855+t9.*(t71-t391).*4.5305948634e-2+t17.*(t426-t581).*7.35522e-1+t9.*(t9166-t11658).*7.35522e-1).*(-1.0./4.0);
t15848 = t10753.*(t1987-t2621+t3452+t11654+t9.*(t71-t391).*6.1597e-2+t17.*(t426-t581)+t9.*(t9166-t11658)).*(-1.0./4.0);
t15855 = t10787.*(t1987-t2621+t3452+t11654+t9.*(t71-t391).*6.1597e-2+t17.*(t426-t581)+t9.*(t9166-t11658)).*(-1.0./4.0);
t15856 = t9252.*(t3418-t3879+t4324+t11855+t9.*(t71-t391).*4.5305948634e-2+t17.*(t426-t581).*7.35522e-1+t9.*(t9166-t11658).*7.35522e-1).*(-1.0./4.0);
t15857 = (t10787.*(t1987-t2621+t3452+t11654+t9.*(t71-t391).*6.1597e-2+t17.*(t426-t581)+t9.*(t9166-t11658)))./4.0;
t15858 = (t9252.*(t3418-t3879+t4324+t11855+t9.*(t71-t391).*4.5305948634e-2+t17.*(t426-t581).*7.35522e-1+t9.*(t9166-t11658).*7.35522e-1))./4.0;
t15875 = ((t4401+t4424+t9457-t11860).*(t249-t391.*(1.1e+1./1.25e+2)-t1912.*4.252e-3+t3505+t13496+t693.*(t71-t391)+t784.*(t71-t391)))./2.0;
t15890 = ((t3625+t3660+t9166-t11658).*(t1589-t2213-t4346+t4355+t9454+t11863+t2772.*(t71-t391)+t2775.*(t71-t391)))./2.0;
